simulink model "RB_KAIROS_impControl_repulsive"  (R2020b)
settings: Solver=ode4  StartTime=0.0  StopTime=t_end  FixedStep=Ts  RelTol=1e-3
values from neighbouring files (symbols this model uses):
  am = 0.3    [RB_KAIROS_ImpControl_OpSpace_quat_2020b_safety_main.m]
  am_r = 0.3    [RB_KAIROS_ImpControl_OpSpace_quat_2020b_safety_main.m]
  Kc = diag(50*ones(6,1))    [RB_KAIROS_ImpControl_OpSpace_quat_2020b_safety_main.m]
  Kp = 2*[400;400;400;400;0;0;0]    [RB_KAIROS_ImpControl_OpSpace_quat_2020b_safety_main.m]
  Kv = [1000;1000;1000;[300;300;300;300;300;300;300]]    [RB_KAIROS_ImpControl_OpSpace_quat_2020b_safety_main.m]
  model_sample_time = 0.001    [RB_KAIROS_ImpControl_OpSpace_quat_2020b_safety_main.m]
  q_dot_0 = zeros(10,1)    [RB_KAIROS_ImpControl_OpSpace_quat_2020b_safety_main.m]
  T_i = K    [RB_KAIROS_ImpControl_OpSpace_quat_2020b_safety_main.m]
  tau_ext = [0 0 0 0 0 0 0 0 0 0 0]    [RB_KAIROS_ImpControl_OpSpace_quat_2020b_safety_main.m]
  v_SMU = 10    [RB_KAIROS_ImpControl_OpSpace_quat_2020b_safety_main.m]
  vm = 0.5    [RB_KAIROS_ImpControl_OpSpace_quat_2020b_safety_main.m]
  vm_r = 0.5    [RB_KAIROS_ImpControl_OpSpace_quat_2020b_safety_main.m]
undefined symbols (not defined in the file or in its folder): DiscIntNeverNeededParam, magnitude, q_0, T_f
libraries: simulink x4, utils x4, transformations_lib x3
(part 3 of 17)

== matlab function RB_KAIROS_impControl_repulsive/CONTROLLER /Kinematics and Dynamics/Dynamics - Configuration space/Arm Coriolis//Centrifugal Matrix  ==
  data: qv input; C output; qa input; qdv input; qda input
function C = get_C(qv,qa,qdv,qda)
%GET_C
%    C = GET_C(qv,qa,qdv,qda)

%    This function was generated by the Symbolic Math Toolbox version 8.6.
%    14-Feb-2023 12:26:28

phi = qv(3);
phid = qdv(3);
q1 = qa(1);
q2 = qa(2);
q3 = qa(3);
q4 = qa(4);
q5 = qa(5);
q6 = qa(6);
q7 = qa(7);
q1d = qda(1);
q2d = qda(2);
q3d = qda(3);
q4d = qda(4);
q5d = qda(5);
q6d = qda(6);
q7d = qda(7);
xd = qdv(1);
yd = qdv(2);
t2 = cos(phi);
t3 = cos(q1);
t4 = cos(q2);
t5 = cos(q3);
t6 = cos(q4);
t7 = cos(q5);
t8 = cos(q6);
t9 = cos(q7);
t10 = sin(phi);
t11 = sin(q1);
t12 = sin(q2);
t13 = sin(q3);
t14 = sin(q4);
t15 = sin(q5);
t16 = sin(q6);
t17 = sin(q7);
t18 = t4.^2;
t19 = t5.^2;
t20 = t6.^2;
t21 = t7.^2;
t22 = t8.^2;
t23 = t9.^2;
t24 = t12.^2;
t25 = t13.^2;
t26 = t14.^2;
t27 = t15.^2;
t28 = t16.^2;
t29 = t17.^2;
t30 = t4.*t6;
t31 = t5.*t7;
t32 = t6.*t8;
t33 = t7.*t9;
t34 = t4.*t14;
t35 = t6.*t12;
t36 = t5.*t15;
t37 = t7.*t13;
t38 = t6.*t16;
t39 = t8.*t14;
t40 = t7.*t17;
t41 = t9.*t15;
t42 = t12.*t14;
t43 = t13.*t15;
t44 = t14.*t16;
t45 = t15.*t17;
t46 = -t10;
t82 = t7.*(1.1e+1./1.25e+2);
t83 = t6.*(4.8e+1./1.25e+2);
t84 = t7.*(4.8e+1./1.25e+2);
t85 = t4.*(3.3e+1./4.0e+2);
t86 = t5.*(3.3e+1./4.0e+2);
t87 = t6.*(3.3e+1./4.0e+2);
t88 = t7.*(3.3e+1./4.0e+2);
t89 = t8.*(3.3e+1./4.0e+2);
t90 = t15.*(1.1e+1./1.25e+2);
t91 = t14.*(4.8e+1./1.25e+2);
t92 = t15.*(4.8e+1./1.25e+2);
t93 = t12.*(3.3e+1./4.0e+2);
t94 = t13.*(3.3e+1./4.0e+2);
t95 = t14.*(3.3e+1./4.0e+2);
t96 = t15.*(3.3e+1./4.0e+2);
t97 = t16.*(3.3e+1./4.0e+2);
t121 = t5.*(7.9e+1./2.5e+2);
t125 = t13.*(7.9e+1./2.5e+2);
t132 = t8.*t9.*(1.1e+1./1.25e+2);
t146 = t8.*t17.*(1.1e+1./1.25e+2);
t147 = t9.*t16.*(1.1e+1./1.25e+2);
t163 = t16.*t17.*(1.1e+1./1.25e+2);
t179 = t5.*t6.*(-3.3e+1./4.0e+2);
t180 = t7.*t16.*(-4.8e+1./1.25e+2);
t181 = t8.*t15.*(-4.8e+1./1.25e+2);
t188 = t4.*t13.*(-3.3e+1./4.0e+2);
t189 = t5.*t12.*(-3.3e+1./4.0e+2);
t191 = t5.*t14.*(-3.3e+1./4.0e+2);
t192 = t6.*t13.*(-3.3e+1./4.0e+2);
t197 = t12.*t13.*(-3.3e+1./4.0e+2);
t198 = t13.*t14.*(-3.3e+1./4.0e+2);
t199 = t4.*2.872e-2;
t200 = t4.*3.925e-3;
t201 = t12.*2.872e-2;
t202 = t12.*3.925e-3;
t203 = t4.*t5.*(-7.9e+1./2.5e+2);
t204 = t5.*t6.*(-7.9e+1./2.5e+2);
t212 = t5.*t14.*(-7.9e+1./2.5e+2);
t213 = t13.*t14.*(-7.9e+1./2.5e+2);
t215 = t6.*1.9552e-2;
t216 = t5.*1.0442e-1;
t217 = t6.*1.0442e-1;
t219 = t14.*1.9552e-2;
t221 = t13.*1.0442e-1;
t222 = t14.*1.0442e-1;
t270 = t4.*1.083e-2;
t271 = t4.*2.811e-2;
t272 = t5.*5.317e-2;
t273 = t6.*5.317e-2;
t275 = t12.*1.083e-2;
t276 = t12.*2.811e-2;
t277 = t13.*5.317e-2;
t278 = t14.*5.317e-2;
t337 = t5.*t14.*(-1.9552e-2);
t364 = t5.*t12.*(-5.317e-2);
t366 = t5.*t14.*(-5.317e-2);
t367 = t12.*t13.*(-5.317e-2);
t368 = t13.*t14.*(-5.317e-2);
t566 = t13.*3.7242e-2;
t567 = t7.*2.9474e-2;
t569 = t15.*2.9474e-2;
t576 = t5.*3.7242e-2;
t587 = t9.*1.2516e-2;
t589 = t17.*1.2516e-2;
t606 = t8.*4.815e-3;
t607 = t7.*3.5549e-2;
t608 = t16.*4.815e-3;
t609 = t15.*3.5549e-2;
t610 = t5.*1.01140545e-1;
t611 = t7.*1.01140545e-1;
t612 = t13.*1.01140545e-1;
t613 = t15.*1.01140545e-1;
t621 = t12.*t13.*(-3.7242e-2);
t625 = t14.*4.1065e-2;
t626 = t15.*4.1065e-2;
t627 = t12.*7.962e-3;
t628 = t8.*4.354e-3;
t629 = t4.*1.2805e-2;
t630 = t5.*1.2805e-2;
t631 = t16.*4.354e-3;
t632 = t12.*1.2805e-2;
t633 = t13.*1.2805e-2;
t634 = t5.*2.8323e-2;
t635 = t13.*2.8323e-2;
t636 = t6.*8.626999999999999e-3;
t637 = t7.*5.433e-3;
t638 = t14.*8.626999999999999e-3;
t639 = t15.*5.433e-3;
t640 = t6.*2.5853e-2;
t643 = t14.*2.5853e-2;
t644 = t4.*2.7518e-2;
t645 = t5.*2.7518e-2;
t647 = t5.*3.6155e-2;
t648 = t12.*2.7518e-2;
t649 = t13.*2.7518e-2;
t650 = t7.*6.0149e-2;
t651 = t8.*6.0149e-2;
t652 = t13.*3.6155e-2;
t653 = t4.*3.9252e-2;
t654 = t5.*3.9252e-2;
t659 = t15.*6.0149e-2;
t660 = t16.*6.0149e-2;
t661 = t4.*1.1396e-2;
t662 = t5.*1.1396e-2;
t663 = t12.*3.9252e-2;
t664 = t13.*3.9252e-2;
t669 = t12.*1.1396e-2;
t670 = t13.*1.1396e-2;
t671 = t5.*8.640999999999999e-3;
t672 = t6.*8.640999999999999e-3;
t677 = t7.*6.3995712e-1;
t678 = t6.*4.1065e-2;
t679 = t7.*4.1065e-2;
t680 = t13.*8.640999999999999e-3;
t681 = t14.*8.640999999999999e-3;
t684 = t4.*7.962e-3;
t685 = t15.*6.3995712e-1;
t686 = t8.*1.196e-3;
t687 = t9.*1.196e-3;
t689 = t17.*4.28e-4;
t690 = t6.*7.796e-3;
t692 = t8.*1.0517e-2;
t693 = t9.*1.0517e-2;
t694 = t7.*2.117e-3;
t695 = t16.*1.196e-3;
t696 = t17.*1.196e-3;
t697 = t14.*7.796e-3;
t698 = t7.*t8.*2.82440448e-1;
t700 = t16.*1.0517e-2;
t701 = t17.*1.0517e-2;
t703 = t15.*2.117e-3;
t704 = t6.*4.037e-3;
t705 = t7.*4.037e-3;
t706 = t7.*6.4725936e-2;
t707 = t4.*3.495e-3;
t708 = t5.*t6.*3.87398936e-1;
t710 = t7.*t16.*2.82440448e-1;
t714 = t14.*4.037e-3;
t715 = t15.*4.037e-3;
t717 = t15.*6.4725936e-2;
t719 = t12.*3.495e-3;
t720 = t5.*t14.*3.87398936e-1;
t723 = t15.*t16.*2.82440448e-1;
t725 = t7.*1.158e-3;
t726 = t8.*1.158e-3;
t730 = t13.*t14.*3.87398936e-1;
t732 = t15.*1.158e-3;
t733 = t16.*1.158e-3;
t734 = t5.*1.332e-3;
t735 = t6.*1.332e-3;
t740 = t9.*1.0027e-2;
t742 = t13.*1.332e-3;
t743 = t14.*1.332e-3;
t751 = t17.*1.0027e-2;
t762 = t6.*t7.*3.8437e-2;
t764 = t6.*t15.*3.8437e-2;
t765 = t7.*t14.*3.8437e-2;
t766 = t14.*t15.*3.8437e-2;
t768 = t8.*1.964e-3;
t769 = t6.*1.1953e-2;
t770 = t7.*1.1953e-2;
t772 = t16.*1.964e-3;
t773 = t4.*3.141e-3;
t774 = t8.*4.252e-3;
t775 = t9.*4.252e-3;
t776 = t14.*1.1953e-2;
t777 = t15.*1.1953e-2;
t781 = t12.*3.141e-3;
t782 = t5.*4.761e-3;
t783 = t16.*4.252e-3;
t784 = t17.*4.252e-3;
t788 = t13.*4.761e-3;
t789 = t7.*1.4117e-2;
t790 = t8.*1.4117e-2;
t795 = t15.*1.4117e-2;
t796 = t16.*1.4117e-2;
t798 = t9.*4.28e-4;
t801 = t16.*t17.*(-1.2516e-2);
t804 = t8.*6.0680565e-2;
t805 = t7.*3.41e-4;
t806 = t8.*3.41e-4;
t813 = t16.*6.0680565e-2;
t817 = t15.*3.41e-4;
t818 = t16.*3.41e-4;
t830 = t8.*t9.*6.1597e-2;
t832 = t6.*2.29e-4;
t833 = t7.*2.29e-4;
t843 = t8.*t17.*6.1597e-2;
t844 = t9.*t16.*6.1597e-2;
t846 = t14.*2.29e-4;
t847 = t15.*2.29e-4;
t857 = t16.*t17.*6.1597e-2;
t862 = t7.*t16.*(-4.815e-3);
t866 = t5.*t6.*2.7454e-2;
t867 = t5.*t6.*(-1.01140545e-1);
t871 = t14.*t15.*(-3.5549e-2);
t874 = t5.*t14.*2.7454e-2;
t875 = t6.*t13.*2.7454e-2;
t876 = t5.*t14.*(-1.01140545e-1);
t877 = t6.*t13.*(-1.01140545e-1);
t883 = t13.*t14.*2.7454e-2;
t890 = t8.*7.41e-4;
t891 = t9.*7.41e-4;
t905 = t16.*7.41e-4;
t906 = t17.*7.41e-4;
t957 = t16.*1.09e-4;
t971 = t8.*t17.*6.4725936e-2;
t972 = t9.*t16.*6.4725936e-2;
t977 = t7.*t16.*(-4.354e-3);
t982 = t16.*t17.*6.4725936e-2;
t995 = t12.*t13.*(-1.2805e-2);
t999 = t4.*t13.*(-2.8323e-2);
t1004 = t7.*1.374907875e-1;
t1005 = t8.*1.374907875e-1;
t1018 = t12.*t13.*(-2.8323e-2);
t1023 = t15.*1.374907875e-1;
t1024 = t16.*1.374907875e-1;
t1026 = t6.*t13.*(-8.626999999999999e-3);
t1041 = t6.*t15.*(-5.433e-3);
t1048 = t14.*t15.*(-5.433e-3);
t1051 = t5.*t6.*(-2.5853e-2);
t1052 = t5.*1.13377482;
t1057 = t13.*1.13377482;
t1078 = t7.*t14.*(-6.0149e-2);
t1082 = t4.*t5.*(-1.1396e-2);
t1100 = t12.*t13.*(-3.9252e-2);
t1115 = t7.*t16.*(-6.3995712e-1);
t1116 = t8.*t15.*(-6.3995712e-1);
t1126 = t5.*t14.*(-4.1065e-2);
t1133 = t12.*t13.*(-8.640999999999999e-3);
t1140 = t4.*2.960013375e-1;
t1161 = t8.*1.09e-4;
t1166 = t12.*2.960013375e-1;
t1176 = t8.*t9.*6.4725936e-2;
t1179 = t16.*t17.*(-1.0517e-2);
t1184 = t14.*t15.*(-2.117e-3);
t1186 = t6.*t13.*(-4.037e-3);
t1194 = t14.*t15.*(-4.037e-3);
t1227 = t14.*t15.*(-1.158e-3);
t1229 = t15.*t16.*(-1.158e-3);
t1231 = t4.*t13.*(-1.332e-3);
t1243 = t13.*t14.*(-1.332e-3);
t1284 = t7.*t8.*(-1.964e-3);
t1297 = t6.*t15.*(-1.1953e-2);
t1303 = t13.*t14.*(-1.1953e-2);
t1304 = t14.*t15.*(-1.1953e-2);
t1312 = t7.*t8.*(-1.4117e-2);
t1325 = t12.*t13.*(-4.761e-3);
t1326 = t8.*t15.*(-1.4117e-2);
t1330 = t8.*t9.*(-1.196e-3);
t1337 = t7.*t16.*(-1.196e-3);
t1338 = t16.*t17.*(-4.28e-4);
t1340 = t6.*t13.*(-7.796e-3);
t1345 = t8.*t15.*(-1.0517e-2);
t1347 = t8.*t17.*(-1.0517e-2);
t1357 = t15.*t16.*(-1.196e-3);
t1358 = t13.*t14.*(-7.796e-3);
t1386 = t6.*t13.*(-2.29e-4);
t1423 = t4.*t5.*2.49498e-1;
t1429 = t8.*t15.*(-7.41e-4);
t1442 = t4.*t13.*2.49498e-1;
t1443 = t5.*t12.*2.49498e-1;
t1446 = t16.*t17.*(-7.41e-4);
t1460 = t12.*t13.*2.49498e-1;
t1496 = t5.*t6.*2.960013375e-1;
t1526 = t5.*t14.*2.960013375e-1;
t1527 = t6.*t13.*2.960013375e-1;
t1557 = t13.*t14.*2.960013375e-1;
t1594 = t6.*t15.*(-3.41e-4);
t1628 = t5.*t6.*(-1.13377482);
t1640 = t13.*t14.*(-1.13377482);
t1679 = t4.*1.857971472e-2;
t1700 = t12.*1.857971472e-2;
t1707 = t8.*t15.*(-1.09e-4);
t1724 = t15.*t16.*(-1.09e-4);
t1743 = t5.*1.9076837715e-1;
t1744 = t6.*1.9076837715e-1;
t1747 = t13.*1.9076837715e-1;
t1748 = t14.*1.9076837715e-1;
t1820 = t5.*3.746479959e-1;
t1821 = t6.*3.746479959e-1;
t1826 = t13.*3.746479959e-1;
t1827 = t14.*3.746479959e-1;
t1899 = t5.*t12.*(-1.9076837715e-1);
t1901 = t5.*t14.*(-1.9076837715e-1);
t1902 = t12.*t13.*(-1.9076837715e-1);
t1903 = t13.*t14.*(-1.9076837715e-1);
t2009 = t2.*1.224646799147353e-16;
t2024 = t10.*1.224646799147353e-16;
t2093 = t13.*t14.*4.5595633420575e-2;
t2162 = t6.*t13.*5.13251877947625e-2;
t2295 = t13.*3.879344917247175e-2;
t2385 = t5.*t12.*3.879344917247175e-2;
t2411 = t4.*t13.*(-3.879344917247175e-2);
t2712 = t4.*8.8844724872e-2;
t2713 = t5.*8.8844724872e-2;
t2715 = t12.*8.8844724872e-2;
t2716 = t13.*8.8844724872e-2;
t2720 = t4.*1.26729164208e-1;
t2721 = t5.*1.26729164208e-1;
t2722 = t12.*1.26729164208e-1;
t2723 = t13.*1.26729164208e-1;
t2725 = t6.*5.034347249e-2;
t2726 = t7.*5.034347249e-2;
t2727 = t6.*t7.*4.7121686402e-2;
t2728 = t14.*5.034347249e-2;
t2729 = t15.*5.034347249e-2;
t2730 = t6.*t15.*4.7121686402e-2;
t2731 = t7.*t14.*4.7121686402e-2;
t2733 = t14.*t15.*4.7121686402e-2;
t2743 = t6.*1.4653732538e-2;
t2744 = t7.*1.4653732538e-2;
t2747 = t14.*1.4653732538e-2;
t2748 = t15.*1.4653732538e-2;
t2761 = t7.*2.3526756935e-2;
t2762 = t8.*2.3526756935e-2;
t2765 = t15.*2.3526756935e-2;
t2766 = t16.*2.3526756935e-2;
t2768 = t8.*3.127439544e-3;
t2769 = t9.*3.127439544e-3;
t2771 = t16.*3.127439544e-3;
t2772 = t17.*3.127439544e-3;
t2774 = t8.*7.735484874e-3;
t2775 = t9.*7.735484874e-3;
t2777 = t16.*7.735484874e-3;
t2778 = t17.*7.735484874e-3;
t2781 = t7.*1.00241616695e-1;
t2782 = t8.*1.00241616695e-1;
t2784 = t15.*1.00241616695e-1;
t2785 = t16.*1.00241616695e-1;
t2788 = t12.*2.26100637e-3;
t2795 = t5.*t6.*9.850206933e-2;
t2801 = t5.*t14.*9.850206933e-2;
t2802 = t6.*t13.*9.850206933e-2;
t2806 = t13.*t14.*9.850206933e-2;
t2836 = t8.*t9.*4.5305948634e-2;
t2840 = t8.*t17.*4.5305948634e-2;
t2841 = t9.*t16.*4.5305948634e-2;
t2842 = t4.*2.031994566e-3;
t2845 = t16.*t17.*4.5305948634e-2;
t2846 = t12.*2.031994566e-3;
t2849 = t4.*2.26100637e-3;
t2868 = t12.*t13.*(-1.26729164208e-1);
t2877 = t7.*t8.*1.7527158935e-2;
t2892 = t7.*t16.*1.7527158935e-2;
t2893 = t8.*t15.*1.7527158935e-2;
t2908 = t15.*t16.*1.7527158935e-2;
t2911 = t5.*t14.*(-5.034347249e-2);
t2953 = t15.*t16.*1.924639040544e-2;
t2954 = t3.*2.75e-1;
t2958 = t6.*t15.*(-1.4653732538e-2);
t2959 = t11.*2.75e-1;
t2963 = t9.*t16.*3.40361334456e-4;
t2964 = t13.*t14.*(-1.4653732538e-2);
t2965 = t14.*t15.*(-1.4653732538e-2);
t2967 = t3.*1.55e-1;
t2972 = t11.*1.55e-1;
t2979 = t7.*t8.*(-2.3526756935e-2);
t2985 = t8.*t15.*(-2.3526756935e-2);
t3001 = t8.*t17.*(-7.735484874e-3);
t3004 = t16.*t17.*(-7.735484874e-3);
t3010 = t7.*t14.*(-1.00241616695e-1);
t3019 = t8.*t15.*4.51713733152e-3;
t3105 = t4.*t5.*8.055302407919999e-1;
t3112 = t4.*t13.*8.055302407919999e-1;
t3113 = t5.*t12.*8.055302407919999e-1;
t3122 = t12.*t13.*8.055302407919999e-1;
t3167 = t16.*t17.*1.37607339936e-4;
t3273 = t5.*t14.*8.222930397193003e-4;
t3281 = t12.*7.689361029464e-4;
t3298 = t5.*t6.*1.95267751313805e-3;
t4017 = t3.*7.704560200000002e-1;
t4019 = t11.*7.704560200000002e-1;
t4041 = t6.*t15.*1.082026026049065e-3;
t4044 = t3.*1.3669381;
t4047 = t11.*1.3669381;
t4049 = t3.*1.0027353e-1;
t4051 = t6.*t7.*2.300122758781553e-3;
t4052 = t11.*1.0027353e-1;
t4063 = t3.*1.7790465e-1;
t4066 = t11.*1.7790465e-1;
t4071 = t8.*t9.*8.36241330891889e-4;
t4072 = t5.*t12.*4.442367301156758e-2;
t4080 = t8.*t17.*2.74179553204116e-4;
t4084 = t7.*t8.*5.187945860934245e-5;
t4092 = t7.*t16.*4.67845486573025e-5;
t4095 = t4.*t13.*2.221183650578379e-2;
t4096 = t14.*5.434755381414281e-3;
t4110 = t15.*5.897280115119475e-3;
t4115 = t4.*t5.*1.678129058305713e-2;
t4121 = t12.*t13.*3.356258116611425e-2;
t4130 = t16.*2.454825983680473e-3;
t4157 = t6.*t13.*5.434755381414281e-3;
t4177 = t7.*t14.*5.897280115119475e-3;
t4178 = t4.*1.026110182100817e-2;
t4189 = t8.*t15.*2.454825983680473e-3;
t4195 = t5.*t14.*(-5.434755381414281e-3);
t4207 = t6.*t15.*(-5.897280115119475e-3);
t4221 = t7.*t16.*(-2.454825983680473e-3);
t4241 = t12.*9.124601146260056e-3;
t47 = t12.*t43;
t48 = t13.*t44;
t49 = t14.*t45;
t50 = t5.*t30;
t51 = t6.*t31;
t52 = t7.*t32;
t53 = t8.*t33;
t54 = t5.*t34;
t55 = t5.*t35;
t56 = t4.*t37;
t57 = t12.*t31;
t58 = t6.*t36;
t59 = t6.*t37;
t60 = t5.*t39;
t61 = t13.*t32;
t62 = t7.*t38;
t63 = t7.*t39;
t64 = t6.*t41;
t65 = t14.*t33;
t66 = t8.*t40;
t67 = t8.*t41;
t68 = t5.*t42;
t69 = t4.*t43;
t70 = t12.*t36;
t71 = t12.*t37;
t72 = t6.*t43;
t73 = t5.*t44;
t74 = t13.*t38;
t75 = t13.*t39;
t76 = t7.*t44;
t77 = t6.*t45;
t78 = t14.*t40;
t79 = t14.*t41;
t80 = t8.*t45;
t98 = t35.*t37;
t99 = t37.*t39;
t100 = t39.*t41;
t103 = t35.*t43;
t105 = t37.*t44;
t107 = t39.*t45;
t113 = t13.*t16.*t42;
t114 = t14.*t17.*t43;
t122 = -t86;
t123 = -t88;
t124 = -t89;
t126 = -t93;
t127 = -t94;
t128 = -t95;
t129 = -t96;
t130 = t31.*(1.1e+1./1.25e+2);
t131 = t32.*(1.1e+1./1.25e+2);
t133 = t30.*(4.8e+1./1.25e+2);
t134 = t5.*t83;
t135 = t31.*(4.8e+1./1.25e+2);
t136 = t8.*t84;
t137 = t33.*(4.8e+1./1.25e+2);
t138 = t30.*(3.3e+1./4.0e+2);
t139 = t6.*t86;
t140 = t36.*(1.1e+1./1.25e+2);
t141 = t37.*(1.1e+1./1.25e+2);
t142 = t6.*t90;
t143 = t14.*t82;
t144 = t38.*(1.1e+1./1.25e+2);
t145 = t39.*(1.1e+1./1.25e+2);
t148 = t34.*(4.8e+1./1.25e+2);
t149 = t13.*t83;
t150 = t36.*(4.8e+1./1.25e+2);
t151 = t37.*(4.8e+1./1.25e+2);
t152 = t16.*t84;
t153 = t8.*t92;
t154 = t40.*(4.8e+1./1.25e+2);
t155 = t41.*(4.8e+1./1.25e+2);
t156 = t13.*t85;
t157 = t12.*t86;
t158 = t34.*(3.3e+1./4.0e+2);
t159 = t35.*(3.3e+1./4.0e+2);
t160 = t14.*t86;
t161 = t13.*t87;
t162 = t14.*t90;
t164 = t42.*(4.8e+1./1.25e+2);
t165 = t13.*t91;
t166 = t43.*(4.8e+1./1.25e+2);
t167 = t16.*t92;
t168 = t45.*(4.8e+1./1.25e+2);
t169 = t13.*t93;
t170 = t14.*t94;
t176 = t4.*t121;
t177 = t6.*t121;
t178 = t31.*(7.9e+1./2.5e+2);
t182 = t4.*t125;
t183 = t12.*t121;
t184 = t14.*t121;
t185 = t6.*t125;
t186 = t36.*(7.9e+1./2.5e+2);
t187 = t37.*(7.9e+1./2.5e+2);
t194 = t12.*t125;
t195 = t14.*t125;
t196 = t43.*(7.9e+1./2.5e+2);
t207 = t14.*t43.*(1.1e+1./1.25e+2);
t209 = t16.*t45.*(1.1e+1./1.25e+2);
t211 = t42.*t94;
t218 = -t201;
t220 = -t202;
t240 = t16.*t33.*(1.1e+1./1.25e+2);
t247 = t30.*t94;
t253 = t16.*t40.*(1.1e+1./1.25e+2);
t255 = t16.*t41.*(1.1e+1./1.25e+2);
t257 = t13.*t35.*(4.8e+1./1.25e+2);
t262 = t34.*t94;
t264 = t35.*t94;
t267 = t42.*t125;
t269 = t13.*t42.*(-3.3e+1./4.0e+2);
t274 = -t219;
t282 = t30.*t125;
t285 = t13.*t30.*(-3.3e+1./4.0e+2);
t293 = t34.*t125;
t295 = t35.*t125;
t297 = t13.*t34.*(-3.3e+1./4.0e+2);
t299 = t13.*t35.*(-3.3e+1./4.0e+2);
t300 = t30.*1.9552e-2;
t301 = t30.*1.0442e-1;
t302 = t6.*t216;
t303 = t13.*t42.*(-7.9e+1./2.5e+2);
t305 = t34.*1.9552e-2;
t306 = t35.*1.9552e-2;
t307 = t5.*t219;
t308 = t13.*t215;
t309 = t4.*t221;
t310 = t12.*t216;
t311 = t34.*1.0442e-1;
t312 = t13.*t217;
t313 = t13.*t219;
t314 = t12.*t221;
t315 = t42.*1.0442e-1;
t316 = t14.*t221;
t317 = -t272;
t318 = -t278;
t330 = t41.*t44.*(1.1e+1./1.25e+2);
t331 = t44.*t45.*(1.1e+1./1.25e+2);
t332 = t13.*t34.*(-7.9e+1./2.5e+2);
t334 = t13.*t35.*(-7.9e+1./2.5e+2);
t335 = t30.*5.317e-2;
t339 = t4.*t277;
t340 = t12.*t272;
t341 = t34.*5.317e-2;
t342 = t35.*5.317e-2;
t343 = t14.*t272;
t344 = t13.*t273;
t345 = t12.*t277;
t346 = t14.*t277;
t363 = t13.*t42.*1.9552e-2;
t378 = t35.*t221;
t379 = t42.*t277;
t402 = t13.*t42.*(-5.317e-2);
t406 = t87+t91;
t432 = t89+t180;
t438 = t93+t203;
t494 = t200+t276;
t577 = -t566;
t583 = t222+t273-3.3e+1./4.0e+2;
t588 = t14.*t569;
t590 = t4.*t576;
t591 = t12.*t576;
t592 = t31.*2.9474e-2;
t593 = t12.*t566;
t594 = t36.*2.9474e-2;
t595 = t37.*2.9474e-2;
t596 = t6.*t569;
t597 = t14.*t567;
t601 = -t589;
t641 = -t609;
t642 = -t611;
t646 = -t613;
t665 = t33.*1.2516e-2;
t666 = t8.*t587;
t673 = t40.*1.2516e-2;
t674 = t16.*t587;
t676 = t14.*t43.*2.9474e-2;
t682 = t45.*1.2516e-2;
t683 = t16.*t589;
t691 = -t627;
t699 = t33.*2.82440448e-1;
t709 = t31.*3.87398936e-1;
t711 = t40.*2.82440448e-1;
t712 = t41.*2.82440448e-1;
t716 = -t629;
t721 = t36.*3.87398936e-1;
t722 = t37.*3.87398936e-1;
t724 = t45.*2.82440448e-1;
t727 = -t631;
t728 = -t633;
t731 = t43.*3.87398936e-1;
t736 = t32.*4.815e-3;
t737 = t31.*3.5549e-2;
t738 = t6.*t607;
t739 = -t635;
t741 = -t636;
t744 = t38.*4.815e-3;
t745 = t39.*4.815e-3;
t746 = t7.*t608;
t747 = t15.*t606;
t748 = t36.*3.5549e-2;
t749 = t14.*t607;
t750 = t6.*t610;
t752 = t15.*t608;
t755 = t43.*3.5549e-2;
t756 = t14.*t609;
t757 = t4.*t612;
t758 = t12.*t610;
t759 = t14.*t610;
t760 = t6.*t612;
t761 = -t639;
t763 = t12.*t612;
t780 = -t660;
t785 = -t664;
t791 = -t669;
t802 = -t689;
t803 = t32.*4.354e-3;
t807 = -t695;
t808 = -t697;
t809 = t38.*4.354e-3;
t810 = t39.*4.354e-3;
t811 = t7.*t631;
t812 = t15.*t628;
t814 = t13.*t629;
t815 = t12.*t630;
t816 = -t701;
t819 = -t703;
t820 = -t704;
t821 = t15.*t631;
t822 = t13.*t632;
t825 = t4.*t635;
t826 = t12.*t634;
t827 = -t715;
t828 = t30.*8.626999999999999e-3;
t829 = t33.*6.1597e-2;
t834 = -t720;
t835 = t12.*t635;
t836 = t31.*5.433e-3;
t837 = t34.*8.626999999999999e-3;
t838 = t35.*8.626999999999999e-3;
t839 = t5.*t638;
t840 = t13.*t636;
t841 = t40.*6.1597e-2;
t842 = t41.*6.1597e-2;
t848 = -t730;
t850 = -t733;
t851 = t36.*5.433e-3;
t852 = t37.*5.433e-3;
t853 = t6.*t639;
t854 = t14.*t637;
t855 = t13.*t638;
t856 = t45.*6.1597e-2;
t858 = -t743;
t861 = t14.*t639;
t863 = t30.*2.5853e-2;
t864 = t5.*t640;
t865 = t30.*2.7454e-2;
t868 = t34.*2.5853e-2;
t869 = t13.*t640;
t872 = t34.*2.7454e-2;
t873 = t35.*2.7454e-2;
t878 = t42.*2.5853e-2;
t879 = t13.*t643;
t880 = t13.*t644;
t881 = t12.*t645;
t882 = t42.*2.7454e-2;
t884 = -t765;
t885 = t31.*6.0149e-2;
t886 = t32.*6.0149e-2;
t888 = t4.*t652;
t889 = t12.*t647;
t892 = t13.*t648;
t893 = t5.*t653;
t894 = -t766;
t895 = t36.*6.0149e-2;
t896 = t37.*6.0149e-2;
t897 = t6.*t659;
t898 = t14.*t650;
t899 = t38.*6.0149e-2;
t900 = t39.*6.0149e-2;
t901 = t16.*t650;
t902 = t15.*t651;
t903 = t12.*t652;
t904 = t5.*t661;
t907 = t12.*t654;
t909 = t14.*t659;
t910 = t16.*t659;
t911 = t12.*t662;
t912 = t13.*t663;
t913 = t30.*8.640999999999999e-3;
t914 = -t773;
t917 = t31.*6.3995712e-1;
t918 = t8.*t677;
t919 = -t777;
t920 = t13.*t669;
t921 = t30.*4.1065e-2;
t922 = t31.*4.1065e-2;
t923 = t7.*t678;
t924 = t4.*t680;
t925 = t12.*t671;
t926 = t34.*8.640999999999999e-3;
t927 = t35.*8.640999999999999e-3;
t928 = t14.*t671;
t929 = t13.*t672;
t934 = t16.*t41.*1.2516e-2;
t935 = t36.*6.3995712e-1;
t936 = t16.*t677;
t937 = t8.*t685;
t938 = t34.*4.1065e-2;
t939 = t35.*4.1065e-2;
t940 = t5.*t625;
t941 = t13.*t678;
t942 = t36.*4.1065e-2;
t943 = t7.*t625;
t944 = t12.*t680;
t945 = t14.*t680;
t947 = -t788;
t948 = -t789;
t949 = t43.*6.3995712e-1;
t950 = t16.*t685;
t951 = t13.*t625;
t952 = t43.*4.1065e-2;
t953 = t15.*t625;
t954 = t44.*1.0517e-2;
t955 = t15.*t700;
t956 = t17.*t700;
t958 = t43.*2.117e-3;
t959 = t14.*t703;
t960 = -t804;
t961 = t34.*4.037e-3;
t962 = t35.*4.037e-3;
t963 = t5.*t714;
t964 = t13.*t704;
t965 = t36.*4.037e-3;
t966 = t14.*t705;
t967 = t36.*6.4725936e-2;
t968 = t37.*6.4725936e-2;
t969 = t6.*t717;
t970 = t14.*t706;
t974 = t31.*1.158e-3;
t975 = t32.*1.158e-3;
t976 = t8.*t725;
t978 = t13.*t714;
t979 = t43.*4.037e-3;
t980 = t15.*t714;
t981 = t14.*t717;
t983 = t13.*t34.*3.87398936e-1;
t985 = t13.*t35.*3.87398936e-1;
t987 = t36.*1.158e-3;
t988 = t37.*1.158e-3;
t989 = t6.*t732;
t990 = t14.*t725;
t991 = t38.*1.158e-3;
t992 = t15.*t726;
t993 = t30.*1.332e-3;
t994 = t6.*t734;
t997 = t13.*t42.*3.87398936e-1;
t1000 = t14.*t732;
t1001 = t44.*1.158e-3;
t1002 = t16.*t732;
t1003 = t33.*1.0027e-2;
t1006 = t4.*t742;
t1007 = t12.*t734;
t1008 = t34.*1.332e-3;
t1009 = t13.*t735;
t1011 = -t830;
t1016 = -t832;
t1019 = t40.*1.0027e-2;
t1020 = t41.*1.0027e-2;
t1021 = t8.*t751;
t1022 = t16.*t740;
t1027 = t12.*t742;
t1028 = t42.*1.332e-3;
t1029 = t14.*t742;
t1030 = -t843;
t1037 = t14.*t37.*3.5549e-2;
t1038 = t30.*t612;
t1040 = t16.*t751;
t1045 = t15.*t44.*4.815e-3;
t1047 = t35.*t612;
t1053 = t42.*t612;
t1055 = t14.*t37.*3.8437e-2;
t1058 = t32.*1.964e-3;
t1059 = t7.*t768;
t1060 = t14.*t43.*3.8437e-2;
t1061 = -t883;
t1062 = t30.*1.1953e-2;
t1063 = t31.*1.1953e-2;
t1064 = t38.*1.964e-3;
t1065 = t15.*t768;
t1066 = -t890;
t1067 = t32.*4.252e-3;
t1068 = t33.*4.252e-3;
t1069 = t9.*t774;
t1070 = t34.*1.1953e-2;
t1071 = t35.*1.1953e-2;
t1072 = t5.*t776;
t1073 = t13.*t769;
t1074 = t36.*1.1953e-2;
t1075 = t37.*1.1953e-2;
t1076 = t15.*t769;
t1077 = t14.*t770;
t1079 = t44.*1.964e-3;
t1080 = t15.*t772;
t1081 = t4.*t782;
t1083 = -t906;
t1084 = t38.*4.252e-3;
t1085 = t39.*4.252e-3;
t1086 = t7.*t783;
t1087 = t15.*t774;
t1088 = t40.*4.252e-3;
t1089 = t16.*t775;
t1090 = t13.*t776;
t1091 = t15.*t776;
t1092 = t4.*t788;
t1093 = t12.*t782;
t1094 = t31.*1.4117e-2;
t1095 = t32.*1.4117e-2;
t1096 = t8.*t789;
t1097 = t15.*t783;
t1098 = t45.*4.252e-3;
t1099 = t17.*t783;
t1101 = t12.*t788;
t1102 = t36.*1.4117e-2;
t1103 = t37.*1.4117e-2;
t1104 = t6.*t795;
t1105 = t14.*t789;
t1106 = t38.*1.4117e-2;
t1107 = t15.*t790;
t1110 = t33.*4.28e-4;
t1111 = t8.*t798;
t1117 = t14.*t795;
t1118 = t44.*1.4117e-2;
t1119 = t16.*t795;
t1120 = t32.*1.196e-3;
t1121 = t33.*1.196e-3;
t1122 = t9.*t686;
t1127 = t40.*4.28e-4;
t1128 = t41.*4.28e-4;
t1129 = t8.*t689;
t1130 = t16.*t798;
t1131 = t30.*7.796e-3;
t1132 = t5.*t690;
t1134 = t32.*1.0517e-2;
t1135 = t7.*t692;
t1136 = t33.*1.0517e-2;
t1138 = t31.*2.117e-3;
t1139 = t6.*t694;
t1141 = t38.*1.196e-3;
t1142 = t39.*1.196e-3;
t1143 = t7.*t695;
t1144 = t15.*t686;
t1145 = t40.*1.196e-3;
t1146 = t16.*t687;
t1147 = t45.*4.28e-4;
t1148 = t16.*t689;
t1149 = t34.*7.796e-3;
t1150 = t35.*7.796e-3;
t1151 = t5.*t697;
t1152 = t13.*t690;
t1153 = t38.*1.0517e-2;
t1154 = t39.*1.0517e-2;
t1155 = t7.*t700;
t1156 = t15.*t692;
t1157 = t40.*1.0517e-2;
t1158 = t41.*1.0517e-2;
t1159 = t17.*t692;
t1160 = t16.*t693;
t1162 = t36.*2.117e-3;
t1163 = t37.*2.117e-3;
t1164 = t6.*t703;
t1165 = t14.*t694;
t1167 = t15.*t695;
t1168 = t45.*1.196e-3;
t1169 = t17.*t695;
t1170 = t30.*4.037e-3;
t1171 = t31.*4.037e-3;
t1172 = t7.*t704;
t1173 = t42.*7.796e-3;
t1174 = t13.*t697;
t1175 = t31.*6.4725936e-2;
t1180 = t14.*t817;
t1181 = t16.*t817;
t1182 = -t957;
t1189 = t15.*t44.*4.354e-3;
t1190 = t30.*2.29e-4;
t1191 = t31.*2.29e-4;
t1201 = t34.*2.29e-4;
t1202 = t35.*2.29e-4;
t1203 = t5.*t846;
t1204 = t13.*t832;
t1205 = t36.*2.29e-4;
t1206 = t37.*2.29e-4;
t1207 = t15.*t832;
t1208 = t14.*t833;
t1223 = t13.*t846;
t1224 = t15.*t846;
t1230 = -t1005;
t1235 = t13.*t42.*8.626999999999999e-3;
t1245 = t14.*t43.*5.433e-3;
t1252 = t13.*t30.*(-1.01140545e-1);
t1256 = t13.*t35.*2.5853e-2;
t1260 = t13.*t35.*(-1.01140545e-1);
t1263 = t32.*7.41e-4;
t1264 = t33.*7.41e-4;
t1275 = t38.*7.41e-4;
t1276 = t39.*7.41e-4;
t1277 = t7.*t905;
t1278 = t15.*t890;
t1279 = t40.*7.41e-4;
t1280 = t41.*7.41e-4;
t1281 = t17.*t890;
t1282 = t16.*t891;
t1290 = t15.*t905;
t1291 = t17.*t905;
t1293 = t14.*t43.*6.0149e-2;
t1295 = t44.*t659;
t1322 = t37.*t625;
t1323 = t42.*t680;
t1328 = t13.*t42.*4.1065e-2;
t1334 = t31.*3.41e-4;
t1335 = t32.*3.41e-4;
t1348 = t36.*3.41e-4;
t1349 = t37.*3.41e-4;
t1350 = t6.*t817;
t1351 = t14.*t805;
t1352 = t38.*3.41e-4;
t1353 = t39.*3.41e-4;
t1354 = t16.*t805;
t1355 = t15.*t806;
t1356 = -t1166;
t1368 = t39.*t732;
t1374 = t14.*t43.*1.158e-3;
t1382 = t35.*t742;
t1397 = t16.*t45.*1.0027e-2;
t1399 = t4.*t1052;
t1400 = t6.*t1052;
t1405 = t12.*t1052;
t1406 = t14.*t1052;
t1407 = t6.*t1057;
t1410 = t12.*t1057;
t1411 = t14.*t1057;
t1415 = t13.*t42.*(-2.7454e-2);
t1428 = t15.*t39.*1.964e-3;
t1453 = t41.*t783;
t1454 = t13.*t42.*1.1953e-2;
t1456 = t43.*t776;
t1459 = t15.*t44.*(-6.0149e-2);
t1469 = t15.*t44.*4.252e-3;
t1482 = t39.*t795;
t1493 = t14.*t43.*1.4117e-2;
t1519 = t32.*1.09e-4;
t1520 = t7.*t1161;
t1534 = t41.*t695;
t1548 = t38.*1.09e-4;
t1549 = t39.*1.09e-4;
t1550 = t7.*t957;
t1551 = t15.*t1161;
t1559 = t15.*t44.*1.196e-3;
t1569 = t16.*t33.*6.4725936e-2;
t1577 = t45.*t700;
t1578 = t44.*1.09e-4;
t1579 = t15.*t957;
t1588 = t37.*t714;
t1591 = t16.*t40.*6.4725936e-2;
t1593 = t16.*t41.*6.4725936e-2;
t1602 = t13.*t42.*4.037e-3;
t1605 = t14.*t43.*6.4725936e-2;
t1606 = t16.*t45.*6.4725936e-2;
t1613 = t13.*t42.*2.29e-4;
t1615 = t43.*t846;
t1624 = t31.*3.45563e-1;
t1626 = t36.*3.45563e-1;
t1627 = t37.*3.45563e-1;
t1630 = t43.*3.45563e-1;
t1650 = t15.*t44.*7.41e-4;
t1652 = t45.*t905;
t1653 = -t1423;
t1657 = t31.*5.2663138e-1;
t1662 = t14.*t43.*(-1.1953e-2);
t1664 = t37.*5.2663138e-1;
t1665 = -t1460;
t1669 = t43.*5.2663138e-1;
t1693 = -t1526;
t1694 = -t1527;
t1699 = t13.*t35.*(-7.796e-3);
t1710 = -t1557;
t1714 = t13.*t42.*(-7.796e-3);
t1718 = t15.*t44.*(-1.0517e-2);
t1719 = t16.*t45.*(-1.0517e-2);
t1721 = t14.*t43.*3.41e-4;
t1723 = t44.*t817;
t1745 = t30.*t1057;
t1749 = t34.*t1057;
t1751 = t35.*t1057;
t1752 = t42.*t1057;
t1762 = t16.*t45.*(-7.41e-4);
t1771 = t13.*t30.*2.960013375e-1;
t1785 = t13.*t34.*2.960013375e-1;
t1787 = t13.*t35.*2.960013375e-1;
t1801 = t13.*t42.*2.960013375e-1;
t1810 = -t1700;
t1812 = t41.*t44.*6.4725936e-2;
t1817 = t44.*t45.*6.4725936e-2;
t1832 = -t1743;
t1836 = -t1748;
t1839 = t13.*t34.*(-1.13377482);
t1863 = t15.*t39.*(-1.09e-4);
t1866 = t15.*t44.*(-1.09e-4);
t1871 = t4.*t1747;
t1872 = t12.*t1743;
t1873 = t34.*1.9076837715e-1;
t1874 = t35.*1.9076837715e-1;
t1875 = t14.*t1743;
t1876 = t13.*t1744;
t1878 = t12.*t1747;
t1879 = t14.*t1747;
t1889 = t30.*3.746479959e-1;
t1890 = t6.*t1820;
t1891 = t4.*t1826;
t1892 = t12.*t1820;
t1893 = t34.*3.746479959e-1;
t1894 = t13.*t1821;
t1895 = t12.*t1826;
t1896 = t42.*3.746479959e-1;
t1897 = t14.*t1826;
t1898 = t30.*1.9076837715e-1;
t1924 = t35.*t1826;
t1928 = t42.*t1747;
t1949 = t13.*t42.*(-1.9076837715e-1);
t1970 = t202+t684;
t2008 = t199+t781;
t2044 = t132+t844;
t2054 = t146+t857;
t2111 = t215+t697;
t2175 = t13.*t30.*7.8691955574375e-3;
t2193 = -t2093;
t2228 = t13.*t34.*1.5454229830875e-2;
t2254 = t13.*t34.*4.5595633420575e-2;
t2297 = t2+t2024;
t2320 = t13.*t30.*5.13251877947625e-2;
t2384 = t4.*t2295;
t2396 = t46+t2009;
t2755 = -t2723;
t2779 = -t2731;
t2780 = -t2733;
t2787 = t13.*t2715;
t2792 = t5.*t2720;
t2793 = t12.*t2721;
t2794 = t30.*9.850206933e-2;
t2797 = -t2748;
t2798 = t13.*t2722;
t2799 = t34.*9.850206933e-2;
t2800 = t35.*9.850206933e-2;
t2805 = t42.*9.850206933e-2;
t2810 = t30.*5.034347249e-2;
t2811 = t31.*5.034347249e-2;
t2812 = t7.*t2725;
t2813 = -t2761;
t2816 = t34.*5.034347249e-2;
t2817 = t35.*5.034347249e-2;
t2818 = t5.*t2728;
t2819 = t13.*t2725;
t2820 = t36.*5.034347249e-2;
t2821 = t14.*t2726;
t2825 = t13.*t2728;
t2826 = t43.*5.034347249e-2;
t2827 = t15.*t2728;
t2829 = t14.*t37.*4.7121686402e-2;
t2832 = t14.*t43.*4.7121686402e-2;
t2834 = -t2778;
t2835 = t33.*4.5305948634e-2;
t2838 = t40.*4.5305948634e-2;
t2839 = t41.*4.5305948634e-2;
t2843 = -t2785;
t2844 = t45.*4.5305948634e-2;
t2847 = t13.*t2712;
t2848 = t12.*t2713;
t2851 = t30.*1.4653732538e-2;
t2852 = t31.*1.4653732538e-2;
t2854 = t34.*1.4653732538e-2;
t2855 = t35.*1.4653732538e-2;
t2856 = t5.*t2747;
t2857 = t13.*t2743;
t2858 = t36.*1.4653732538e-2;
t2859 = t37.*1.4653732538e-2;
t2860 = t15.*t2743;
t2861 = t14.*t2744;
t2863 = t13.*t2747;
t2864 = t15.*t2747;
t2870 = t33.*1.485213095808e-3;
t2872 = t31.*2.3526756935e-2;
t2873 = t32.*2.3526756935e-2;
t2874 = t8.*t2761;
t2875 = -t2806;
t2876 = t32.*1.7527158935e-2;
t2878 = t36.*2.3526756935e-2;
t2879 = t37.*2.3526756935e-2;
t2880 = t6.*t2765;
t2881 = t14.*t2761;
t2882 = t38.*2.3526756935e-2;
t2883 = t15.*t2762;
t2887 = t32.*3.127439544e-3;
t2888 = t33.*3.127439544e-3;
t2889 = t9.*t2768;
t2890 = t38.*1.7527158935e-2;
t2891 = t39.*1.7527158935e-2;
t2895 = t14.*t2765;
t2896 = t44.*2.3526756935e-2;
t2897 = t16.*t2765;
t2899 = t38.*3.127439544e-3;
t2900 = t39.*3.127439544e-3;
t2901 = t7.*t2771;
t2902 = t15.*t2768;
t2903 = t40.*3.127439544e-3;
t2904 = t16.*t2769;
t2905 = t32.*7.735484874e-3;
t2906 = t33.*7.735484874e-3;
t2907 = t44.*1.7527158935e-2;
t2912 = t15.*t2771;
t2913 = t45.*3.127439544e-3;
t2914 = t17.*t2771;
t2915 = t38.*7.735484874e-3;
t2916 = t39.*7.735484874e-3;
t2917 = t7.*t2777;
t2918 = t15.*t2774;
t2919 = t40.*7.735484874e-3;
t2920 = t41.*7.735484874e-3;
t2921 = t17.*t2774;
t2922 = t16.*t2775;
t2926 = t15.*t2777;
t2927 = t17.*t2777;
t2930 = t31.*1.00241616695e-1;
t2931 = t32.*1.00241616695e-1;
t2934 = t36.*1.00241616695e-1;
t2935 = t37.*1.00241616695e-1;
t2936 = t6.*t2784;
t2937 = t14.*t2781;
t2938 = t38.*1.00241616695e-1;
t2939 = t39.*1.00241616695e-1;
t2940 = t16.*t2781;
t2941 = t15.*t2782;
t2942 = t31.*4.23641577598e-1;
t2943 = t14.*t2784;
t2944 = t16.*t2784;
t2946 = -t2836;
t2947 = t36.*4.23641577598e-1;
t2948 = t37.*4.23641577598e-1;
t2949 = -t2840;
t2950 = -t2842;
t2951 = t43.*4.23641577598e-1;
t2955 = t36.*7.954268653419999e-3;
t2968 = t31.*2.315289741004e-3;
t2974 = t40.*6.00468392448e-4;
t2993 = t37.*t2728;
t2994 = -t2893;
t2996 = t13.*t42.*5.034347249e-2;
t3018 = -t2953;
t3020 = t13.*t42.*1.4653732538e-2;
t3022 = t43.*t2747;
t3024 = -t2959;
t3026 = -t2963;
t3030 = t576+t788;
t3037 = t13.*t42.*(-9.850206933e-2);
t3051 = t39.*t2765;
t3064 = t14.*t43.*2.3526756935e-2;
t3073 = t41.*t2771;
t3086 = t15.*t44.*3.127439544e-3;
t3094 = t15.*t44.*7.735484874e-3;
t3096 = t45.*t2777;
t3106 = t569+t694;
t3117 = t14.*t43.*1.00241616695e-1;
t3119 = t44.*t2784;
t3140 = -t3019;
t3142 = t14.*t43.*(-1.4653732538e-2);
t3162 = t15.*t44.*(-1.7527158935e-2);
t3170 = t16.*t45.*(-7.735484874e-3);
t3172 = -t3105;
t3184 = t15.*t44.*(-1.00241616695e-1);
t3185 = -t3122;
t3190 = t16.*t33.*3.40361334456e-4;
t3219 = t587+t689;
t3220 = -t3167;
t3230 = t607+t703;
t3235 = t16.*t40.*1.37607339936e-4;
t3240 = t630+t670;
t3243 = t649+t654;
t3246 = t41.*t44.*3.40361334456e-4;
t3248 = t643+t690;
t3249 = t651+t796;
t3260 = t681+t735;
t3263 = t652+t782;
t3271 = t34.*1.644586079438601e-3;
t3272 = t35.*8.222930397193003e-4;
t3276 = t44.*t45.*1.37607339936e-4;
t3280 = t751+t798;
t3286 = t696+t891;
t3292 = t192+t213+t277+t866;
t3296 = t628+t957;
t3297 = t30.*3.9053550262761e-3;
t3299 = t726+t818;
t3302 = t705+t847;
t3303 = t42.*1.95267751313805e-3;
t3307 = t772+t1161;
t3309 = t13.*t42.*8.222930397193003e-4;
t3350 = t644+t1443;
t3354 = t13.*t35.*1.95267751313805e-3;
t3356 = t663+t1442;
t3424 = t626+t770+3.3e+1./4.0e+2;
t3451 = t4.*(t633-t662).*(-1.0./4.0);
t3489 = t693+t784+1.1e+1./1.25e+2;
t3518 = (t4.*(t633-t662))./4.0;
t3550 = t17.*(t689-t740).*(-1.0./2.0);
t3681 = t9.*t16.*(t689-t740).*(-1.0./4.0);
t3699 = t6.*t15.*(t733-t806).*(-1.0./4.0);
t3702 = (t9.*t16.*(t689-t740))./4.0;
t3722 = (t6.*t15.*(t733-t806))./4.0;
t3745 = t14.*t43.*(t733-t806).*(-1.0./4.0);
t4062 = -t4047;
t4069 = t37.*8.583920692030934e-3;
t4073 = t45.*8.36241330891889e-4;
t4079 = t41.*2.74179553204116e-4;
t4082 = t14.*t43.*1.082026026049065e-3;
t4085 = t44.*5.187945860934245e-5;
t4086 = t43.*5.133938885144471e-4;
t4087 = -t4066;
t4090 = t14.*t37.*2.300122758781553e-3;
t4091 = t39.*4.67845486573025e-5;
t4094 = -t4071;
t4103 = -t4080;
t4105 = -t4084;
t4120 = -t4092;
t4124 = t16.*t41.*8.36241330891889e-4;
t4126 = -t4095;
t4135 = t16.*t45.*2.74179553204116e-4;
t4138 = t15.*t39.*5.187945860934245e-5;
t4145 = -t4110;
t4148 = -t4115;
t4151 = t15.*t44.*4.67845486573025e-5;
t4154 = t34.*5.434755381414281e-3;
t4155 = t35.*5.434755381414281e-3;
t4156 = t5.*t4096;
t4163 = -t4130;
t4174 = t36.*5.897280115119475e-3;
t4175 = t37.*5.897280115119475e-3;
t4176 = t6.*t4110;
t4186 = t38.*2.454825983680473e-3;
t4187 = t39.*2.454825983680473e-3;
t4188 = t7.*t4130;
t4209 = -t4178;
t4222 = t13.*t42.*5.434755381414281e-3;
t4239 = t14.*t43.*5.897280115119475e-3;
t4249 = t15.*t44.*2.454825983680473e-3;
t4264 = -t4241;
t4294 = t12.*t19.*1.004890920085612e-1;
t4296 = t12.*t25.*1.004890920085612e-1;
t4298 = t1176+t2841;
t4300 = t971+t2845;
t4337 = t1679+t2846;
t4681 = t1744+t1827-2.960013375e-1;
t4860 = t2716+t2721;
t4884 = t2766+t2782;
t4916 = t2712+t3113;
t4922 = t2722+t3112;
t4959 = t2954+t2972;
t5011 = -t4.*(t2959-t2967);
t5012 = -t5.*(t2959-t2967);
t5015 = -t12.*(t2959-t2967);
t5016 = -t13.*(t2959-t2967);
t5044 = -t30.*(t2959-t2967);
t5047 = -t34.*(t2959-t2967);
t5048 = -t35.*(t2959-t2967);
t5052 = -t42.*(t2959-t2967);
t5076 = t4.*t5.*(t2959-t2967);
t5077 = t30.*(t2959-t2967);
t5078 = t34.*(t2959-t2967);
t5079 = t35.*(t2959-t2967);
t5080 = t12.*t13.*(t2959-t2967);
t5081 = t42.*(t2959-t2967);
t5083 = t1005+t1115+t2893;
t5137 = t1526+t1628+t2806;
t5331 = t2729+t2744+1.01140545e-1;
t5365 = t2772+t2775+6.4725936e-2;
t5437 = t12.*(t2959-t2967).*(-3.228604);
t5439 = t13.*(t2959-t2967).*(-3.228604);
t5440 = t5.*(t2959-t2967).*(-3.587895);
t5441 = t1116+t2765+t2892;
t5451 = t4.*(t2959-t2967).*(-3.228604);
t5452 = t5.*(t2959-t2967).*(-3.228604);
t5455 = t12.*(t2959-t2967).*(-6.46926e-1);
t5463 = t4.*(t2959-t2967).*(-6.46926e-1);
t5465 = t4.*t13.*(t2959-t2967).*(-3.587895);
t5759 = t4019+t4044;
t5889 = t13.*(t2959-t2967).*(-6.3364582104e-2);
t5900 = t5.*(t2959-t2967).*(-4.4422362436e-2);
t5902 = t13.*(t2959-t2967).*6.3364582104e-2;
t5916 = t5.*(t2959-t2967).*4.4422362436e-2;
t5943 = t5.*t12.*(t2959-t2967).*(-6.3364582104e-2);
t5963 = t5.*t12.*(t2959-t2967).*6.3364582104e-2;
t81 = -t48;
t101 = -t51;
t102 = -t52;
t104 = t12.*t75;
t106 = t13.*t79;
t108 = -t54;
t109 = -t55;
t110 = -t60;
t111 = -t66;
t112 = -t67;
t115 = -t69;
t116 = -t71;
t117 = -t72;
t118 = -t76;
t119 = -t77;
t120 = -t79;
t171 = -t100;
t172 = -t103;
t173 = -t105;
t175 = -t113;
t190 = -t158;
t193 = -t166;
t205 = -t178;
t206 = t47.*(1.1e+1./1.25e+2);
t208 = t48.*(1.1e+1./1.25e+2);
t210 = t47.*(4.8e+1./1.25e+2);
t214 = -t196;
t223 = t30+t68;
t224 = t42+t50;
t225 = t36+t59;
t226 = t37+t58;
t227 = t38+t63;
t228 = t39+t62;
t229 = t33+t80;
t230 = t45+t53;
t231 = t50.*(4.8e+1./1.25e+2);
t232 = t56.*(1.1e+1./1.25e+2);
t233 = t57.*(1.1e+1./1.25e+2);
t234 = t58.*(1.1e+1./1.25e+2);
t235 = t59.*(1.1e+1./1.25e+2);
t236 = t60.*(1.1e+1./1.25e+2);
t237 = t61.*(1.1e+1./1.25e+2);
t238 = t62.*(1.1e+1./1.25e+2);
t239 = t63.*(1.1e+1./1.25e+2);
t241 = t67.*(1.1e+1./1.25e+2);
t242 = t55.*(4.8e+1./1.25e+2);
t243 = t56.*(4.8e+1./1.25e+2);
t244 = t57.*(4.8e+1./1.25e+2);
t245 = t67.*(4.8e+1./1.25e+2);
t246 = t54.*(3.3e+1./4.0e+2);
t248 = t55.*(3.3e+1./4.0e+2);
t249 = t71.*(1.1e+1./1.25e+2);
t250 = t72.*(1.1e+1./1.25e+2);
t251 = t75.*(1.1e+1./1.25e+2);
t252 = t76.*(1.1e+1./1.25e+2);
t254 = t80.*(1.1e+1./1.25e+2);
t256 = t68.*(4.8e+1./1.25e+2);
t258 = t69.*(4.8e+1./1.25e+2);
t259 = t70.*(4.8e+1./1.25e+2);
t260 = t71.*(4.8e+1./1.25e+2);
t261 = t80.*(4.8e+1./1.25e+2);
t263 = t68.*(3.3e+1./4.0e+2);
t268 = t47.*(7.9e+1./2.5e+2);
t283 = t55.*(7.9e+1./2.5e+2);
t290 = -t257;
t294 = t68.*(7.9e+1./2.5e+2);
t296 = t71.*(7.9e+1./2.5e+2);
t327 = t103.*(1.1e+1./1.25e+2);
t329 = t105.*(1.1e+1./1.25e+2);
t336 = -t305;
t338 = -t311;
t361 = -t331;
t362 = -t335;
t365 = -t341;
t369 = t70+t98;
t370 = t74+t99;
t371 = t65+t107;
t372 = t50.*1.0442e-1;
t373 = t54.*1.9552e-2;
t374 = t55.*1.9552e-2;
t375 = t55.*1.0442e-1;
t376 = t68.*1.9552e-2;
t377 = t68.*1.0442e-1;
t399 = t54.*5.317e-2;
t400 = t55.*5.317e-2;
t401 = t68.*5.317e-2;
t419 = t83+t128;
t420 = t97+t136;
t421 = t7.*t406;
t422 = t15.*t406;
t433 = t85+t183;
t437 = t161+t165;
t444 = t134+t191;
t445 = t139+t184;
t449 = t149+t198;
t459 = t177+t191;
t461 = t185+t198;
t463 = t9.*t432;
t467 = t17.*t432;
t478 = t7.*t438;
t481 = t15.*t438;
t487 = t7.*(t134+t14.*t122);
t489 = t15.*(t134+t14.*t122);
t492 = t7.*(t149+t14.*t127);
t496 = t15.*(t149+t14.*t127);
t502 = t264+t267;
t512 = t220+t271;
t528 = t282+t297;
t530 = t211+t334;
t536 = t217+t318;
t544 = -t7.*(t257+t269);
t546 = -t15.*(t257+t269);
t552 = -t7.*(t295-t13.*t42.*(3.3e+1./4.0e+2));
t553 = -t8.*(t295-t13.*t42.*(3.3e+1./4.0e+2));
t554 = t316+t344;
t555 = -t15.*(t295-t13.*t42.*(3.3e+1./4.0e+2));
t556 = -t16.*(t295-t13.*t42.*(3.3e+1./4.0e+2));
t559 = (t4.*t494)./2.0;
t564 = t7.*(t257+t269);
t570 = t7.*(t295-t13.*t42.*(3.3e+1./4.0e+2));
t572 = t15.*(t295-t13.*t42.*(3.3e+1./4.0e+2));
t575 = t127+t161+t195;
t619 = -t592;
t655 = t56.*2.9474e-2;
t656 = t57.*2.9474e-2;
t657 = t58.*2.9474e-2;
t658 = t59.*2.9474e-2;
t667 = t71.*2.9474e-2;
t668 = t72.*2.9474e-2;
t675 = t47.*2.9474e-2;
t794 = -t673;
t823 = -t709;
t849 = -t731;
t859 = t188+t247+t293;
t870 = -t755;
t908 = t53.*1.2516e-2;
t915 = t67.*1.2516e-2;
t916 = t103.*2.9474e-2;
t930 = t77.*1.2516e-2;
t931 = t78.*1.2516e-2;
t932 = t79.*1.2516e-2;
t933 = t80.*1.2516e-2;
t946 = t49.*1.2516e-2;
t973 = t80.*2.82440448e-1;
t984 = t68.*3.87398936e-1;
t986 = t71.*3.87398936e-1;
t996 = t51.*3.5549e-2;
t998 = t47.*3.87398936e-1;
t1010 = -t829;
t1012 = t60.*4.815e-3;
t1013 = t61.*4.815e-3;
t1014 = t62.*4.815e-3;
t1015 = t63.*4.815e-3;
t1017 = t59.*3.5549e-2;
t1025 = -t838;
t1031 = t75.*4.815e-3;
t1032 = t76.*4.815e-3;
t1033 = t69.*3.5549e-2;
t1034 = t70.*3.5549e-2;
t1035 = t71.*3.5549e-2;
t1036 = t72.*3.5549e-2;
t1039 = t55.*1.01140545e-1;
t1042 = t51.*3.8437e-2;
t1043 = -t856;
t1044 = t48.*4.815e-3;
t1046 = t47.*3.5549e-2;
t1049 = t58.*3.8437e-2;
t1050 = t59.*3.8437e-2;
t1054 = t72.*3.8437e-2;
t1056 = -t873;
t1109 = -t922;
t1112 = -t927;
t1124 = -t938;
t1125 = -t939;
t1137 = -t949;
t1177 = t67.*2.82440448e-1;
t1178 = -t954;
t1183 = -t958;
t1185 = -t962;
t1187 = t53.*6.1597e-2;
t1188 = t48.*4.354e-3;
t1192 = -t974;
t1193 = -t979;
t1195 = t54.*8.626999999999999e-3;
t1196 = t55.*8.626999999999999e-3;
t1197 = t64.*6.1597e-2;
t1198 = t65.*6.1597e-2;
t1199 = t66.*6.1597e-2;
t1200 = t67.*6.1597e-2;
t1209 = -t983;
t1211 = -t985;
t1212 = t56.*5.433e-3;
t1213 = t57.*5.433e-3;
t1214 = t58.*5.433e-3;
t1215 = t59.*5.433e-3;
t1216 = t68.*8.626999999999999e-3;
t1218 = t77.*6.1597e-2;
t1219 = t78.*6.1597e-2;
t1220 = t79.*6.1597e-2;
t1221 = t80.*6.1597e-2;
t1222 = t16.*t842;
t1225 = -t997;
t1228 = -t1001;
t1232 = -t1008;
t1233 = t71.*5.433e-3;
t1234 = t72.*5.433e-3;
t1238 = t49.*6.1597e-2;
t1239 = t16.*t856;
t1240 = t50.*2.5853e-2;
t1241 = t50.*2.7454e-2;
t1242 = -t1020;
t1244 = t47.*5.433e-3;
t1247 = t55.*2.5853e-2;
t1250 = t54.*2.7454e-2;
t1251 = t55.*2.7454e-2;
t1255 = t68.*2.5853e-2;
t1258 = t68.*2.7454e-2;
t1259 = t13.*t873;
t1265 = t13.*t882;
t1266 = -t1055;
t1267 = t56.*6.0149e-2;
t1268 = t57.*6.0149e-2;
t1269 = t58.*6.0149e-2;
t1270 = t59.*6.0149e-2;
t1271 = t60.*6.0149e-2;
t1272 = t61.*6.0149e-2;
t1273 = t62.*6.0149e-2;
t1274 = t63.*6.0149e-2;
t1283 = -t1058;
t1285 = -t1060;
t1286 = t71.*6.0149e-2;
t1287 = t72.*6.0149e-2;
t1288 = t75.*6.0149e-2;
t1289 = t76.*6.0149e-2;
t1292 = t47.*6.0149e-2;
t1294 = t48.*6.0149e-2;
t1296 = -t1071;
t1298 = t51.*4.1065e-2;
t1299 = t54.*8.640999999999999e-3;
t1300 = t55.*8.640999999999999e-3;
t1301 = t100.*1.2516e-2;
t1305 = t54.*4.1065e-2;
t1306 = t55.*4.1065e-2;
t1307 = t59.*4.1065e-2;
t1308 = t68.*8.640999999999999e-3;
t1310 = -t1094;
t1311 = -t1095;
t1313 = t69.*6.3995712e-1;
t1314 = t70.*6.3995712e-1;
t1315 = t71.*6.3995712e-1;
t1317 = t68.*4.1065e-2;
t1318 = t69.*4.1065e-2;
t1319 = t70.*4.1065e-2;
t1320 = t71.*4.1065e-2;
t1321 = t72.*4.1065e-2;
t1324 = t114.*1.2516e-2;
t1327 = t47.*6.3995712e-1;
t1329 = t47.*4.1065e-2;
t1331 = -t1127;
t1332 = -t1128;
t1333 = -t1134;
t1336 = -t1138;
t1339 = -t1149;
t1341 = t60.*4.354e-3;
t1342 = t61.*4.354e-3;
t1343 = t62.*4.354e-3;
t1344 = t63.*4.354e-3;
t1346 = -t1157;
t1359 = t75.*4.354e-3;
t1360 = t76.*4.354e-3;
t1362 = t71.*1.158e-3;
t1363 = t72.*1.158e-3;
t1364 = t73.*1.158e-3;
t1365 = t74.*1.158e-3;
t1366 = t75.*1.158e-3;
t1367 = t76.*1.158e-3;
t1369 = t55.*1.332e-3;
t1372 = -t1191;
t1373 = t47.*1.158e-3;
t1375 = t48.*1.158e-3;
t1376 = t64.*1.0027e-2;
t1377 = t65.*1.0027e-2;
t1378 = t66.*1.0027e-2;
t1379 = t67.*1.0027e-2;
t1381 = t68.*1.332e-3;
t1385 = -t1202;
t1387 = t98.*3.5549e-2;
t1388 = t79.*1.0027e-2;
t1389 = t80.*1.0027e-2;
t1395 = t105.*4.815e-3;
t1396 = t49.*1.0027e-2;
t1401 = -t1245;
t1402 = t98.*3.8437e-2;
t1408 = t52.*1.964e-3;
t1409 = t103.*3.8437e-2;
t1412 = t63.*1.964e-3;
t1413 = -t1263;
t1414 = t53.*4.252e-3;
t1416 = t54.*1.1953e-2;
t1417 = t55.*1.1953e-2;
t1418 = t56.*1.1953e-2;
t1419 = t57.*1.1953e-2;
t1420 = t58.*1.1953e-2;
t1421 = t59.*1.1953e-2;
t1424 = t73.*1.964e-3;
t1425 = t74.*1.964e-3;
t1426 = t75.*1.964e-3;
t1427 = t76.*1.964e-3;
t1430 = -t1279;
t1431 = t60.*4.252e-3;
t1432 = t61.*4.252e-3;
t1433 = t62.*4.252e-3;
t1434 = t63.*4.252e-3;
t1435 = t67.*4.252e-3;
t1436 = t68.*1.1953e-2;
t1437 = t71.*1.1953e-2;
t1438 = t72.*1.1953e-2;
t1444 = t48.*1.964e-3;
t1445 = t52.*1.4117e-2;
t1447 = t75.*4.252e-3;
t1448 = t76.*4.252e-3;
t1449 = t77.*4.252e-3;
t1450 = t78.*4.252e-3;
t1451 = t79.*4.252e-3;
t1452 = t80.*4.252e-3;
t1455 = t47.*1.1953e-2;
t1463 = t56.*1.4117e-2;
t1464 = t57.*1.4117e-2;
t1465 = t58.*1.4117e-2;
t1466 = t59.*1.4117e-2;
t1467 = t63.*1.4117e-2;
t1468 = t48.*4.252e-3;
t1470 = t49.*4.252e-3;
t1472 = t53.*4.28e-4;
t1476 = t71.*1.4117e-2;
t1477 = t72.*1.4117e-2;
t1478 = t73.*1.4117e-2;
t1479 = t74.*1.4117e-2;
t1480 = t75.*1.4117e-2;
t1481 = t76.*1.4117e-2;
t1483 = t53.*1.196e-3;
t1485 = t64.*4.28e-4;
t1486 = t65.*4.28e-4;
t1487 = t66.*4.28e-4;
t1488 = t67.*4.28e-4;
t1489 = t50.*7.796e-3;
t1490 = t121+t302+t366;
t1491 = t52.*1.0517e-2;
t1492 = t47.*1.4117e-2;
t1494 = t48.*1.4117e-2;
t1495 = t51.*2.117e-3;
t1497 = t60.*1.196e-3;
t1498 = t61.*1.196e-3;
t1499 = t62.*1.196e-3;
t1500 = t63.*1.196e-3;
t1501 = t67.*1.196e-3;
t1503 = t77.*4.28e-4;
t1504 = t78.*4.28e-4;
t1505 = t79.*4.28e-4;
t1506 = t80.*4.28e-4;
t1507 = t16.*t1128;
t1508 = t54.*7.796e-3;
t1509 = t55.*7.796e-3;
t1511 = t60.*1.0517e-2;
t1512 = t61.*1.0517e-2;
t1513 = t62.*1.0517e-2;
t1514 = t63.*1.0517e-2;
t1515 = t64.*1.0517e-2;
t1516 = t65.*1.0517e-2;
t1517 = t66.*1.0517e-2;
t1518 = t67.*1.0517e-2;
t1522 = t56.*2.117e-3;
t1523 = t57.*2.117e-3;
t1524 = t58.*2.117e-3;
t1525 = t59.*2.117e-3;
t1528 = t75.*1.196e-3;
t1529 = t76.*1.196e-3;
t1530 = t77.*1.196e-3;
t1531 = t78.*1.196e-3;
t1532 = t79.*1.196e-3;
t1533 = t80.*1.196e-3;
t1535 = t51.*4.037e-3;
t1536 = t49.*4.28e-4;
t1537 = t16.*t1147;
t1538 = t68.*7.796e-3;
t1539 = t13.*t1150;
t1541 = t73.*1.0517e-2;
t1542 = t74.*1.0517e-2;
t1543 = t75.*1.0517e-2;
t1544 = t76.*1.0517e-2;
t1545 = t15.*t1154;
t1546 = t79.*1.0517e-2;
t1547 = t80.*1.0517e-2;
t1552 = t69.*2.117e-3;
t1553 = t70.*2.117e-3;
t1554 = t71.*2.117e-3;
t1555 = t72.*2.117e-3;
t1556 = t14.*t1163;
t1558 = t48.*1.196e-3;
t1560 = t49.*1.196e-3;
t1561 = t54.*4.037e-3;
t1562 = t55.*4.037e-3;
t1563 = t59.*4.037e-3;
t1564 = t13.*t1173;
t1565 = t56.*6.4725936e-2;
t1566 = t57.*6.4725936e-2;
t1567 = t58.*6.4725936e-2;
t1568 = t59.*6.4725936e-2;
t1570 = t67.*6.4725936e-2;
t1571 = -t1335;
t1572 = t125+t312+t368;
t1573 = t52.*1.158e-3;
t1574 = t48.*1.0517e-2;
t1575 = t15.*t954;
t1576 = t49.*1.0517e-2;
t1580 = t47.*2.117e-3;
t1581 = t14.*t958;
t1583 = t68.*4.037e-3;
t1584 = t69.*4.037e-3;
t1585 = t70.*4.037e-3;
t1586 = t71.*4.037e-3;
t1587 = t72.*4.037e-3;
t1589 = t71.*6.4725936e-2;
t1590 = t72.*6.4725936e-2;
t1592 = t80.*6.4725936e-2;
t1595 = t56.*1.158e-3;
t1596 = t57.*1.158e-3;
t1597 = t58.*1.158e-3;
t1598 = t59.*1.158e-3;
t1599 = t63.*1.158e-3;
t1600 = t50.*1.332e-3;
t1603 = t47.*4.037e-3;
t1604 = t47.*6.4725936e-2;
t1607 = t68.*2.29e-4;
t1608 = t71.*2.29e-4;
t1609 = t72.*2.29e-4;
t1612 = t107.*6.1597e-2;
t1614 = t47.*2.29e-4;
t1616 = -t1374;
t1620 = t103.*5.433e-3;
t1621 = t114.*6.1597e-2;
t1631 = t60.*7.41e-4;
t1632 = t61.*7.41e-4;
t1633 = t62.*7.41e-4;
t1634 = t63.*7.41e-4;
t1635 = t64.*7.41e-4;
t1636 = t65.*7.41e-4;
t1637 = t66.*7.41e-4;
t1638 = t67.*7.41e-4;
t1641 = t75.*7.41e-4;
t1642 = t76.*7.41e-4;
t1643 = t79.*7.41e-4;
t1644 = t80.*7.41e-4;
t1645 = t103.*6.0149e-2;
t1647 = t105.*6.0149e-2;
t1649 = t48.*7.41e-4;
t1651 = t49.*7.41e-4;
t1661 = -t1454;
t1663 = t98.*4.1065e-2;
t1668 = -t1469;
t1683 = t56.*3.41e-4;
t1684 = t57.*3.41e-4;
t1685 = t58.*3.41e-4;
t1686 = t59.*3.41e-4;
t1687 = t60.*3.41e-4;
t1688 = t61.*3.41e-4;
t1689 = t62.*3.41e-4;
t1690 = t63.*3.41e-4;
t1691 = -t1519;
t1703 = t71.*3.41e-4;
t1704 = t72.*3.41e-4;
t1705 = t75.*3.41e-4;
t1706 = t76.*3.41e-4;
t1712 = -t1559;
t1716 = t105.*4.354e-3;
t1720 = t47.*3.41e-4;
t1722 = t48.*3.41e-4;
t1730 = t54.*2.29e-4;
t1731 = t55.*2.29e-4;
t1732 = t56.*2.29e-4;
t1733 = t57.*2.29e-4;
t1734 = t58.*2.29e-4;
t1735 = t59.*2.29e-4;
t1739 = t100.*6.1597e-2;
t1741 = t107.*1.0027e-2;
t1746 = t55.*1.13377482;
t1750 = t68.*1.13377482;
t1753 = t99.*1.964e-3;
t1758 = t100.*4.252e-3;
t1759 = t103.*1.1953e-2;
t1761 = t113.*1.964e-3;
t1764 = t105.*4.252e-3;
t1765 = t99.*1.4117e-2;
t1766 = t114.*4.252e-3;
t1767 = t103.*1.4117e-2;
t1768 = t100.*4.28e-4;
t1769 = t52.*1.09e-4;
t1770 = t113.*1.4117e-2;
t1772 = t55.*2.960013375e-1;
t1773 = t100.*1.196e-3;
t1775 = t107.*4.28e-4;
t1776 = -t1669;
t1779 = t99.*1.0517e-2;
t1780 = t60.*1.09e-4;
t1781 = t61.*1.09e-4;
t1782 = t62.*1.09e-4;
t1783 = t63.*1.09e-4;
t1784 = t98.*2.117e-3;
t1786 = t68.*2.960013375e-1;
t1789 = t105.*1.196e-3;
t1790 = t114.*4.28e-4;
t1792 = t105.*1.0517e-2;
t1794 = t107.*1.0517e-2;
t1795 = t73.*1.09e-4;
t1796 = t74.*1.09e-4;
t1797 = t75.*1.09e-4;
t1798 = t76.*1.09e-4;
t1799 = t15.*t1549;
t1800 = t103.*2.117e-3;
t1802 = t114.*1.196e-3;
t1803 = t98.*4.037e-3;
t1807 = t113.*1.0517e-2;
t1808 = t48.*1.09e-4;
t1809 = t15.*t1578;
t1811 = t103.*6.4725936e-2;
t1815 = t99.*1.158e-3;
t1819 = t103.*1.158e-3;
t1825 = t113.*1.158e-3;
t1830 = t56.*3.45563e-1;
t1831 = t57.*3.45563e-1;
t1833 = t69.*3.45563e-1;
t1834 = t70.*3.45563e-1;
t1835 = t71.*3.45563e-1;
t1838 = t47.*3.45563e-1;
t1842 = t105.*7.41e-4;
t1844 = t107.*7.41e-4;
t1847 = t71.*5.2663138e-1;
t1850 = -t1771;
t1853 = -t1785;
t1858 = t103.*3.41e-4;
t1860 = t105.*3.41e-4;
t1864 = -t1801;
t1868 = -t1817;
t1869 = t103.*2.29e-4;
t1884 = t99.*1.09e-4;
t1886 = t105.*1.09e-4;
t1887 = t113.*1.09e-4;
t1900 = -t1873;
t1909 = -t1893;
t1910 = -t1898;
t1920 = t194+t378+t402;
t1921 = t50.*3.746479959e-1;
t1922 = t55.*3.746479959e-1;
t1923 = t68.*3.746479959e-1;
t1925 = t54.*1.9076837715e-1;
t1926 = t55.*1.9076837715e-1;
t1927 = t68.*1.9076837715e-1;
t2040 = t200+t691;
t2087 = t218+t773;
t2176 = t55.*7.8691955574375e-3;
t2219 = t274+t690;
t2229 = t68.*1.5454229830875e-2;
t2255 = t68.*4.5595633420575e-2;
t2261 = -t2175;
t2304 = -t2228;
t2321 = t55.*5.13251877947625e-2;
t2333 = -t2254;
t2383 = t308+t1174;
t2393 = (t12.*t1970)./2.0;
t2422 = t3.*t2297;
t2425 = t11.*t2297;
t2443 = (t14.*t2111)./2.0;
t2468 = t3.*t2396;
t2471 = t11.*t2396;
t2486 = (t6.*t13.*t2111)./4.0;
t2520 = t432+t1156;
t2523 = (t13.*t42.*t2111)./2.0;
t2546 = t15.*(t257+t269).*(-1.225946);
t2568 = t160+t204+t883;
t2583 = t8.*(t295-t13.*t42.*(3.3e+1./4.0e+2)).*(-1.666555);
t2588 = t16.*(t295-t13.*t42.*(3.3e+1./4.0e+2)).*(-1.666555);
t2631 = t8.*(t295-t13.*t42.*(3.3e+1./4.0e+2)).*(-7.35522e-1);
t2814 = t51.*4.7121686402e-2;
t2822 = t58.*4.7121686402e-2;
t2823 = t59.*4.7121686402e-2;
t2828 = t72.*4.7121686402e-2;
t2869 = -t2800;
t2898 = -t2811;
t2909 = -t2816;
t2910 = -t2817;
t2929 = -t2829;
t2933 = -t2832;
t2945 = -t2835;
t2952 = -t2844;
t2956 = t50.*9.850206933e-2;
t2957 = -t2855;
t2960 = t54.*9.850206933e-2;
t2961 = t55.*9.850206933e-2;
t2969 = t68.*9.850206933e-2;
t2970 = t13.*t2800;
t2973 = t13.*t2805;
t2975 = t51.*5.034347249e-2;
t2976 = -t2870;
t2977 = -t2872;
t2978 = -t2873;
t2981 = t54.*5.034347249e-2;
t2982 = t55.*5.034347249e-2;
t2983 = t59.*5.034347249e-2;
t2984 = -t2876;
t2988 = t68.*5.034347249e-2;
t2989 = t69.*5.034347249e-2;
t2990 = t70.*5.034347249e-2;
t2991 = t71.*5.034347249e-2;
t2992 = t72.*5.034347249e-2;
t2995 = t98.*4.7121686402e-2;
t2997 = t47.*5.034347249e-2;
t2998 = -t2907;
t2999 = t103.*4.7121686402e-2;
t3000 = -t2919;
t3003 = t53.*4.5305948634e-2;
t3006 = t64.*4.5305948634e-2;
t3007 = t65.*4.5305948634e-2;
t3008 = t66.*4.5305948634e-2;
t3009 = t67.*4.5305948634e-2;
t3011 = t77.*4.5305948634e-2;
t3012 = t78.*4.5305948634e-2;
t3013 = t79.*4.5305948634e-2;
t3014 = t80.*4.5305948634e-2;
t3015 = t16.*t2839;
t3016 = t49.*4.5305948634e-2;
t3017 = t16.*t2844;
t3021 = t47.*1.4653732538e-2;
t3023 = -t2955;
t3027 = t52.*2.3526756935e-2;
t3028 = -t2968;
t3031 = t52.*1.7527158935e-2;
t3032 = t56.*2.3526756935e-2;
t3033 = t57.*2.3526756935e-2;
t3034 = t58.*2.3526756935e-2;
t3035 = t59.*2.3526756935e-2;
t3036 = t63.*2.3526756935e-2;
t3038 = t53.*3.127439544e-3;
t3039 = t80.*1.485213095808e-3;
t3040 = -t2974;
t3041 = t60.*1.7527158935e-2;
t3042 = t61.*1.7527158935e-2;
t3043 = t62.*1.7527158935e-2;
t3044 = t63.*1.7527158935e-2;
t3045 = t71.*2.3526756935e-2;
t3046 = t72.*2.3526756935e-2;
t3047 = t73.*2.3526756935e-2;
t3048 = t74.*2.3526756935e-2;
t3049 = t75.*2.3526756935e-2;
t3050 = t76.*2.3526756935e-2;
t3053 = t60.*3.127439544e-3;
t3054 = t61.*3.127439544e-3;
t3055 = t62.*3.127439544e-3;
t3056 = t63.*3.127439544e-3;
t3057 = t67.*3.127439544e-3;
t3058 = t73.*1.7527158935e-2;
t3059 = t74.*1.7527158935e-2;
t3060 = t75.*1.7527158935e-2;
t3061 = t76.*1.7527158935e-2;
t3062 = t15.*t2891;
t3063 = t47.*2.3526756935e-2;
t3065 = t48.*2.3526756935e-2;
t3067 = t75.*3.127439544e-3;
t3068 = t76.*3.127439544e-3;
t3069 = t77.*3.127439544e-3;
t3070 = t78.*3.127439544e-3;
t3071 = t79.*3.127439544e-3;
t3072 = t80.*3.127439544e-3;
t3074 = t60.*7.735484874e-3;
t3075 = t61.*7.735484874e-3;
t3076 = t62.*7.735484874e-3;
t3077 = t63.*7.735484874e-3;
t3078 = t64.*7.735484874e-3;
t3079 = t65.*7.735484874e-3;
t3080 = t66.*7.735484874e-3;
t3081 = t67.*7.735484874e-3;
t3082 = t48.*1.7527158935e-2;
t3083 = t15.*t2907;
t3085 = t48.*3.127439544e-3;
t3087 = t49.*3.127439544e-3;
t3088 = t75.*7.735484874e-3;
t3089 = t76.*7.735484874e-3;
t3090 = t79.*7.735484874e-3;
t3091 = t80.*7.735484874e-3;
t3093 = t48.*7.735484874e-3;
t3095 = t49.*7.735484874e-3;
t3097 = t56.*1.00241616695e-1;
t3098 = t57.*1.00241616695e-1;
t3099 = t58.*1.00241616695e-1;
t3100 = t59.*1.00241616695e-1;
t3101 = t60.*1.00241616695e-1;
t3102 = t61.*1.00241616695e-1;
t3103 = t62.*1.00241616695e-1;
t3104 = t63.*1.00241616695e-1;
t3107 = t71.*1.00241616695e-1;
t3108 = t72.*1.00241616695e-1;
t3109 = t75.*1.00241616695e-1;
t3110 = t76.*1.00241616695e-1;
t3114 = t56.*4.23641577598e-1;
t3115 = t57.*4.23641577598e-1;
t3116 = t47.*1.00241616695e-1;
t3118 = t48.*1.00241616695e-1;
t3123 = t69.*4.23641577598e-1;
t3124 = t70.*4.23641577598e-1;
t3125 = t71.*4.23641577598e-1;
t3129 = t47.*4.23641577598e-1;
t3130 = t54.*1.4653732538e-2;
t3131 = t55.*1.4653732538e-2;
t3132 = t56.*1.4653732538e-2;
t3133 = t57.*1.4653732538e-2;
t3134 = t58.*1.4653732538e-2;
t3135 = t59.*1.4653732538e-2;
t3136 = t68.*1.4653732538e-2;
t3137 = t71.*1.4653732538e-2;
t3138 = t72.*1.4653732538e-2;
t3139 = t47.*7.954268653419999e-3;
t3141 = -t3020;
t3143 = t67.*6.00468392448e-4;
t3144 = t71.*2.315289741004e-3;
t3147 = t577+t782;
t3149 = t98.*5.034347249e-2;
t3164 = -t3086;
t3173 = t567+t819;
t3174 = t100.*4.5305948634e-2;
t3180 = t107.*4.5305948634e-2;
t3186 = t114.*4.5305948634e-2;
t3191 = t67.*3.40361334456e-4;
t3196 = t99.*2.3526756935e-2;
t3200 = t99.*1.7527158935e-2;
t3202 = t103.*2.3526756935e-2;
t3203 = t100.*3.127439544e-3;
t3207 = t105.*1.7527158935e-2;
t3208 = t113.*2.3526756935e-2;
t3210 = t105.*3.127439544e-3;
t3211 = t113.*1.7527158935e-2;
t3212 = t114.*3.127439544e-3;
t3215 = t105.*7.735484874e-3;
t3217 = t107.*7.735484874e-3;
t3221 = t103.*1.00241616695e-1;
t3223 = t105.*1.00241616695e-1;
t3226 = t103.*1.4653732538e-2;
t3229 = -t3190;
t3236 = t80.*1.37607339936e-4;
t3239 = t601+t798;
t3247 = t641+t694;
t3252 = -t3235;
t3256 = t662+t728;
t3261 = t645+t785;
t3264 = t640+t808;
t3265 = t780+t790;
t3266 = t679+t919;
t3277 = t597+t1184;
t3279 = t672+t858;
t3283 = t647+t947;
t3285 = t621+t1093;
t3288 = -t3272;
t3289 = t775+t816;
t3295 = (t13.*t3030)./2.0;
t3300 = t740+t802;
t3301 = (t7.*t3106)./2.0;
t3304 = t687+t1083;
t3305 = t54.*8.222930397193003e-4;
t3306 = t55.*1.644586079438601e-3;
t3310 = t801+t1130;
t3311 = t815+t920;
t3316 = t880+t893;
t3317 = t727+t1161;
t3318 = t892+t907;
t3319 = t806+t850;
t3321 = t827+t833;
t3322 = -t3303;
t3329 = t768+t1182;
t3332 = -t3309;
t3335 = (t5.*t12.*t3030)./4.0;
t3351 = t50.*1.95267751313805e-3;
t3352 = t881+t1100;
t3353 = t68.*3.9053550262761e-3;
t3355 = (t17.*t3219)./2.0;
t3357 = (t14.*t15.*t3106)./4.0;
t3358 = t871+t1165;
t3359 = t879+t1152;
t3360 = t902+t1119;
t3362 = t953+t1077;
t3365 = t1099+t1160;
t3385 = (t15.*t3230)./2.0;
t3395 = t929+t1243;
t3396 = t648+t1653;
t3401 = -t3354;
t3404 = t889+t1325;
t3405 = t653+t1665;
t3407 = (t12.*t3240)./2.0;
t3408 = t923+t1297;
t3409 = t943+t1304;
t3421 = t1089+t1179;
t3427 = (t5.*t3263)./2.0;
t3431 = (t6.*t3248)./2.0;
t3441 = t812+t1579;
t3446 = (t9.*t16.*t3219)./4.0;
t3447 = t1022+t1338;
t3453 = t1169+t1282;
t3454 = (t5.*t3260)./4.0;
t3455 = t1069+t1347;
t3475 = (t7.*t14.*t3230)./4.0;
t3510 = t1229+t1355;
t3514 = t1194+t1208;
t3524 = t1080+t1551;
t3536 = (t9.*t3280)./2.0;
t3547 = (t6.*t3302)./4.0;
t3553 = (t12.*t13.*t3263)./4.0;
t3558 = (t13.*t14.*t3248)./4.0;
t3586 = (t12.*t13.*t3260)./4.0;
t3588 = (t16.*t3296)./2.0;
t3592 = (t7.*t3299)./4.0;
t3620 = (t8.*t3307)./2.0;
t3632 = (t17.*(t1130-t16.*t17.*1.2516e-2))./4.0;
t3653 = (t16.*t17.*t3280)./4.0;
t3659 = (t13.*t35.*t3248)./2.0;
t3661 = (t15.*(t1165-t14.*t15.*3.5549e-2))./4.0;
t3665 = (t7.*t16.*t3286)./4.0;
t3675 = (t8.*t15.*t3296)./4.0;
t3683 = (t14.*t15.*t3299)./4.0;
t3687 = (t13.*t14.*t3302)./4.0;
t3695 = (t15.*t16.*t3307)./4.0;
t3696 = (t9.*t16.*(t1130-t16.*t17.*1.2516e-2))./2.0;
t3697 = (t5.*(t929-t1029))./2.0;
t3707 = (t5.*(t889+t12.*t947))./4.0;
t3711 = (t15.*t44.*t3286)./4.0;
t3726 = (t7.*t14.*(t1165-t14.*t15.*3.5549e-2))./2.0;
t3732 = t167+t659+t1135;
t3738 = t774+t2054;
t3740 = (t12.*t13.*(t929-t1029))./4.0;
t3741 = (t7.*(t1355-t15.*t16.*1.158e-3))./2.0;
t3743 = t692+t2044;
t3746 = (t6.*(t1208-t14.*t15.*4.037e-3))./2.0;
t3748 = (t12.*t13.*(t889+t12.*t947))./2.0;
t3752 = t92+t910+t1326;
t3758 = t1821+t1836;
t3763 = t163+t783+t1030;
t3767 = t147+t700+t1011;
t3771 = t84+t901+t1312;
t3780 = t181+t795+t1155;
t3787 = (t14.*t15.*(t1355-t15.*t16.*1.158e-3))./4.0;
t3789 = (t13.*t14.*(t1208-t14.*t15.*4.037e-3))./4.0;
t3833 = t1876+t1897;
t3861 = t337+t680+t1132;
t3864 = t313+t671+t1340;
t3865 = t275+t814+t1082;
t3866 = t270+t911+t995;
t3929 = t15.*(t257+t269).*(-2.5171736245e-2);
t3953 = t8.*(t295-t13.*t42.*(3.3e+1./4.0e+2)).*(-5.01208083475e-2);
t4000 = t16.*(t295-t13.*t42.*(3.3e+1./4.0e+2)).*(-1.17633784675e-2);
t4016 = t363+t925+t1699;
t4021 = t124+t152+t650+t1345;
t4074 = t58.*1.082026026049065e-3;
t4088 = -t4069;
t4097 = -t4073;
t4102 = -t4079;
t4104 = -t4082;
t4106 = -t4085;
t4107 = -t4086;
t4108 = t56.*8.583920692030934e-3;
t4109 = t57.*8.583920692030934e-3;
t4111 = t47.*1.716784138406187e-2;
t4114 = t51.*2.300122758781553e-3;
t4117 = t53.*8.36241330891889e-4;
t4118 = -t4090;
t4119 = -t4091;
t4122 = t77.*8.36241330891889e-4;
t4123 = t78.*8.36241330891889e-4;
t4127 = t64.*2.74179553204116e-4;
t4128 = t65.*2.74179553204116e-4;
t4129 = t66.*2.74179553204116e-4;
t4131 = t103.*1.082026026049065e-3;
t4132 = t52.*5.187945860934245e-5;
t4136 = t73.*5.187945860934245e-5;
t4137 = t74.*5.187945860934245e-5;
t4139 = t69.*5.133938885144471e-4;
t4140 = t70.*5.133938885144471e-4;
t4141 = t71.*1.026787777028894e-3;
t4167 = -t4135;
t4179 = t98.*2.300122758781553e-3;
t4180 = t60.*4.67845486573025e-5;
t4181 = t61.*4.67845486573025e-5;
t4182 = t62.*4.67845486573025e-5;
t4183 = t100.*8.36241330891889e-4;
t4190 = t114.*8.36241330891889e-4;
t4193 = -t4154;
t4194 = -t4155;
t4198 = t107.*2.74179553204116e-4;
t4199 = t99.*5.187945860934245e-5;
t4203 = t113.*5.187945860934245e-5;
t4206 = -t4174;
t4214 = t54.*5.434755381414281e-3;
t4215 = t55.*5.434755381414281e-3;
t4220 = -t4186;
t4232 = t56.*5.897280115119475e-3;
t4233 = t57.*5.897280115119475e-3;
t4234 = t58.*5.897280115119475e-3;
t4235 = t59.*5.897280115119475e-3;
t4238 = t47.*5.897280115119475e-3;
t4243 = t105.*4.67845486573025e-5;
t4248 = t48.*2.454825983680473e-3;
t4262 = -t4239;
t4270 = t60.*2.454825983680473e-3;
t4271 = t61.*2.454825983680473e-3;
t4272 = t62.*2.454825983680473e-3;
t4273 = t63.*2.454825983680473e-3;
t4283 = t103.*5.897280115119475e-3;
t4306 = t105.*2.454825983680473e-3;
t4344 = t591+t661+t1101;
t4356 = t1810+t2842;
t4365 = t590+t791+t1092;
t4383 = t596+t846+t1139;
t4410 = t674+t686+t1148;
t4415 = t588+t1016+t1165;
t4432 = t666+t807+t1129;
t4447 = t634+t945+t1009;
t4450 = t632+t888+t1081;
t4451 = t714+t738+t1164;
t4466 = t739+t928+t994;
t4470 = t716+t903+t1093;
t4471 = t749+t820+t959;
t4473 = t742+t1051+t1151;
t4475 = t734+t869+t1358;
t4476 = t608+t1281+t1330;
t4477 = t606+t1146+t1446;
t4486 = t9.*t2044.*1.13264871585e-2;
t4491 = t17.*t2054.*1.13264871585e-2;
t4494 = t638+t1172+t1207;
t4495 = t637+t992+t1181;
t4499 = t905+t1021+t1111;
t4510 = t761+t976+t1354;
t4512 = t741+t966+t1224;
t4515 = t1040+t1066+t1130;
t4526 = t732+t1284+t1550;
t4527 = t725+t1065+t1724;
t4532 = t817+t977+t1520;
t4534 = t805+t821+t1707;
t4558 = t826+t1323+t1382;
t4619 = t854+t1368+t1723;
t4624 = t1007+t1256+t1714;
t4635 = t747+t1534+t1762;
t4662 = t1026+t1588+t1615;
t4711 = t1189+t1351+t1863;
t4724 = t583.*(t1748-t1821).*(-1.0./2.0);
t4726 = t990+t1428+t1866;
t4746 = (t583.*(t1748-t1821))./2.0;
t4841 = t1052+t1890+t1901;
t4843 = t1057+t1894+t1903;
t4873 = t2713+t2755;
t4879 = t2726+t2797;
t4896 = t2769+t2834;
t4900 = t2762+t2843;
t4905 = t1410+t1924+t1949;
t4906 = t2792+t2847;
t4908 = t2787+t2793;
t4917 = t2827+t2861;
t4924 = t2848+t2868;
t4930 = t2715+t3172;
t4931 = t2821+t2965;
t4936 = t2720+t3185;
t4938 = t2914+t2922;
t4939 = t2897+t2941;
t4943 = t2812+t2958;
t4945 = t2889+t3001;
t4948 = t2904+t3004;
t4970 = t2967+t3024;
t4992 = t5.*t4959;
t4994 = t13.*t4959;
t5001 = t9.*t4298.*1.539925e-2;
t5009 = t17.*t4300.*1.539925e-2;
t5027 = t35.*t4959;
t5029 = t42.*t4959;
t5043 = t5.*t5011;
t5045 = t13.*t5011;
t5046 = t12.*t5012;
t5051 = t13.*t5015;
t5062 = t4959+3.875e-3;
t5069 = t918+t1024+t2908;
t5070 = t5.*t3350.*2.01382560198e-1;
t5087 = t12.*t13.*t3350.*4.02765120396e-1;
t5115 = t1406+t1496+t2802;
t5430 = t950+t2784+t2877;
t5433 = t2774+t4298;
t5434 = t2768+t4300;
t5442 = t677+t2940+t2979;
t5443 = t685+t2944+t2985;
t5448 = t972+t2777+t2946;
t5449 = t982+t2771+t2949;
t5458 = t5.*t4916.*6.23745e-2;
t5466 = t5078.*(-3.587895);
t5468 = t5079.*(-3.587895);
t5470 = t5080.*(-3.587895);
t5471 = t5081.*(-3.587895);
t5475 = t5077.*(-1.225946);
t5477 = t5079.*(-1.225946);
t5479 = t5081.*(-1.225946);
t5482 = t5076.*(-3.228604);
t5484 = t4.*t5439;
t5485 = t5.*t5437;
t5486 = t5080.*(-3.228604);
t5487 = t5076.*(-3.587895);
t5488 = t5077.*(-3.587895);
t5489 = t5078.*3.587895;
t5490 = t5080.*3.587895;
t5491 = t5081.*3.587895;
t5495 = t5077.*1.225946;
t5496 = t5079.*1.225946;
t5500 = t12.*t13.*t4916.*1.24749e-1;
t5501 = t5076.*3.228604;
t5502 = t5076.*3.587895;
t5503 = t5077.*3.587895;
t5530 = t707+t5011;
t5531 = t4.*t4959.*9.28985736e-3;
t5535 = t719+t5015;
t5601 = t8.*t5083.*2.62925e-3;
t5610 = t5078.*(-1.8732399795e-1);
t5615 = t5077.*(-9.5384188575e-2);
t5629 = t5078.*1.8732399795e-1;
t5632 = t5077.*9.5384188575e-2;
t5665 = t14.*t5137.*6.8635e-3;
t5681 = t201+t914+t4959;
t5739 = t1407+t1710+t1826+t2801;
t5750 = t1400+t1693+t1820+t2875;
t5755 = t1640+t1694+t1747+t2795;
t5772 = t4017+t4062;
t5795 = t4049+t4087;
t5911 = t12.*t4959.*1.015997283e-3;
t5935 = t5080.*(-4.4422362436e-2);
t5953 = t5080.*4.4422362436e-2;
t6069 = t936+t1230+t2781+t2994;
t6092 = t708+t876+t2993+t3142;
t6104 = t698+t813+t3073+t3170;
t6117 = (t701-t775).*(t2904-t2927).*(-1.0./4.0);
t6149 = ((t923-t1076).*(t2821-t2864))./2.0;
t6150 = ((t943-t1091).*(t2812-t2860))./2.0;
t6338 = t5759+1.92614005e-2;
t6481 = t2849+t5463;
t6483 = t2788+t5455;
t6524 = t5365.*(t701-t775).*(-1.0./2.0);
t6533 = (t5365.*(t701-t775))./2.0;
t7362 = t1700+t2950+t4052+t4063;
t8526 = t3350.*(-t2715+t3105+t5080.*3.228604).*(-1.0./4.0);
t174 = -t106;
t265 = -t208;
t266 = -t210;
t279 = -t236;
t280 = -t242;
t281 = -t245;
t284 = -t246;
t286 = -t248;
t287 = -t249;
t288 = -t250;
t289 = -t252;
t291 = -t258;
t292 = -t260;
t298 = -t263;
t304 = -t268;
t319 = t34+t109;
t320 = t35+t108;
t321 = t31+t117;
t322 = t43+t101;
t323 = t32+t118;
t324 = t44+t102;
t325 = t40+t112;
t326 = t41+t111;
t328 = t104.*(1.1e+1./1.25e+2);
t333 = -t294;
t347 = t7.*t224;
t348 = t8.*t223;
t349 = t8.*t225;
t350 = t9.*t225;
t351 = t9.*t226;
t352 = t9.*t227;
t353 = t15.*t224;
t354 = t16.*t223;
t355 = t16.*t225;
t356 = t17.*t225;
t357 = t17.*t226;
t358 = t17.*t227;
t359 = -t327;
t360 = -t329;
t382 = t41.*t223;
t383 = t45.*t223;
t398 = -t373;
t403 = t57+t172;
t404 = t61+t173;
t405 = t78+t171;
t407 = -t399;
t408 = -t401;
t409 = t8.*t369;
t410 = t9.*t370;
t413 = t16.*t369;
t414 = t17.*t370;
t428 = t90.*t223;
t429 = t90.*t224;
t434 = t7.*t419;
t435 = t15.*t419;
t441 = -t421;
t442 = -t422;
t452 = t9.*t420;
t453 = t17.*t420;
t457 = t144+t239;
t458 = t145+t238;
t462 = t33.*t419;
t464 = t7.*t433;
t466 = t40.*t419;
t468 = t15.*t433;
t477 = t7.*t437;
t479 = t15.*t437;
t488 = t7.*t445;
t490 = t67.*t419;
t491 = t15.*t445;
t493 = t80.*t419;
t498 = -t467;
t501 = t211+t290;
t507 = t7.*t459;
t508 = t8.*t459;
t509 = t15.*t459;
t510 = t16.*t459;
t511 = t7.*t461;
t514 = t15.*t461;
t515 = -t481;
t533 = -t487;
t535 = t112.*t419;
t537 = -t496;
t545 = t7.*t502;
t547 = t15.*t502;
t548 = t7.*(t282+t13.*t190);
t549 = -t7.*(t263-t283);
t550 = t15.*(t282+t13.*t190);
t551 = -t15.*(t263-t283);
t568 = (t12.*t512)./2.0;
t573 = t122+t445;
t602 = t8.*t575;
t603 = t16.*t575;
t779 = -t656;
t860 = t189+t248+t294;
t887 = t197+t502;
t1113 = -t930;
t1114 = -t931;
t1210 = -t984;
t1226 = -t998;
t1236 = -t1012;
t1246 = -t1032;
t1248 = -t1033;
t1249 = -t1036;
t1253 = -t1039;
t1254 = -t1044;
t1257 = -t1046;
t1261 = -t1049;
t1262 = -t1050;
t1361 = -t1177;
t1370 = -t1187;
t1371 = -t1188;
t1380 = -t1196;
t1383 = -t1199;
t1384 = -t1200;
t1390 = -t1212;
t1391 = -t1218;
t1392 = -t1220;
t1393 = -t1221;
t1394 = t104.*4.815e-3;
t1398 = -t1234;
t1403 = -t1247;
t1404 = -t1251;
t1422 = -t1272;
t1439 = -t1286;
t1440 = -t1287;
t1441 = -t1289;
t1457 = -t1292;
t1458 = -t1294;
t1461 = t8.*t859;
t1471 = -t1298;
t1473 = -t1300;
t1474 = t16.*t859;
t1484 = -t1305;
t1502 = -t1320;
t1521 = -t1327;
t1582 = -t1341;
t1601 = -t1360;
t1610 = -t1367;
t1611 = t106.*6.1597e-2;
t1617 = -t1375;
t1618 = -t1376;
t1619 = -t1379;
t1622 = -t1388;
t1623 = -t1395;
t1629 = -t1402;
t1639 = -t1408;
t1646 = t104.*6.0149e-2;
t1648 = -t1417;
t1654 = -t1432;
t1655 = -t1435;
t1656 = -t1438;
t1658 = -t1445;
t1659 = -t1448;
t1660 = -t1451;
t1666 = -t1464;
t1667 = -t1468;
t1670 = -t1476;
t1671 = -t1479;
t1672 = -t1488;
t1673 = -t1492;
t1674 = -t1501;
t1675 = -t1504;
t1676 = -t1505;
t1677 = -t1508;
t1678 = -t1509;
t1680 = -t1511;
t1681 = -t1512;
t1682 = -t1517;
t1692 = -t1523;
t1695 = -t1528;
t1696 = -t1529;
t1697 = -t1530;
t1698 = -t1532;
t1701 = -t1541;
t1702 = -t1544;
t1708 = -t1552;
t1709 = -t1555;
t1711 = -t1558;
t1713 = -t1562;
t1715 = t104.*4.354e-3;
t1717 = -t1574;
t1725 = -t1580;
t1726 = -t1584;
t1727 = -t1587;
t1728 = -t1589;
t1729 = -t1590;
t1736 = -t1595;
t1737 = -t1596;
t1738 = -t1603;
t1740 = t106.*1.0027e-2;
t1742 = -t1620;
t1754 = -t1631;
t1755 = -t1632;
t1756 = -t1635;
t1757 = -t1637;
t1760 = -t1645;
t1763 = t104.*4.252e-3;
t1774 = t106.*4.28e-4;
t1788 = t104.*1.196e-3;
t1791 = t104.*1.0517e-2;
t1793 = t106.*1.0517e-2;
t1805 = -t1687;
t1806 = -t1688;
t1813 = -t1703;
t1814 = -t1704;
t1816 = -t1716;
t1822 = -t1731;
t1823 = -t1733;
t1828 = -t1739;
t1841 = t104.*7.41e-4;
t1843 = t106.*7.41e-4;
t1845 = -t1758;
t1846 = -t1759;
t1848 = -t1765;
t1849 = -t1769;
t1851 = -t1773;
t1854 = -t1786;
t1856 = -t1789;
t1857 = -t1792;
t1859 = t104.*3.41e-4;
t1861 = -t1795;
t1862 = -t1798;
t1865 = -t1808;
t1867 = -t1811;
t1870 = -t1825;
t1877 = -t1830;
t1880 = -t1835;
t1881 = -t1838;
t1882 = t223.*t569;
t1885 = t104.*1.09e-4;
t1888 = -t1858;
t1908 = -t1886;
t1929 = t7.*t223.*3.8437e-2;
t1931 = t15.*t223.*3.8437e-2;
t1935 = t133+t190+t248+t256;
t1941 = -t1925;
t1944 = t223.*t607;
t1946 = -t1927;
t1954 = t223.*t659;
t1958 = t223.*t679;
t1979 = t223.*t639;
t1990 = t223.*t777;
t1999 = t223.*t795;
t2022 = t223.*t694;
t2034 = t223.*t703;
t2036 = t223.*t705;
t2038 = t223.*t717;
t2045 = t223.*t732;
t2057 = t15.*t223.*(-5.433e-3);
t2077 = t15.*t223.*(-1.1953e-2);
t2100 = t223.*t817;
t2116 = t223.*t847;
t2208 = t15.*t223.*(-3.41e-4);
t2262 = -t2176;
t2292 = t421.*1.666555;
t2301 = t422.*1.666555;
t2305 = -t2229;
t2307 = t421.*1.225946;
t2310 = t422.*1.225946;
t2334 = -t2255;
t2403 = t463.*7.35522e-1;
t2407 = t467.*7.35522e-1;
t2420 = (t4.*t2040)./2.0;
t2424 = -t2393;
t2434 = t478.*1.666555;
t2438 = t478.*1.225946;
t2441 = t481.*1.225946;
t2448 = t487.*1.666555;
t2450 = t492.*1.666555;
t2451 = t496.*1.666555;
t2452 = t487.*1.225946;
t2454 = t489.*1.225946;
t2456 = t492.*1.225946;
t2457 = t496.*1.225946;
t2460 = (t6.*t2219)./2.0;
t2461 = -t2425;
t2501 = t420+t955;
t2502 = -t2486;
t2503 = (t13.*t14.*t2219)./4.0;
t2521 = (t6.*t2383)./4.0;
t2533 = t564.*(-1.666555);
t2540 = t564.*(-1.225946);
t2561 = t445+t875;
t2578 = t15.*(t263-t283).*(-1.666555);
t2581 = t564.*1.666555;
t2582 = t570.*(-1.666555);
t2587 = t572.*(-1.666555);
t2591 = t7.*(t263-t283).*(-1.225946);
t2595 = t15.*(t263-t283).*(-1.225946);
t2600 = t564.*1.225946;
t2601 = t570.*(-1.225946);
t2605 = t572.*(-1.225946);
t2608 = (t13.*t14.*t2383)./2.0;
t2641 = t570.*1.666555;
t2645 = t570.*1.225946;
t2648 = t572.*1.225946;
t2701 = t301+t365+t377+t400;
t2808 = (t223.*t2219)./4.0;
t2924 = -t2822;
t2925 = -t2823;
t3025 = -t2961;
t3029 = (t223.*t2383)./4.0;
t3052 = -t2975;
t3066 = -t2981;
t3084 = -t2991;
t3092 = -t2995;
t3111 = -t3003;
t3120 = -t3008;
t3121 = -t3009;
t3126 = -t3011;
t3127 = -t3013;
t3128 = -t3014;
t3145 = -t3027;
t3148 = -t3033;
t3150 = -t3039;
t3151 = -t3042;
t3152 = -t3045;
t3153 = -t3048;
t3154 = -t3054;
t3155 = -t3057;
t3156 = -t3058;
t3157 = -t3063;
t3158 = -t3068;
t3159 = -t3071;
t3160 = -t3074;
t3161 = -t3080;
t3163 = -t3085;
t3165 = -t3089;
t3169 = -t3093;
t3171 = -t3102;
t3176 = -t3107;
t3177 = -t3108;
t3178 = -t3110;
t3179 = t106.*4.5305948634e-2;
t3181 = -t3114;
t3182 = -t3116;
t3183 = -t3118;
t3187 = -t3125;
t3188 = -t3129;
t3189 = -t3131;
t3192 = -t3138;
t3193 = -t3139;
t3194 = -t3143;
t3197 = -t3144;
t3206 = t104.*1.7527158935e-2;
t3209 = t104.*3.127439544e-3;
t3214 = t104.*7.735484874e-3;
t3216 = t106.*7.735484874e-3;
t3222 = t104.*1.00241616695e-1;
t3224 = -t3174;
t3232 = -t3196;
t3233 = -t3203;
t3238 = -t3215;
t3241 = -t3221;
t3244 = -t3226;
t3254 = t221+t461+t874;
t3275 = t216+t459+t1061;
t3290 = t7.*t223.*4.7121686402e-2;
t3293 = t15.*t223.*4.7121686402e-2;
t3314 = (t5.*t3147)./2.0;
t3315 = -t3295;
t3320 = -t3301;
t3323 = (t15.*t3173)./2.0;
t3325 = -t3305;
t3326 = -t3306;
t3327 = t223.*t2726;
t3386 = t223.*t2784;
t3390 = -t3335;
t3393 = (t12.*t13.*t3147)./4.0;
t3397 = -t3351;
t3398 = (t9.*t3239)./2.0;
t3399 = t223.*t2748;
t3402 = (t7.*t14.*t3173)./4.0;
t3403 = -t3355;
t3406 = -t3357;
t3414 = t223.*t2765;
t3430 = (t7.*t3247)./2.0;
t3449 = t15.*t223.*(-1.4653732538e-2);
t3482 = (t13.*t3283)./2.0;
t3485 = -t3431;
t3491 = (t13.*t3285)./4.0;
t3493 = (t14.*t3264)./2.0;
t3511 = (t7.*t3277)./4.0;
t3512 = (t16.*t17.*t3239)./4.0;
t3526 = -t3454;
t3554 = -t3475;
t3557 = (t14.*t15.*t3247)./4.0;
t3599 = -t3547;
t3602 = (t5.*t12.*t3283)./4.0;
t3604 = (t5.*t12.*t3285)./2.0;
t3605 = -t3553;
t3606 = (t6.*t13.*t3264)./4.0;
t3609 = -t3558;
t3617 = (t8.*t3304)./4.0;
t3629 = (t4.*t3311)./2.0;
t3633 = (t14.*t15.*t3277)./2.0;
t3641 = (t5.*t12.*t3279)./2.0;
t3642 = (t4.*t13.*t3279)./4.0;
t3643 = t248+t294+t364+t1259;
t3645 = (t8.*t3317)./2.0;
t3647 = -t3586;
t3651 = -t3588;
t3656 = -t3592;
t3662 = (t14.*t3359)./4.0;
t3671 = (t16.*t3329)./2.0;
t3689 = -t3659;
t3690 = -t3661;
t3692 = -t3665;
t3694 = (t15.*t16.*t3304)./4.0;
t3698 = (t15.*t16.*t3317)./4.0;
t3704 = -t3683;
t3705 = (t5.*t14.*t3321)./4.0;
t3708 = -t3687;
t3709 = (t8.*t3453)./2.0;
t3712 = (t8.*t15.*t3329)./4.0;
t3714 = -t3696;
t3717 = (t8.*t3441)./4.0;
t3719 = -t3697;
t3721 = (t9.*t3447)./4.0;
t3727 = (t6.*t13.*t3359)./2.0;
t3730 = (t16.*t3524)./4.0;
t3733 = t2422.*4.970684;
t3734 = t2425.*4.970684;
t3747 = (t13.*t42.*t3321)./4.0;
t3749 = -t3726;
t3750 = t2422.*6.46926e-1;
t3751 = t2425.*6.46926e-1;
t3753 = (t225.*t3173)./4.0;
t3754 = (t226.*t3173)./4.0;
t3756 = t467.*3.867742437e-3;
t3760 = (t15.*t16.*t3441)./2.0;
t3761 = -t3740;
t3765 = (t16.*t17.*t3447)./2.0;
t3770 = -t3748;
t3772 = (t15.*t16.*t3453)./4.0;
t3776 = t463.*1.563719772e-3;
t3782 = t481.*2.5171736245e-2;
t3792 = t478.*7.326866269e-3;
t3794 = (t8.*t15.*t3524)./2.0;
t3799 = (t229.*t3239)./4.0;
t3800 = (t230.*t3239)./4.0;
t3801 = t489.*2.5171736245e-2;
t3810 = -t3787;
t3811 = t487.*7.326866269e-3;
t3812 = t2468.*4.970684;
t3815 = (t225.*t3230)./4.0;
t3816 = t2471.*4.970684;
t3836 = t2468.*6.46926e-1;
t3837 = t2471.*6.46926e-1;
t3839 = -t8.*(-t244+t268+t15.*(t257+t269)+t7.*(t263-t283));
t3841 = -t16.*(-t244+t268+t15.*(t257+t269)+t7.*(t263-t283));
t3843 = (t223.*t3248)./4.0;
t3844 = (t224.*t3248)./4.0;
t3857 = t2422.*9.630700250000001e-3;
t3860 = t2425.*9.630700250000001e-3;
t3869 = (t229.*t3280)./4.0;
t3905 = (t227.*t3296)./4.0;
t3906 = (t228.*t3296)./4.0;
t3909 = (t223.*t3302)./4.0;
t3915 = t8.*(-t244+t268+t15.*(t257+t269)+t7.*(t263-t283));
t3920 = (t228.*t3286)./4.0;
t3931 = t226.*(t733-t806).*(-1.0./4.0);
t3935 = t564.*(-7.326866269e-3);
t3954 = (t226.*(t733-t806))./4.0;
t3958 = t2468.*9.630700250000001e-3;
t3960 = t15.*(t263-t283).*(-7.326866269e-3);
t3961 = (t369.*t3247)./4.0;
t3962 = (t225.*(t1165-t14.*t15.*3.5549e-2))./4.0;
t3964 = t2471.*9.630700250000001e-3;
t3971 = (t227.*t3329)./4.0;
t3975 = t7.*(t263-t283).*(-2.5171736245e-2);
t3977 = t15.*t223.*(t733-t806).*(-1.0./4.0);
t3984 = t15.*(t263-t283).*7.326866269e-3;
t4002 = t371.*(t689-t740).*(-1.0./4.0);
t4003 = (t229.*t3447)./4.0;
t4005 = (t15.*t223.*(t733-t806))./4.0;
t4022 = (t223.*(t1208-t14.*t15.*4.037e-3))./4.0;
t4026 = (t4.*t3865)./2.0;
t4027 = (t14.*t3864)./4.0;
t4028 = (t370.*t3307)./4.0;
t4029 = (t227.*t3524)./4.0;
t4032 = (t12.*t3866)./2.0;
t4056 = (t5.*t14.*t3864)./2.0;
t4057 = (t6.*t13.*t3864)./2.0;
t4058 = (t13.*t14.*t3861)./2.0;
t4098 = -t4074;
t4100 = (t13.*t42.*t3864)./4.0;
t4143 = -t4108;
t4147 = -t4114;
t4150 = -t4117;
t4152 = t420+t1453+t1719;
t4158 = -t4122;
t4159 = (t6.*t4016)./2.0;
t4161 = -t4127;
t4162 = -t4129;
t4165 = -t4132;
t4170 = -t4137;
t4171 = -t4139;
t4172 = -t4140;
t4197 = t106.*2.74179553204116e-4;
t4210 = -t4180;
t4211 = -t4181;
t4212 = -t4182;
t4216 = -t4183;
t4223 = -t4190;
t4224 = (t13.*t14.*t4016)./4.0;
t4228 = -t4199;
t4231 = -t4203;
t4242 = t104.*4.67845486573025e-5;
t4245 = -t4214;
t4246 = -t4215;
t4251 = t269+t295+t865+t1258;
t4255 = t129+t422+t678+t894;
t4259 = -t4232;
t4260 = -t4233;
t4261 = -t4235;
t4265 = t459+t1322+t1662;
t4267 = -t4243;
t4274 = -t4248;
t4286 = t123+t421+t769+t884;
t4290 = -t4270;
t4291 = -t4271;
t4292 = -t4273;
t4293 = (t223.*t3861)./4.0;
t4303 = -t4283;
t4305 = t104.*2.454825983680473e-3;
t4307 = t15.*t223.*1.082026026049065e-3;
t4313 = -t4306;
t4325 = t7.*t223.*2.300122758781553e-3;
t4374 = t336+t374+t1131+t1538;
t4412 = t223.*t4110;
t4422 = (t223.*t4016)./2.0;
t4433 = t15.*t223.*(-5.897280115119475e-3);
t4436 = t2422+t2471;
t4472 = (t5.*t4344)./4.0;
t4474 = t254+t463+t1087+t1239;
t4496 = (t13.*t4365)./2.0;
t4504 = -t4486;
t4508 = -t4491;
t4521 = (t4.*t5.*t4344)./2.0;
t4525 = (t12.*t13.*t4344)./2.0;
t4531 = t676+t1386+t1556;
t4533 = (t9.*t4410)./4.0;
t4535 = t2422.*5.171996702e-3;
t4538 = t2425.*5.171996702e-3;
t4546 = -t5.*(t2425-t2468);
t4547 = -t13.*(t2425-t2468);
t4548 = (t15.*t4415)./4.0;
t4550 = (t5.*t12.*t4365)./2.0;
t4551 = t934+t1144+t1537;
t4553 = (t5.*t4450)./2.0;
t4561 = (t14.*t15.*t4383)./2.0;
t4567 = (t13.*t4447)./2.0;
t4568 = (t7.*t4471)./4.0;
t4569 = t309+t528+t1056+t1250;
t4570 = (t13.*t4470)./4.0;
t4572 = (t8.*t9.*t4410)./2.0;
t4573 = (t16.*t17.*t4410)./2.0;
t4584 = -t30.*(t2425-t2468);
t4587 = t1037+t1186+t1581;
t4590 = -t34.*(t2425-t2468);
t4591 = -t35.*(t2425-t2468);
t4594 = (t6.*t15.*t4415)./2.0;
t4595 = (t7.*t14.*t4415)./2.0;
t4597 = -t42.*(t2425-t2468);
t4598 = (t5.*t4466)./2.0;
t4600 = (t12.*t13.*t4450)./2.0;
t4601 = (t6.*t4494)./2.0;
t4602 = t16.*(-t244+t268+t15.*(t257+t269)+t7.*(t263-t283)).*(-7.35522e-1);
t4604 = t285+t332+t339+t882+t1241;
t4607 = (t15.*t4495)./2.0;
t4608 = (t9.*t16.*t4432)./2.0;
t4610 = (t6.*t4475)./4.0;
t4612 = t16.*(-t244+t268+t15.*(t257+t269)+t7.*(t263-t283)).*(-1.666555);
t4614 = (t8.*t4476)./2.0;
t4617 = (t16.*t4477)./2.0;
t4626 = (t5.*t12.*t4447)./4.0;
t4628 = t2468.*5.171996702e-3;
t4632 = t2471.*5.171996702e-3;
t4634 = (t7.*t14.*t4451)./2.0;
t4636 = (t4.*t13.*t4470)./2.0;
t4637 = (t5.*t12.*t4470)./2.0;
t4641 = (t7.*t4510)./2.0;
t4642 = (t14.*t15.*t4471)./2.0;
t4644 = (t16.*t41.*t4410)./4.0;
t4646 = (t14.*t4512)./2.0;
t4650 = t109.*(t2425-t2468);
t4653 = -t68.*(t2425-t2468);
t4654 = t116.*(t2425-t2468);
t4656 = t4.*t5.*(t2425-t2468);
t4660 = -t47.*(t2425-t2468);
t4661 = (t14.*t43.*t4415)./4.0;
t4664 = t42.*(t2425-t2468);
t4665 = (t12.*t13.*t4466)./4.0;
t4670 = (t6.*t7.*t4471)./2.0;
t4677 = (t7.*t14.*t4495)./4.0;
t4678 = (t13.*t14.*t4494)./4.0;
t4679 = (t5.*t6.*t4475)./2.0;
t4680 = (t6.*t13.*t4473)./2.0;
t4686 = (t13.*t14.*t4475)./2.0;
t4689 = (t17.*t4515)./4.0;
t4690 = (t8.*t15.*t4477)./4.0;
t4691 = (t15.*t16.*t4476)./4.0;
t4701 = t1397+t1429+t1507;
t4708 = (t14.*t15.*t4510)./4.0;
t4709 = (t6.*t13.*t4512)./4.0;
t4714 = (t16.*t17.*t4499)./2.0;
t4716 = (t8.*t4527)./4.0;
t4720 = t55.*(t2425-t2468);
t4721 = t71.*(t2425-t2468);
t4723 = (t16.*t4534)./4.0;
t4733 = (t14.*t37.*t4471)./4.0;
t4736 = (t13.*t35.*t4475)./4.0;
t4737 = (t8.*t17.*t4515)./2.0;
t4738 = (t9.*t16.*t4515)./2.0;
t4742 = (t5.*t4558)./4.0;
t4751 = (t13.*t42.*t4512)./2.0;
t4752 = (t7.*t8.*t4527)./2.0;
t4753 = (t8.*t15.*t4526)./2.0;
t4756 = (t15.*t16.*t4527)./2.0;
t4763 = (t7.*t16.*t4534)./2.0;
t4764 = (t8.*t15.*t4534)./2.0;
t4765 = (t15.*t16.*t4532)./2.0;
t4777 = (t14.*t4624)./2.0;
t4780 = t8.*t2520.*4.38178973375e-3;
t4781 = (t16.*t45.*t4515)./4.0;
t4782 = (t8.*t4635)./4.0;
t4791 = (t583.*t3833)./4.0;
t4793 = (t12.*t13.*t4558)./2.0;
t4799 = (t7.*t4619)./4.0;
t4800 = (t15.*t39.*t4527)./4.0;
t4809 = (t15.*t44.*t4534)./4.0;
t4811 = t14.*t2568.*2.46255173325e-2;
t4819 = (t6.*t4662)./4.0;
t4822 = (t15.*t16.*t4635)./2.0;
t4824 = (t225.*t4415)./4.0;
t4830 = (t14.*t15.*t4619)./2.0;
t4834 = (t6.*t13.*t4624)./4.0;
t4835 = (t229.*t4410)./4.0;
t4842 = (t225.*t4451)./4.0;
t4845 = (t13.*t14.*t4662)./2.0;
t4852 = (t227.*t4477)./4.0;
t4853 = (t228.*t4477)./4.0;
t4854 = t15.*t223.*t4415.*(-1.0./4.0);
t4855 = (t15.*t16.*t4711)./4.0;
t4856 = (t223.*t4494)./4.0;
t4857 = (t225.*t4495)./4.0;
t4858 = (t226.*t4495)./4.0;
t4859 = t1572.*(t1748-t1821).*(-1.0./4.0);
t4861 = (t8.*t15.*t4726)./4.0;
t4862 = (t224.*t4475)./2.0;
t4863 = (t223.*t4475)./4.0;
t4871 = (t1572.*(t1748-t1821))./4.0;
t4874 = (t229.*t4499)./4.0;
t4881 = t7.*t223.*t4471.*(-1.0./4.0);
t4891 = (t227.*t4534)./4.0;
t4892 = (t369.*t4471)./2.0;
t4894 = (t1572.*t3833)./2.0;
t4899 = (t227.*t4526)./4.0;
t4946 = (t223.*t4662)./4.0;
t4966 = (t227.*t4726)./2.0;
t5021 = -t5001;
t5024 = t4.*t4992;
t5026 = t4.*t4994;
t5028 = -t5009;
t5034 = -t4994;
t5066 = -t5027;
t5088 = -t5070;
t5093 = t13.*t3405.*2.01382560198e-1;
t5101 = t5.*t12.*t3405.*4.02765120396e-1;
t5105 = t5.*(t2425-t2468).*(-3.587895);
t5107 = t13.*(t2425-t2468).*(-3.587895);
t5121 = t5.*(t2425-t2468).*(-3.228604);
t5125 = t13.*(t2425-t2468).*(-3.228604);
t5151 = t30.*(t2425-t2468).*(-1.225946);
t5153 = t35.*(t2425-t2468).*(-1.225946);
t5165 = t30.*(t2425-t2468).*(-3.587895);
t5168 = t34.*(t2425-t2468).*(-3.587895);
t5169 = t35.*(t2425-t2468).*(-3.587895);
t5180 = t17.*t3738.*1.13264871585e-2;
t5181 = t9.*t3743.*1.13264871585e-2;
t5190 = t68.*(t2425-t2468).*(-1.225946);
t5193 = t47.*(t2425-t2468).*(-1.225946);
t5194 = t16.*(-t244+t268+t15.*(t257+t269)+t7.*(t263-t283)).*(-5.01208083475e-2);
t5196 = t68.*(t2425-t2468).*(-3.587895);
t5212 = (t536.*t4681)./2.0;
t5214 = t16.*(-t244+t268+t15.*(t257+t269)+t7.*(t263-t283)).*5.01208083475e-2;
t5247 = (t554.*t4681)./4.0;
t5248 = t182+t5046;
t5252 = t4.*(t2425-t2468).*(-9.28985736e-3);
t5262 = t4.*(t2425-t2468).*9.28985736e-3;
t5274 = t863+t1255+t1339+t1509;
t5275 = t899+t1274+t1311+t1481;
t5277 = t1074+t1109+t1321+t1421;
t5281 = t34.*(t2425-t2468).*(-1.8732399795e-1);
t5286 = t30.*(t2425-t2468).*(-9.5384188575e-2);
t5287 = t35.*(t2425-t2468).*(-9.5384188575e-2);
t5290 = t1068+t1346+t1452+t1518;
t5293 = t35.*(t2425-t2468).*9.5384188575e-2;
t5295 = (t536.*t4843)./4.0;
t5299 = t68.*(t2425-t2468).*(-9.5384188575e-2);
t5312 = t1121+t1430+t1533+t1638;
t5314 = t809+t1344+t1691+t1798;
t5319 = (t554.*t4843)./2.0;
t5320 = (t2087.*t4337)./2.0;
t5321 = (t2008.*t4356)./2.0;
t5322 = (t2087.*t4337)./4.0;
t5323 = (t2008.*t4356)./4.0;
t5324 = t8.*t4021.*4.38178973375e-3;
t5334 = t1283+t1427+t1548+t1783;
t5351 = t438+t5051;
t5422 = t4994.*3.228604;
t5423 = t4992.*3.587895;
t5424 = t4994.*3.587895;
t5436 = t4992.*3.228604;
t5445 = (t1572.*t4841)./2.0;
t5446 = (t1490.*t4843)./2.0;
t5450 = t4970+2.081e-3;
t5454 = t5027.*3.587895;
t5456 = t5029.*3.587895;
t5457 = t5027.*1.225946;
t5469 = t13.*t4936.*6.23745e-2;
t5480 = -t5458;
t5510 = t5.*t12.*t4936.*1.24749e-1;
t5525 = (t1572.*t4905)./4.0;
t5526 = (t1920.*t4843)./4.0;
t5538 = t5.*(t2425-t2468).*(-4.4422362436e-2);
t5544 = t13.*(t2425-t2468).*(-6.3364582104e-2);
t5550 = -t5531;
t5557 = t5.*(t2425-t2468).*4.4422362436e-2;
t5562 = t13.*(t2425-t2468).*6.3364582104e-2;
t5565 = t16.*t5069.*2.62925e-3;
t5569 = t12.*(t2425-t2468).*(-1.015997283e-3);
t5571 = t4.*t13.*(t2425-t2468).*(-4.4422362436e-2);
t5572 = t12.*t13.*(t2425-t2468).*(-4.4422362436e-2);
t5576 = t5.*t12.*(t2425-t2468).*(-6.3364582104e-2);
t5587 = t12.*(t2425-t2468).*1.015997283e-3;
t5589 = t4.*t13.*(t2425-t2468).*4.4422362436e-2;
t5591 = t5029.*1.8732399795e-1;
t5593 = t12.*t13.*(t2425-t2468).*4.4422362436e-2;
t5594 = t5027.*9.5384188575e-2;
t5598 = t1889+t1900+t1923+t1926;
t5599 = t5.*t12.*(t2425-t2468).*6.3364582104e-2;
t5620 = t18.*(t2425-t2468).*(-1.130503185e-3);
t5622 = t24.*(t2425-t2468).*(-1.130503185e-3);
t5624 = t47.*(t2425-t2468).*(-2.5171736245e-2);
t5638 = t12.*t13.*t583.*(t2425-t2468).*(-8.9697375e-1);
t5639 = t18.*(t2425-t2468).*1.130503185e-3;
t5641 = t24.*(t2425-t2468).*1.130503185e-3;
t5642 = t47.*(t2425-t2468).*2.5171736245e-2;
t5650 = t6.*t5115.*6.8635e-3;
t5657 = t12.*t13.*t583.*(t2425-t2468).*8.9697375e-1;
t5677 = -t5665;
t5709 = t619+t668+t1162+t1223+t1525;
t5723 = t595+t657+t1183+t1203+t1495;
t5740 = t1832+t5115;
t5761 = t682+t908+t1332+t1337+t1487;
t5763 = t794+t915+t1110+t1357+t1506;
t5776 = t870+t963+t996+t1163+t1524;
t5777 = t748+t978+t1017+t1336+t1555;
t5778 = (t3738.*t4298)./2.0;
t5781 = (t3743.*t4300)./2.0;
t5785 = t999+t1028+t1112+t1299+t1600;
t5787 = t913+t1018+t1232+t1308+t1369;
t5826 = t1750+t1772+t1899+t2970;
t5831 = t839+t1193+t1206+t1535+t1734;
t5833 = t855+t965+t1372+t1563+t1609;
t5834 = t1147+t1242+t1277+t1378+t1472;
t5837 = t1003+t1290+t1331+t1389+t1488;
t5845 = t1041+t1228+t1353+t1573+t1689;
t5847 = t991+t1048+t1571+t1599+t1706;
t5933 = -t5911;
t5966 = (t3243.*t4873)./2.0;
t5967 = (t3261.*t4860)./2.0;
t5971 = t9.*t5433.*1.539925e-2;
t5975 = t17.*t5434.*1.539925e-2;
t6024 = (t3249.*t4900)./2.0;
t6025 = (t3265.*t4884)./2.0;
t6035 = (t3243.*t4908)./4.0;
t6036 = (t3318.*t4860)./4.0;
t6046 = t2813+t5069;
t6071 = t3261.*(t2798-t2848).*(-1.0./4.0);
t6072 = (t4873.*(t881-t912))./4.0;
t6084 = (t3249.*t4939)./4.0;
t6085 = (t3360.*t4884)./4.0;
t6090 = (t3318.*t4906)./2.0;
t6091 = (t3316.*t4908)./2.0;
t6093 = (t3266.*(t2821-t2864))./4.0;
t6094 = (t4879.*(t943-t1091))./4.0;
t6107 = (t4908.*(t881-t912))./2.0;
t6108 = t3318.*(t2798-t2848).*(-1.0./2.0);
t6109 = (t4908.*(t881-t912))./4.0;
t6110 = t3318.*(t2798-t2848).*(-1.0./4.0);
t6112 = (t3424.*t4879)./2.0;
t6116 = (t3421.*t4896)./4.0;
t6124 = (t3318.*(t2798-t2848))./2.0;
t6126 = (t3318.*(t2798-t2848))./4.0;
t6130 = (t4917.*(t943-t1091))./2.0;
t6131 = (t3362.*(t2821-t2864))./2.0;
t6133 = (t3489.*t4896)./2.0;
t6137 = (t3356.*t4936)./2.0;
t6138 = (t3405.*t4922)./2.0;
t6145 = (t3396.*t4916)./2.0;
t6146 = (t3350.*t4930)./2.0;
t6155 = t3316+t5011;
t6159 = t3318+t5015;
t6160 = (t3424.*t4917)./4.0;
t6168 = -t6149;
t6169 = -t6150;
t6182 = (t3421.*t4938)./2.0;
t6183 = (t3365.*(t2904-t2927))./2.0;
t6187 = (t3489.*t4938)./4.0;
t6197 = (t3421.*(t2889-t2921))./2.0;
t6198 = (t3455.*(t2904-t2927))./2.0;
t6205 = t3356+t5046;
t6213 = t12.*t3243.*(t2425-t2468).*(-8.07151e-1);
t6216 = t3396+t5051;
t6222 = t1751+t1864+t2794+t2969;
t6225 = t12.*t3261.*(t2425-t2468).*(-8.07151e-1);
t6239 = t12.*t3261.*(t2425-t2468).*8.07151e-1;
t6243 = (t3752.*t4900)./4.0;
t6253 = (t2054.*t5433)./2.0;
t6256 = t12.*t3316.*(t2425-t2468).*(-8.07151e-1);
t6257 = t4.*t3318.*(t2425-t2468).*(-8.07151e-1);
t6259 = t12.*t3318.*(t2425-t2468).*(-8.07151e-1);
t6261 = (t2044.*t5434)./2.0;
t6273 = t12.*(t881-t912).*(t2425-t2468).*(-8.07151e-1);
t6274 = t12.*t3318.*(t2425-t2468).*8.07151e-1;
t6280 = (t3752.*t4939)./2.0;
t6300 = t12.*t13.*t3350.*(t2425-t2468).*(-8.07151e-1);
t6309 = t4337.*(t2425-t2468).*(-1.0./4.0);
t6317 = t12.*t13.*t3350.*(t2425-t2468).*8.07151e-1;
t6319 = t5.*t12.*t3405.*(t2425-t2468).*(-8.07151e-1);
t6324 = t4356.*(t2425-t2468).*(-1.0./4.0);
t6333 = t14.*t5750.*6.8635e-3;
t6337 = t5.*t12.*t3405.*(t2425-t2468).*8.07151e-1;
t6479 = (t3266.*t5331)./2.0;
t6513 = (t4021.*t5069)./2.0;
t6514 = -t8.*(t30.*(t2425-t2468)+t68.*(t2425-t2468));
t6515 = -t16.*(t30.*(t2425-t2468)+t68.*(t2425-t2468));
t6519 = t12.*t13.*t4681.*(t2425-t2468).*(-1.0./4.0);
t6520 = (t3362.*t5331)./4.0;
t6529 = (t12.*t13.*t4681.*(t2425-t2468))./4.0;
t6530 = t12.*t3261.*t4959.*8.07151e-1;
t6545 = (t3365.*t5365)./4.0;
t6561 = t8.*t6069.*2.62925e-3;
t6578 = t12.*t4860.*(t2425-t2468).*(-1.0./4.0);
t6580 = (t3265.*t5443)./4.0;
t6586 = t12.*t4873.*(t2425-t2468).*(-1.0./4.0);
t6597 = (t12.*t4873.*(t2425-t2468))./4.0;
t6606 = (t3360.*t5443)./2.0;
t6609 = t12.*t4906.*(t2425-t2468).*(-1.0./4.0);
t6611 = t4.*t4908.*(t2425-t2468).*(-1.0./4.0);
t6614 = t12.*t4908.*(t2425-t2468).*(-1.0./4.0);
t6621 = (t12.*t4908.*(t2425-t2468))./4.0;
t6622 = (t12.*(t2425-t2468).*(t2798-t2848))./4.0;
t6643 = t12.*t13.*t4916.*(t2425-t2468).*(-1.0./4.0);
t6646 = t5772+1.0343993404e-2;
t6647 = t5.*t12.*t4936.*(t2425-t2468).*(-1.0./4.0);
t6655 = (t12.*t13.*t4916.*(t2425-t2468))./4.0;
t6658 = (t5.*t12.*t4936.*(t2425-t2468))./4.0;
t6684 = (t3743.*t5448)./2.0;
t6685 = (t3767.*t5433)./2.0;
t6694 = (t3738.*t5449)./2.0;
t6695 = (t3763.*t5434)./2.0;
t6710 = (t3752.*t5442)./2.0;
t6711 = (t3771.*t5443)./2.0;
t6762 = t1745+t1853+t1891+t2869+t2960;
t6763 = t1839+t1850+t1871+t2805+t2956;
t6839 = (t4021.*t5430)./2.0;
t6928 = t2858+t2898+t2992+t3135;
t6950 = t8.*(t30.*(t2425-t2468)+t68.*(t2425-t2468)).*(-7.35522e-1);
t6952 = t8.*(t30.*(t2425-t2468)+t68.*(t2425-t2468)).*(-1.666555);
t6955 = t16.*(t30.*(t2425-t2468)+t68.*(t2425-t2468)).*(-1.666555);
t6960 = (t12.*t4873.*t4959)./4.0;
t6966 = t2888+t3000+t3072+t3081;
t6969 = t2938+t2978+t3050+t3104;
t7002 = t5750.*(t263-t283-t310+t1265).*(-1.0./4.0);
t7145 = t18.*t4959.*(t2425-t2468).*(-3.23463e-1);
t7153 = t24.*t4959.*(t2425-t2468).*(-1.937765);
t7161 = t18.*t4959.*(t2425-t2468).*3.23463e-1;
t7166 = t24.*t4959.*(t2425-t2468).*1.937765;
t7206 = (t6092.*(t943-t1091))./4.0;
t7210 = t183+t4992+t5045;
t7233 = (t3421.*t6104)./4.0;
t7237 = t194+t4994+t5076;
t7248 = (t4337.*t5681)./2.0;
t7249 = (t4337.*t5681)./4.0;
t7274 = (t3732.*t6069)./2.0;
t7344 = t433+t4992+t5045;
t7383 = t8.*(t30.*(t2425-t2468)+t68.*(t2425-t2468)).*(-5.01208083475e-2);
t7386 = t4906+t5451;
t7389 = t4908+t5437;
t7392 = t14.*(t30.*(t2425-t2468)+t68.*(t2425-t2468)).*(-2.46255173325e-2);
t7395 = t16.*(t30.*(t2425-t2468)+t68.*(t2425-t2468)).*(-1.17633784675e-2);
t7405 = t14.*(t30.*(t2425-t2468)+t68.*(t2425-t2468)).*2.46255173325e-2;
t7422 = t4922+t5485;
t7428 = t4930+t5486;
t7437 = t5759.*(t2425-t2468).*(-1.0./4.0);
t7443 = t5772.*(t2425-t2468).*(-1.0./4.0);
t7444 = (t5759.*(t2425-t2468))./4.0;
t7468 = t5795.*(t2425-t2468).*(-1.0./4.0);
t7620 = t1443+t4992+t5045;
t7656 = t1460+t4994+t5076;
t7665 = t4.*t5530.*(t2425-t2468).*(-1.617315e-1);
t7667 = t12.*t5535.*(t2425-t2468).*(-1.617315e-1);
t7681 = t4.*t5530.*(t2425-t2468).*1.617315e-1;
t7683 = t12.*t5535.*(t2425-t2468).*1.617315e-1;
t7734 = t1920+t4994+t5076;
t7852 = t14.*(t30.*(t2425-t2468).*3.587895+t68.*(t2425-t2468).*3.587895).*(-6.8635e-3);
t7865 = t14.*(t30.*(t2425-t2468).*3.587895+t68.*(t2425-t2468).*3.587895).*6.8635e-3;
t7887 = (t5062.*t5772)./2.0;
t7956 = t6338.*(t2425-t2468).*(-1.0./4.0);
t7966 = (t6338.*(t2425-t2468))./4.0;
t8015 = t4.*t4959.*t5530.*3.23463e-1;
t8017 = t12.*t4959.*t5535.*3.23463e-1;
t8108 = (t2008.*t7362)./2.0;
t8109 = (t2008.*t7362)./4.0;
t8155 = t4.*t6481.*(t2425-t2468).*(-1.0./4.0);
t8156 = t3350+t4992+t5045;
t8159 = t12.*t6483.*(t2425-t2468).*(-1.0./4.0);
t8169 = (t4.*t6481.*(t2425-t2468))./4.0;
t8171 = (t12.*t6483.*(t2425-t2468))./4.0;
t8321 = t6338.*(t2959-t2967).*(-1.0./2.0);
t8327 = (t6338.*(t2959-t2967))./2.0;
t8423 = (t30.*(t2425-t2468)+t68.*(t2425-t2468)).*(t2821-t2864).*(-1.0./4.0);
t8428 = ((t30.*(t2425-t2468)+t68.*(t2425-t2468)).*(t2821-t2864))./4.0;
t8442 = (t4.*t4959.*t6481)./2.0;
t8444 = (t943-t1091).*(t30.*(t2425-t2468).*1.225946+t68.*(t2425-t2468).*1.225946).*(-1.0./4.0);
t8445 = (t12.*t4959.*t6483)./2.0;
t8450 = ((t943-t1091).*(t30.*(t2425-t2468).*1.225946+t68.*(t2425-t2468).*1.225946))./4.0;
t8453 = t3424.*(t30.*(t2425-t2468).*1.225946+t68.*(t2425-t2468).*1.225946).*(-1.0./4.0);
t8470 = (t5681.*t5795)./2.0;
t8683 = t5331.*(t30.*(t2425-t2468)+t68.*(t2425-t2468)).*(-1.0./4.0);
t8797 = t7362.*(t2425-t2468).*(-1.0./4.0);
t8811 = (t7362.*(t2425-t2468))./4.0;
t8940 = t13.*(-t3405+t4994+t5076).*(-2.01382560198e-1);
t8969 = t5.*t12.*(-t3405+t4994+t5076).*(-2.01382560198e-1);
t9031 = t7362.*(t2959-t2967).*(-1.0./2.0);
t9033 = (t7362.*(t2959-t2967))./2.0;
t9451 = t4922.*(-t3405+t4994+t5076).*(-1.0./4.0);
t9540 = t5.*t12.*(t2425-t2468).*(-t3405+t4994+t5076).*8.07151e-1;
t380 = t7.*t348;
t381 = t7.*t354;
t384 = t7.*t319;
t385 = t8.*t319;
t386 = t8.*t320;
t387 = -t348;
t388 = t8.*t322;
t389 = t9.*t321;
t390 = t9.*t324;
t391 = t15.*t319;
t392 = t16.*t319;
t393 = t16.*t320;
t394 = t16.*t322;
t395 = t17.*t321;
t396 = -t357;
t397 = t17.*t324;
t416 = -t383;
t423 = t9.*t403;
t424 = t17.*t403;
t426 = t348.*(1.1e+1./1.25e+2);
t427 = t349.*(1.1e+1./1.25e+2);
t430 = t354.*(1.1e+1./1.25e+2);
t431 = t355.*(1.1e+1./1.25e+2);
t439 = t75+t355;
t440 = t49+t352;
t443 = t82.*t354;
t446 = t82.*t319;
t450 = t90.*t319;
t454 = t56+t353;
t455 = -t434;
t456 = -t435;
t465 = t8.*t435;
t469 = t16.*t435;
t471 = t81+t349;
t472 = t120+t358;
t473 = t131+t289;
t474 = t413.*(1.1e+1./1.25e+2);
t475 = t147.*t321;
t476 = t163.*t321;
t480 = -t453;
t482 = t115+t347;
t495 = -t464;
t499 = -t468;
t503 = t9.*t457;
t504 = t9.*t458;
t505 = t17.*t457;
t506 = t17.*t458;
t513 = -t479;
t518 = -t8.*(t69-t347);
t521 = -t16.*(t69-t347);
t523 = -t9.*(t48-t349);
t527 = -t17.*(t48-t349);
t529 = t283+t298;
t534 = -t488;
t538 = t237+t360;
t539 = t104+t413;
t540 = t114+t410;
t541 = -t514;
t557 = t175+t409;
t558 = t174+t414;
t565 = -t547;
t571 = t88+t441;
t574 = t96+t442;
t580 = t16.*(t69-t347).*(-1.1e+1./1.25e+2);
t584 = -t9.*(t113-t409);
t585 = -t17.*(t113-t409);
t618 = t9.*(t113-t409);
t620 = t8.*t573;
t624 = t16.*t573;
t1462 = t8.*t860;
t1475 = t16.*t860;
t1510 = t8.*t887;
t1540 = t16.*t887;
t1777 = -t1474;
t1829 = -t1740;
t1852 = -t1774;
t1855 = -t1788;
t1883 = t353.*2.9474e-2;
t1911 = t352.*1.2516e-2;
t1915 = t356.*1.2516e-2;
t1916 = t357.*1.2516e-2;
t1917 = t358.*1.2516e-2;
t1930 = t347.*3.8437e-2;
t1932 = t353.*3.8437e-2;
t1936 = t138+t148+t263+t280;
t1937 = t159+t164+t231+t284;
t1942 = t348.*4.815e-3;
t1943 = t349.*4.815e-3;
t1945 = t347.*3.5549e-2;
t1947 = t354.*4.815e-3;
t1948 = t355.*4.815e-3;
t1950 = -t1931;
t1952 = t348.*6.0149e-2;
t1953 = t349.*6.0149e-2;
t1955 = t353.*6.0149e-2;
t1956 = t354.*6.0149e-2;
t1957 = t355.*6.0149e-2;
t1959 = t347.*4.1065e-2;
t1960 = t383.*1.2516e-2;
t1963 = t323.*t587;
t1968 = t348.*4.354e-3;
t1969 = t349.*4.354e-3;
t1971 = t354.*4.354e-3;
t1972 = t355.*4.354e-3;
t1973 = t350.*6.1597e-2;
t1974 = t351.*6.1597e-2;
t1975 = t352.*6.1597e-2;
t1976 = t356.*6.1597e-2;
t1977 = t357.*6.1597e-2;
t1978 = t358.*6.1597e-2;
t1980 = t353.*5.433e-3;
t1982 = t348.*1.964e-3;
t1983 = t349.*1.964e-3;
t1985 = t354.*1.964e-3;
t1986 = t355.*1.964e-3;
t1987 = t348.*4.252e-3;
t1988 = t349.*4.252e-3;
t1989 = t352.*4.252e-3;
t1991 = t353.*1.1953e-2;
t1992 = t354.*4.252e-3;
t1993 = t355.*4.252e-3;
t1994 = t356.*4.252e-3;
t1995 = t357.*4.252e-3;
t1996 = t358.*4.252e-3;
t1997 = t348.*1.4117e-2;
t1998 = t349.*1.4117e-2;
t2000 = t353.*1.4117e-2;
t2001 = t354.*1.4117e-2;
t2002 = t355.*1.4117e-2;
t2004 = t350.*4.28e-4;
t2005 = t351.*4.28e-4;
t2006 = t352.*4.28e-4;
t2010 = t348.*1.196e-3;
t2011 = t349.*1.196e-3;
t2012 = t352.*1.196e-3;
t2013 = t356.*4.28e-4;
t2014 = t357.*4.28e-4;
t2015 = t358.*4.28e-4;
t2016 = t9.*t323.*(-1.2516e-2);
t2017 = t348.*1.0517e-2;
t2018 = t349.*1.0517e-2;
t2019 = t350.*1.0517e-2;
t2020 = t351.*1.0517e-2;
t2021 = t352.*1.0517e-2;
t2023 = t347.*2.117e-3;
t2025 = t354.*1.196e-3;
t2026 = t355.*1.196e-3;
t2027 = t356.*1.196e-3;
t2028 = t357.*1.196e-3;
t2029 = t358.*1.196e-3;
t2031 = t354.*1.0517e-2;
t2032 = t355.*1.0517e-2;
t2033 = t358.*1.0517e-2;
t2035 = t353.*2.117e-3;
t2037 = t347.*4.037e-3;
t2039 = t353.*6.4725936e-2;
t2041 = t348.*1.158e-3;
t2042 = t349.*1.158e-3;
t2046 = t353.*1.158e-3;
t2047 = t354.*1.158e-3;
t2048 = t355.*1.158e-3;
t2050 = t350.*1.0027e-2;
t2051 = t351.*1.0027e-2;
t2052 = t352.*1.0027e-2;
t2055 = t358.*1.0027e-2;
t2062 = t321.*t608;
t2066 = t354.*7.41e-4;
t2067 = t355.*7.41e-4;
t2068 = t358.*7.41e-4;
t2079 = t321.*t660;
t2081 = t410.*1.2516e-2;
t2094 = t348.*3.41e-4;
t2095 = t349.*3.41e-4;
t2101 = t353.*3.41e-4;
t2102 = t354.*3.41e-4;
t2103 = t355.*3.41e-4;
t2106 = t7.*t1935;
t2109 = t321.*t631;
t2112 = t382.*6.1597e-2;
t2113 = t15.*t1935;
t2117 = t353.*2.29e-4;
t2119 = t383.*6.1597e-2;
t2122 = t9.*t323.*6.1597e-2;
t2126 = t17.*t323.*6.1597e-2;
t2130 = t16.*t321.*(-4.815e-3);
t2132 = t348.*7.41e-4;
t2133 = t349.*7.41e-4;
t2134 = t350.*7.41e-4;
t2135 = t351.*7.41e-4;
t2136 = t352.*7.41e-4;
t2139 = t321.*t768;
t2143 = t383.*4.252e-3;
t2150 = t323.*t775;
t2154 = t321.*t783;
t2157 = t382.*4.28e-4;
t2159 = t321.*t790;
t2164 = t383.*4.28e-4;
t2169 = t382.*1.0517e-2;
t2170 = t348.*1.09e-4;
t2171 = t349.*1.09e-4;
t2173 = t323.*t798;
t2177 = t383.*1.196e-3;
t2178 = t354.*1.09e-4;
t2179 = t355.*1.09e-4;
t2183 = t323.*t687;
t2186 = t323.*t689;
t2190 = t321.*t692;
t2198 = t321.*t695;
t2203 = t321.*t700;
t2206 = t323.*t701;
t2215 = t321.*t726;
t2217 = t382.*1.0027e-2;
t2218 = t16.*t321.*(-4.354e-3);
t2224 = t413.*4.815e-3;
t2231 = t323.*t751;
t2236 = t477+t491;
t2239 = t321.*t905;
t2242 = t323.*t906;
t2244 = t8.*t321.*(-1.964e-3);
t2247 = t9.*t323.*(-4.252e-3);
t2253 = t8.*t321.*(-1.4117e-2);
t2264 = t9.*t323.*(-1.196e-3);
t2266 = t17.*t323.*(-4.28e-4);
t2267 = t413.*4.354e-3;
t2274 = t16.*t321.*(-1.196e-3);
t2280 = t321.*t818;
t2284 = t410.*6.1597e-2;
t2290 = t414.*6.1597e-2;
t2293 = t8.*t321.*(-1.158e-3);
t2309 = t382.*7.41e-4;
t2312 = t413.*6.0149e-2;
t2316 = t413.*4.252e-3;
t2319 = t409.*1.4117e-2;
t2322 = t410.*4.28e-4;
t2325 = t410.*1.196e-3;
t2326 = t414.*4.28e-4;
t2327 = t409.*1.0517e-2;
t2331 = t413.*1.196e-3;
t2335 = t413.*1.0517e-2;
t2336 = t414.*1.0517e-2;
t2340 = t321.*t1161;
t2344 = t321.*t957;
t2346 = t409.*1.158e-3;
t2350 = t16.*t321.*(-3.41e-4);
t2352 = t414.*1.0027e-2;
t2354 = t434.*1.666555;
t2355 = -t2292;
t2359 = -t2301;
t2360 = t434.*1.225946;
t2361 = -t2307;
t2362 = t409.*1.964e-3;
t2364 = t435.*1.225946;
t2365 = -t2310;
t2366 = t410.*4.252e-3;
t2375 = t452.*7.35522e-1;
t2378 = t413.*3.41e-4;
t2379 = t453.*7.35522e-1;
t2389 = t413.*7.41e-4;
t2390 = t414.*7.41e-4;
t2397 = t409.*1.09e-4;
t2399 = t413.*1.09e-4;
t2402 = t462.*7.35522e-1;
t2406 = t466.*7.35522e-1;
t2410 = t464.*1.666555;
t2413 = t468.*1.666555;
t2417 = t464.*1.225946;
t2419 = t468.*1.225946;
t2432 = -t2407;
t2433 = t477.*1.666555;
t2436 = t477.*1.225946;
t2439 = t479.*1.225946;
t2446 = t490.*7.35522e-1;
t2447 = t493.*7.35522e-1;
t2449 = t491.*1.666555;
t2453 = t488.*1.225946;
t2455 = t491.*1.225946;
t2459 = -t2441;
t2464 = t508.*7.35522e-1;
t2469 = t507.*1.666555;
t2470 = t508.*1.666555;
t2472 = t509.*1.666555;
t2473 = t510.*1.666555;
t2475 = -t2451;
t2476 = t514.*1.666555;
t2477 = -t2452;
t2478 = t507.*1.225946;
t2481 = t509.*1.225946;
t2483 = t511.*1.225946;
t2484 = -t2457;
t2485 = t514.*1.225946;
t2487 = -t2460;
t2491 = t9.*(t48-t349).*(-1.2516e-2);
t2493 = t17.*(t48-t349).*(-1.2516e-2);
t2517 = t16.*(t69-t347).*(-4.815e-3);
t2526 = -t2503;
t2535 = t16.*(t69-t347).*(-4.354e-3);
t2536 = t547.*1.666555;
t2541 = t545.*1.225946;
t2544 = t9.*(t48-t349).*(-6.1597e-2);
t2547 = t547.*1.225946;
t2551 = t17.*(t48-t349).*(-6.1597e-2);
t2552 = t608.*(t69-t347);
t2555 = -t2521;
t2558 = t16.*(t69-t347).*(-6.0149e-2);
t2562 = t8.*(t69-t347).*(-1.0517e-2);
t2564 = t16.*(t69-t347).*(-1.196e-3);
t2565 = t9.*(t48-t349).*(-1.196e-3);
t2567 = t17.*(t48-t349).*(-4.28e-4);
t2570 = t16.*(t69-t347).*(-1.0517e-2);
t2572 = t9.*(t48-t349).*(-1.0517e-2);
t2576 = t17.*(t48-t349).*(-1.196e-3);
t2577 = t550.*1.666555;
t2580 = t17.*(t48-t349).*(-1.0517e-2);
t2584 = t8.*(t69-t347).*(-1.158e-3);
t2585 = t631.*(t69-t347);
t2590 = t548.*1.225946;
t2594 = t550.*1.225946;
t2598 = t9.*(t48-t349).*(-1.0027e-2);
t2603 = t9.*(t48-t349).*6.1597e-2;
t2604 = t17.*(t48-t349).*(-1.0027e-2);
t2606 = t17.*(t48-t349).*6.1597e-2;
t2609 = t8.*(t69-t347).*(-1.964e-3);
t2614 = t660.*(t69-t347);
t2617 = t16.*(t69-t347).*(-4.252e-3);
t2618 = t9.*(t48-t349).*(-4.252e-3);
t2620 = t8.*(t69-t347).*(-1.4117e-2);
t2623 = t17.*(t48-t349).*(-4.252e-3);
t2629 = t9.*(t48-t349).*(-4.28e-4);
t2632 = t695.*(t69-t347);
t2633 = t687.*(t48-t349);
t2635 = t700.*(t69-t347);
t2637 = t16.*(t69-t347).*(-3.41e-4);
t2644 = t740.*(t48-t349);
t2651 = -t2608;
t2653 = t16.*(t69-t347).*(-7.41e-4);
t2655 = t9.*(t48-t349).*(-7.41e-4);
t2658 = t17.*(t48-t349).*(-7.41e-4);
t2661 = t783.*(t69-t347);
t2662 = t775.*(t48-t349);
t2667 = t798.*(t48-t349);
t2688 = t8.*(t69-t347).*(-1.09e-4);
t2690 = t16.*(t69-t347).*(-1.09e-4);
t2708 = t957.*(t69-t347);
t2741 = t17.*(t113-t409).*(-6.1597e-2);
t2757 = t602.*7.35522e-1;
t2773 = t602.*1.666555;
t2776 = t603.*1.666555;
t2790 = t17.*(t113-t409).*(-1.0027e-2);
t2791 = t17.*(t113-t409).*6.1597e-2;
t2833 = t17.*(t113-t409).*(-4.28e-4);
t2837 = t17.*(t113-t409).*(-1.0517e-2);
t2871 = t17.*(t113-t409).*(-7.41e-4);
t2884 = -t2808;
t2885 = (t319.*t2111)./4.0;
t2886 = (t320.*t2111)./4.0;
t3146 = -t3029;
t3198 = t1461.*1.666555;
t3204 = t1474.*1.666555;
t3227 = t1461.*7.35522e-1;
t3268 = t150+t187+t492+t509;
t3269 = t151+t186+t489+t511;
t3270 = t317+t2561;
t3291 = t347.*4.7121686402e-2;
t3294 = t353.*4.7121686402e-2;
t3312 = -t3293;
t3328 = t347.*5.034347249e-2;
t3330 = t135+t214+t507+t537;
t3338 = t350.*4.5305948634e-2;
t3339 = t351.*4.5305948634e-2;
t3340 = t352.*4.5305948634e-2;
t3344 = t356.*4.5305948634e-2;
t3345 = t357.*4.5305948634e-2;
t3346 = t358.*4.5305948634e-2;
t3361 = -t3323;
t3363 = t354.*1.7527158935e-2;
t3364 = t355.*1.7527158935e-2;
t3367 = t354.*3.127439544e-3;
t3368 = t355.*3.127439544e-3;
t3369 = t356.*3.127439544e-3;
t3370 = t357.*3.127439544e-3;
t3371 = t358.*3.127439544e-3;
t3372 = t348.*7.735484874e-3;
t3373 = t349.*7.735484874e-3;
t3374 = t350.*7.735484874e-3;
t3375 = t351.*7.735484874e-3;
t3376 = t352.*7.735484874e-3;
t3378 = t354.*7.735484874e-3;
t3379 = t355.*7.735484874e-3;
t3380 = t358.*7.735484874e-3;
t3381 = t348.*1.00241616695e-1;
t3382 = t349.*1.00241616695e-1;
t3383 = t4.*t3314;
t3387 = t353.*1.00241616695e-1;
t3388 = t354.*1.00241616695e-1;
t3389 = t355.*1.00241616695e-1;
t3400 = t353.*1.4653732538e-2;
t3410 = t348.*2.3526756935e-2;
t3411 = t349.*2.3526756935e-2;
t3412 = t348.*1.7527158935e-2;
t3413 = t349.*1.7527158935e-2;
t3415 = t353.*2.3526756935e-2;
t3416 = t354.*2.3526756935e-2;
t3417 = t355.*2.3526756935e-2;
t3418 = t348.*3.127439544e-3;
t3419 = t349.*3.127439544e-3;
t3420 = t352.*3.127439544e-3;
t3432 = t382.*4.5305948634e-2;
t3435 = t383.*4.5305948634e-2;
t3437 = t9.*t323.*4.5305948634e-2;
t3442 = -t3393;
t3444 = t17.*t323.*4.5305948634e-2;
t3450 = -t3402;
t3463 = t16.*t321.*1.7527158935e-2;
t3467 = t321.*t2771;
t3477 = t321.*t2777;
t3480 = t323.*t2778;
t3484 = -t3430;
t3495 = t321.*t2785;
t3504 = -t9.*(t166+t205+t514+t533);
t3509 = -t17.*(t166+t205+t514+t533);
t3529 = t321.*t2762;
t3531 = t383.*3.127439544e-3;
t3534 = t8.*t321.*1.7527158935e-2;
t3538 = t382.*7.735484874e-3;
t3545 = t323.*t2769;
t3556 = t410.*4.5305948634e-2;
t3564 = t414.*4.5305948634e-2;
t3568 = -t3491;
t3570 = -t3493;
t3579 = -t3511;
t3591 = t8.*t321.*(-2.3526756935e-2);
t3597 = t9.*t323.*(-3.127439544e-3);
t3601 = t4.*t3482;
t3603 = t413.*1.00241616695e-1;
t3608 = -t3557;
t3624 = t9.*(t166+t205+t514+t533);
t3639 = t409.*2.3526756935e-2;
t3640 = t409.*1.7527158935e-2;
t3644 = t410.*3.127439544e-3;
t3646 = t413.*1.7527158935e-2;
t3650 = t413.*3.127439544e-3;
t3654 = t413.*7.735484874e-3;
t3655 = t414.*7.735484874e-3;
t3663 = -t3604;
t3664 = -t3606;
t3673 = -t3633;
t3679 = -t3642;
t3691 = -t3662;
t3710 = t434.*7.326866269e-3;
t3713 = -t3694;
t3716 = t435.*2.5171736245e-2;
t3720 = t126+t176+t315+t342+t372+t407;
t3731 = -t3712;
t3742 = t338+t362+t375+t408+t433;
t3744 = -t3721;
t3755 = t462.*3.867742437e-3;
t3757 = -t3734;
t3759 = t244+t304+t546+t549;
t3769 = -t3747;
t3774 = -t3751;
t3777 = t466.*1.563719772e-3;
t3778 = -t3753;
t3779 = (t321.*t3106)./4.0;
t3781 = t479.*2.5171736245e-2;
t3783 = -t3756;
t3784 = t259+t296+t551+t564;
t3788 = -t3765;
t3791 = t477.*7.326866269e-3;
t3795 = -t3772;
t3798 = t488.*2.5171736245e-2;
t3802 = t223.*t3323;
t3804 = t493.*3.867742437e-3;
t3806 = -t3782;
t3813 = t491.*7.326866269e-3;
t3818 = -t3792;
t3821 = -t3794;
t3824 = t17.*(t48-t349).*(-4.5305948634e-2);
t3828 = t490.*1.563719772e-3;
t3829 = -t3799;
t3830 = -t3800;
t3831 = (t325.*t3219)./4.0;
t3832 = -t3801;
t3834 = t511.*2.5171736245e-2;
t3835 = t508.*5.01208083475e-2;
t3838 = -t3811;
t3842 = -t3815;
t3847 = t514.*7.326866269e-3;
t3850 = t9.*(t48-t349).*(-4.5305948634e-2);
t3852 = t17.*(t48-t349).*4.5305948634e-2;
t3856 = t510.*1.17633784675e-2;
t3867 = t8.*(t69-t347).*(-2.3526756935e-2);
t3868 = t8.*(t69-t347).*(-1.7527158935e-2);
t3873 = t16.*(t69-t347).*(-1.7527158935e-2);
t3876 = t16.*(t69-t347).*(-3.127439544e-3);
t3877 = t9.*(t48-t349).*(-3.127439544e-3);
t3881 = t17.*(t48-t349).*(-3.127439544e-3);
t3883 = t16.*(t69-t347).*(-7.735484874e-3);
t3885 = t9.*(t48-t349).*(-7.735484874e-3);
t3889 = t17.*(t48-t349).*(-7.735484874e-3);
t3891 = -t3843;
t3892 = -t3844;
t3895 = t16.*(t69-t347).*(-1.00241616695e-1);
t3900 = t9.*(t48-t349).*4.5305948634e-2;
t3904 = -t3857;
t3907 = -t3869;
t3910 = t223.*t3430;
t3911 = t2771.*(t69-t347);
t3912 = t2769.*(t48-t349);
t3914 = t2777.*(t69-t347);
t3918 = (t321.*t3247)./4.0;
t3919 = (t322.*t3247)./4.0;
t3922 = t2785.*(t69-t347);
t3926 = t545.*2.5171736245e-2;
t3927 = (t403.*t3173)./4.0;
t3928 = (t321.*t3277)./4.0;
t3930 = -t3905;
t3933 = -t3909;
t3938 = t547.*7.326866269e-3;
t3947 = (t319.*t3264)./4.0;
t3948 = -t3920;
t3955 = (t321.*t3299)./4.0;
t3956 = t325.*(t689-t740).*(-1.0./4.0);
t3957 = t326.*(t689-t740).*(-1.0./4.0);
t3959 = t550.*7.326866269e-3;
t3974 = t548.*2.5171736245e-2;
t3976 = (t323.*t3317)./4.0;
t3980 = (t325.*(t689-t740))./4.0;
t3981 = (t326.*(t689-t740))./4.0;
t3982 = -t3958;
t3985 = (t319.*t3321)./2.0;
t3986 = (t320.*t3321)./4.0;
t3987 = -t3961;
t3989 = -t3964;
t3990 = (t323.*t3304)./4.0;
t3992 = -t3971;
t3993 = (t323.*t3307)./4.0;
t3994 = (t324.*t3307)./4.0;
t3998 = (t405.*t3239)./4.0;
t3999 = (t325.*(t1130-t16.*t17.*1.2516e-2))./4.0;
t4008 = (t319.*t3359)./4.0;
t4010 = (t16.*t321.*t3286)./4.0;
t4011 = t17.*(t113-t409).*(-4.5305948634e-2);
t4020 = -t4003;
t4023 = t17.*(t113-t409).*(-7.735484874e-3);
t4024 = t948+t2501;
t4033 = t17.*(t113-t409).*4.5305948634e-2;
t4036 = (t404.*t3296)./4.0;
t4037 = (t323.*t3441)./4.0;
t4039 = -t4022;
t4042 = (t404.*t3286)./4.0;
t4043 = (t323.*t3453)./4.0;
t4045 = -t4027;
t4046 = -t4029;
t4053 = t403.*(t733-t806).*(-1.0./4.0);
t4054 = (t321.*(t1355-t15.*t16.*1.158e-3))./4.0;
t4065 = t602.*5.01208083475e-2;
t4077 = -t4056;
t4078 = -t4057;
t4081 = t603.*1.17633784675e-2;
t4144 = t3239.*(t79-t358).*(-1.0./4.0);
t4164 = t3247.*(t69-t347).*(-1.0./4.0);
t4192 = t3280.*(t79-t358).*(-1.0./4.0);
t4200 = (t3247.*(t69-t347))./4.0;
t4225 = t1461.*5.01208083475e-2;
t4227 = -t4197;
t4244 = t3296.*(t48-t349).*(-1.0./4.0);
t4252 = t502+t872+t1404;
t4266 = -t4242;
t4268 = t1474.*1.17633784675e-2;
t4281 = t3329.*(t48-t349).*(-1.0./4.0);
t4302 = (t3329.*(t48-t349))./4.0;
t4308 = t353.*1.082026026049065e-3;
t4314 = t3447.*(t79-t358).*(-1.0./4.0);
t4315 = -t4307;
t4318 = t348.*1.037589172186849e-4;
t4319 = (t320.*t3864)./2.0;
t4320 = (t319.*t3864)./4.0;
t4322 = t3524.*(t48-t349).*(-1.0./4.0);
t4326 = t347.*2.300122758781553e-3;
t4331 = (t3447.*(t79-t358))./4.0;
t4340 = (t3524.*(t48-t349))./4.0;
t4342 = -t4325;
t4345 = ((t106-t414).*(t689-t740))./4.0;
t4347 = t356.*8.36241330891889e-4;
t4348 = t357.*8.36241330891889e-4;
t4353 = t350.*2.74179553204116e-4;
t4354 = t351.*2.74179553204116e-4;
t4357 = t3307.*(t113-t409).*(-1.0./4.0);
t4364 = t354.*9.3569097314605e-5;
t4372 = t17.*t323.*2.74179553204116e-4;
t4375 = t8.*t321.*5.187945860934245e-5;
t4377 = (t3307.*(t113-t409))./4.0;
t4388 = t383.*8.36241330891889e-4;
t4391 = t17.*(t166+t205+t514+t533).*(-7.35522e-1);
t4393 = t9.*t323.*8.36241330891889e-4;
t4396 = t382.*2.74179553204116e-4;
t4413 = t353.*5.897280115119475e-3;
t4418 = t16.*t321.*4.67845486573025e-5;
t4437 = t410.*8.36241330891889e-4;
t4443 = t349.*2.454825983680473e-3;
t4446 = t354.*2.454825983680473e-3;
t4448 = t414.*2.74179553204116e-4;
t4452 = t409.*5.187945860934245e-5;
t4460 = t413.*4.67845486573025e-5;
t4482 = t2461+t2468;
t4487 = t321.*t4130;
t4497 = -t4472;
t4506 = t5.*t4436;
t4507 = t13.*t4436;
t4513 = -t4496;
t4516 = (t6.*t4374)./4.0;
t4517 = t241+t498+t1156+t1222;
t4518 = t413.*2.454825983680473e-3;
t4537 = t30.*t4436;
t4541 = t34.*t4436;
t4542 = t35.*t4436;
t4544 = t42.*t4436;
t4549 = -t4521;
t4556 = (t13.*t14.*t4374)./4.0;
t4557 = t314+t4251;
t4559 = -t4538;
t4562 = -t4548;
t4563 = -t4550;
t4578 = t55.*t4436;
t4581 = t68.*t4436;
t4582 = t71.*t4436;
t4583 = t4.*t4546;
t4586 = t47.*t4436;
t4588 = t4.*t4547;
t4596 = -t4561;
t4603 = -t4568;
t4606 = -t4570;
t4609 = t3915.*(-1.666555);
t4621 = -t4594;
t4622 = -t4595;
t4625 = t4.*t4567;
t4627 = -t4598;
t4638 = -t4600;
t4645 = -t4607;
t4647 = -t4610;
t4649 = -t4614;
t4651 = t109.*t4436;
t4655 = t116.*t4436;
t4657 = -t4617;
t4663 = t8.*(t69-t347).*(-5.187945860934245e-5);
t4667 = -t4628;
t4671 = -t4634;
t4673 = -t4636;
t4674 = -t4637;
t4683 = -t4646;
t4685 = t16.*(t69-t347).*(-4.67845486573025e-5);
t4694 = -t4661;
t4698 = t8.*(t69-t347).*5.187945860934245e-5;
t4705 = -t4670;
t4707 = -t4677;
t4710 = -t4678;
t4712 = -t4679;
t4715 = t16.*(t69-t347).*4.67845486573025e-5;
t4718 = -t4691;
t4734 = -t4708;
t4735 = -t4709;
t4739 = -t4716;
t4745 = -t4723;
t4750 = -t4733;
t4755 = -t4738;
t4759 = t16.*(t69-t347).*(-2.454825983680473e-3);
t4760 = t16.*t2501.*4.38178973375e-3;
t4761 = (t14.*t15.*t4531)./4.0;
t4772 = t168+t209+t452+t1010+t1393;
t4774 = t530+t1958+t2077;
t4775 = (t9.*t16.*t4551)./4.0;
t4776 = -t4751;
t4778 = -t4753;
t4784 = -t4756;
t4786 = t4130.*(t69-t347);
t4789 = t6.*t2561.*2.46255173325e-2;
t4792 = -t4765;
t4801 = -t4777;
t4805 = t17.*(t113-t409).*(-2.74179553204116e-4);
t4810 = -t4791;
t4812 = -t4793;
t4815 = (t7.*t14.*t4587)./4.0;
t4816 = (t223.*t4374)./2.0;
t4818 = -t4799;
t4820 = -t4800;
t4827 = -t4809;
t4828 = -t4811;
t4833 = -t4819;
t4839 = (t321.*t4383)./4.0;
t4844 = -t4830;
t4847 = t223.*t4548;
t4850 = -t4842;
t4851 = (t16.*t17.*t4701)./4.0;
t4864 = (t325.*t4432)./4.0;
t4865 = -t4852;
t4866 = -t4855;
t4867 = t223.*t4568;
t4868 = -t4856;
t4869 = (t321.*t4471)./4.0;
t4870 = -t4857;
t4872 = t323.*t4533;
t4875 = -t4861;
t4876 = -t4862;
t4877 = -t4863;
t4878 = (t323.*t4476)./4.0;
t4882 = t223.*t4607;
t4885 = t9.*t323.*t4410.*(-1.0./4.0);
t4886 = (t319.*t4473)./4.0;
t4887 = -t4874;
t4890 = (t403.*t4415)./2.0;
t4895 = (t321.*t4510)./4.0;
t4897 = (t319.*t4512)./4.0;
t4898 = (t320.*t4512)./4.0;
t4907 = -t4892;
t4912 = -t4899;
t4914 = (t325.*t4515)./4.0;
t4915 = (t321.*t4531)./2.0;
t4919 = (t323.*t4532)./4.0;
t4923 = (t225.*t4587)./2.0;
t4925 = (t325.*t4551)./2.0;
t4926 = (t323.*t4527)./4.0;
t4937 = (t403.*t4495)./4.0;
t4941 = t323.*t4689;
t4942 = (t404.*t4477)./4.0;
t4944 = t321.*t4723;
t4949 = t321.*t4716;
t4951 = t17.*t323.*t4515.*(-1.0./4.0);
t4953 = t16.*t321.*t4534.*(-1.0./4.0);
t4954 = (t321.*t4619)./4.0;
t4955 = -t4946;
t4957 = (t319.*t4624)./2.0;
t4958 = (t229.*t4701)./2.0;
t4960 = t8.*t321.*t4527.*(-1.0./4.0);
t4961 = (t323.*t4635)./4.0;
t4978 = t4410.*(t79-t358).*(-1.0./4.0);
t4979 = t14.*t3275.*2.46255173325e-2;
t4987 = (t4410.*(t79-t358))./4.0;
t4993 = (t323.*t4711)./2.0;
t4998 = t4471.*(t69-t347).*(-1.0./4.0);
t5018 = (t4471.*(t69-t347))./4.0;
t5025 = t4477.*(t48-t349).*(-1.0./4.0);
t5039 = t4499.*(t79-t358).*(-1.0./4.0);
t5054 = t17.*(t166+t205+t514+t533).*(-1.563719772e-3);
t5059 = (t4499.*(t79-t358))./4.0;
t5064 = t187+t492+t509+t1262+t1626;
t5065 = -t5026;
t5068 = t17.*(t166+t205+t514+t533).*1.563719772e-3;
t5072 = t4526.*(t48-t349).*(-1.0./4.0);
t5082 = t4534.*(t48-t349).*(-1.0./4.0);
t5092 = (t4526.*(t48-t349))./4.0;
t5095 = t214+t507+t537+t1054+t1624;
t5118 = t306+t398+t924+t1173+t1489;
t5139 = t300+t376+t1133+t1149+t1678;
t5145 = t4515.*(t106-t414).*(-1.0./4.0);
t5146 = t4701.*(t79-t358).*(-1.0./4.0);
t5154 = t4664.*(-1.225946);
t5158 = t4656.*(-3.228604);
t5161 = t4.*t5125;
t5163 = t594+t658+t1138+t1709;
t5164 = t4656.*(-3.587895);
t5167 = t4.*t5107;
t5170 = t4664.*(-3.587895);
t5173 = t4527.*(t113-t409).*(-1.0./4.0);
t5174 = t4726.*(t48-t349).*(-1.0./4.0);
t5175 = (t4701.*(t79-t358))./4.0;
t5179 = t4664.*1.225946;
t5182 = t4656.*3.228604;
t5185 = t4656.*3.587895;
t5187 = t4664.*3.587895;
t5188 = t4721.*(-1.666555);
t5189 = (t4726.*(t48-t349))./4.0;
t5191 = t4721.*(-1.225946);
t5195 = t4720.*(-3.587895);
t5200 = t3915.*(-1.17633784675e-2);
t5201 = t4721.*1.666555;
t5210 = t4721.*1.225946;
t5213 = t154+t253+t281+t842+t1086+t1383;
t5217 = t137+t240+t261+t1043+t1155+t1370;
t5219 = t4720.*3.587895;
t5221 = t3915.*1.17633784675e-2;
t5229 = t4.*t4436.*9.28985736e-3;
t5231 = -t5212;
t5233 = t665+t933+t1127+t1672;
t5254 = t737+t1162+t1249+t1525;
t5259 = -t5247;
t5270 = t926+t993+t1381+t1473;
t5282 = t6.*t5248;
t5283 = t4664.*(-1.8732399795e-1);
t5285 = t14.*t5248;
t5291 = t1019+t1110+t1506+t1619;
t5292 = t4664.*1.8732399795e-1;
t5297 = t4720.*(-1.8732399795e-1);
t5304 = -t5295;
t5307 = t975+t1352+t1610+t1690;
t5308 = t4720.*1.8732399795e-1;
t5309 = t1171+t1205+t1727+t1735;
t5326 = (t14.*t5274)./4.0;
t5355 = (t6.*t13.*t5274)./4.0;
t5370 = (t8.*t5314)./4.0;
t5382 = (t8.*t5312)./4.0;
t5392 = t7.*t5351;
t5393 = t15.*t5351;
t5398 = (t15.*t16.*t5314)./4.0;
t5399 = (t16.*t5334)./4.0;
t5405 = (t15.*t16.*t5312)./2.0;
t5412 = t14.*t4251.*2.46255173325e-2;
t5416 = t15.*t4255.*1.059103943995e-1;
t5421 = (t8.*t15.*t5334)./4.0;
t5432 = t7.*t4286.*1.059103943995e-1;
t5438 = -t5422;
t5453 = t5026.*3.587895;
t5459 = -t5445;
t5460 = -t5446;
t5461 = t5024.*3.228604;
t5462 = t5026.*3.228604;
t5467 = -t5454;
t5476 = -t5457;
t5478 = t3733+t3816;
t5494 = t1201+t1822+t1882+t2022;
t5498 = (t319.*t5274)./2.0;
t5499 = (t1748-t1821).*(t85+t338+t362+t375+t408+t5.*t12.*(7.9e+1./2.5e+2)).*(-1.0./4.0);
t5507 = ((t1748-t1821).*(t85+t338+t362+t375+t408+t5.*t12.*(7.9e+1./2.5e+2)))./4.0;
t5508 = t961+t1713+t1944+t2034;
t5509 = t3750+t3837;
t5517 = t837+t1380+t2036+t2116;
t5521 = (t3833.*(t85+t338+t362+t375+t408+t5.*t12.*(7.9e+1./2.5e+2)))./4.0;
t5524 = t90+t167+t1098+t1158+t1414+t1682;
t5533 = t12.*t4436.*1.015997283e-3;
t5537 = (t323.*t5312)./4.0;
t5539 = (t227.*t5334)./2.0;
t5540 = (t323.*t5314)./2.0;
t5543 = t434+t900+t1118+t1273+t1658;
t5575 = t4656.*(-6.3364582104e-2);
t5577 = t18.*t4436.*1.130503185e-3;
t5579 = t24.*t4436.*1.130503185e-3;
t5597 = t4656.*6.3364582104e-2;
t5611 = -t5591;
t5613 = t186+t489+t511+t1126+t1261+t1627;
t5616 = -t5594;
t5630 = t4721.*(-7.326866269e-3);
t5648 = t205+t514+t533+t1042+t1072+t1630;
t5652 = t4721.*7.326866269e-3;
t5653 = t6.*t4569.*2.46255173325e-2;
t5663 = -t5650;
t5669 = t14.*t4604.*2.46255173325e-2;
t5696 = t82+t124+t152+t1088+t1136+t1547+t1655;
t5713 = t86+t179+t212+t942+t1063+t1307+t1656;
t5716 = t94+t192+t213+t952+t1075+t1420+t1471;
t5722 = (t2701.*t4681)./4.0;
t5734 = t5334.*(t48-t349).*(-1.0./4.0);
t5745 = (t5334.*(t48-t349))./4.0;
t5779 = (t7.*t5723)./4.0;
t5780 = (t15.*t5709)./4.0;
t5783 = t868+t1027+t1131+t1403+t1538;
t5784 = -t5778;
t5790 = (t2701.*t4843)./4.0;
t5794 = (t7.*t14.*t5709)./4.0;
t5806 = t304+t546+t549+t1328+t1409+t1831;
t5807 = t878+t1150+t1231+t1240+t1677;
t5809 = t6.*t15.*t5709.*(-1.0./4.0);
t5810 = t752+t1145+t1264+t1644+t1674;
t5818 = (t14.*t43.*t5709)./2.0;
t5821 = t862+t1168+t1280+t1483+t1757;
t5829 = t779+t916+t1553+t1613+t1784;
t5835 = (t9.*t5763)./4.0;
t5836 = (t17.*t5761)./4.0;
t5839 = (t7.*t5777)./4.0;
t5840 = (t15.*t5776)./4.0;
t5843 = t1746+t1854+t1892+t3037;
t5860 = t296+t551+t564+t1629+t1661+t1834;
t5862 = (t16.*t17.*t5763)./4.0;
t5866 = t803+t1180+t1548+t1601+t1783;
t5868 = (t14.*t15.*t5777)./4.0;
t5872 = (t5.*t5785)./2.0;
t5873 = (t13.*t5787)./4.0;
t5874 = t8.*t9.*t5763.*(-1.0./4.0);
t5875 = t810+t1343+t1578+t1594+t1849;
t5877 = t989+t1079+t1549+t1639+t1782;
t5879 = t1064+t1227+t1412+t1519+t1862;
t5884 = t157+t286+t333+t1319+t1419+t1663+t1846;
t5885 = (t16.*t41.*t5763)./2.0;
t5887 = t6.*t7.*t5777.*(-1.0./4.0);
t5888 = t1114+t1301+t1486+t1712+t1775;
t5894 = t1034+t1387+t1602+t1692+t1800;
t5895 = (t4.*t13.*t5787)./2.0;
t5896 = (t5.*t12.*t5787)./2.0;
t5897 = (t12.*t13.*t5785)./2.0;
t5901 = (t14.*t37.*t5777)./2.0;
t5903 = (t17.*t5837)./4.0;
t5913 = t5026.*4.4422362436e-2;
t5918 = t5024.*6.3364582104e-2;
t5920 = (t9.*t5834)./4.0;
t5921 = (t14.*t5833)./4.0;
t5939 = (t225.*t5709)./2.0;
t5940 = (t226.*t5709)./2.0;
t5942 = (t15.*t5847)./4.0;
t5956 = (t5.*t14.*t5833)./2.0;
t5957 = (t6.*t13.*t5833)./2.0;
t5958 = (t13.*t14.*t5831)./2.0;
t5965 = (t9.*t16.*t5837)./4.0;
t5976 = (t6.*t15.*t5847)./2.0;
t5977 = (t7.*t14.*t5847)./2.0;
t5978 = (t14.*t15.*t5845)./2.0;
t5981 = t1045+t1531+t1636+t1844+t1851;
t5982 = (t321.*t5723)./2.0;
t5986 = t8.*t17.*t5837.*(-1.0./4.0);
t5988 = t1235+t1585+t1803+t1823+t1869;
t5990 = t1377+t1650+t1675+t1741+t1768;
t5997 = t15.*t223.*t5709.*(-1.0./4.0);
t5998 = (t13.*t42.*t5833)./4.0;
t6000 = (t16.*t45.*t5837)./2.0;
t6005 = t1365+t1401+t1806+t1815+t1860;
t6008 = (t229.*t5763)./2.0;
t6009 = (t230.*t5763)./2.0;
t6015 = (t14.*t43.*t5847)./4.0;
t6029 = t1342+t1721+t1796+t1816+t1884;
t6033 = (t225.*t5776)./2.0;
t6042 = (t325.*t5761)./2.0;
t6050 = (t403.*t5709)./4.0;
t6053 = -t6035;
t6054 = -t6036;
t6064 = t1425+t1616+t1753+t1781+t1908;
t6066 = (t321.*t5777)./2.0;
t6067 = (t322.*t5777)./2.0;
t6079 = t7.*t223.*t5777.*(-1.0./4.0);
t6088 = (t369.*t5777)./4.0;
t6098 = (t405.*t5763)./4.0;
t6099 = (t223.*t5831)./4.0;
t6101 = -t6090;
t6102 = -t6091;
t6103 = (t229.*t5834)./2.0;
t6105 = -t6093;
t6106 = -t6094;
t6119 = (t225.*t5847)./4.0;
t6123 = -t6107;
t6125 = -t6109;
t6135 = (t320.*t5833)./2.0;
t6136 = (t319.*t5833)./4.0;
t6139 = (t325.*t5837)./2.0;
t6140 = (t326.*t5837)./2.0;
t6152 = (t321.*t5845)./4.0;
t6154 = -t6133;
t6163 = (t4841.*(t85+t338+t362+t375+t408+t5.*t12.*(7.9e+1./2.5e+2)))./4.0;
t6170 = t15.*t223.*t5847.*(-1.0./4.0);
t6172 = (t371.*t5837)./4.0;
t6175 = t646+t2310+t2725+t2780;
t6178 = -t6160;
t6181 = t12.*t3243.*t4436.*8.07151e-1;
t6185 = (t583.*t5598)./4.0;
t6196 = t642+t2307+t2743+t2779;
t6199 = t12.*t3261.*t4436.*8.07151e-1;
t6203 = -t6187;
t6215 = (t403.*t5847)./2.0;
t6223 = t1752+t1787+t2799+t3025;
t6226 = t5763.*(t79-t358).*(-1.0./4.0);
t6230 = t5777.*(t69-t347).*(-1.0./2.0);
t6233 = t12.*t3316.*t4436.*8.07151e-1;
t6234 = t4.*t3318.*t4436.*8.07151e-1;
t6236 = t12.*t3318.*t4436.*8.07151e-1;
t6240 = (t5763.*(t79-t358))./4.0;
t6242 = (t5777.*(t69-t347))./2.0;
t6246 = (t4905.*(t85+t338+t362+t375+t408+t5.*t12.*(7.9e+1./2.5e+2)))./2.0;
t6249 = t12.*t4436.*(t881-t912).*8.07151e-1;
t6277 = (t4337.*t4436)./4.0;
t6278 = -t6261;
t6284 = (t3275.*t5115)./2.0;
t6292 = (t1572.*t5598)./4.0;
t6294 = (t4356.*t4436)./4.0;
t6296 = t5834.*(t79-t358).*(-1.0./4.0);
t6312 = (t5834.*(t79-t358))./4.0;
t6318 = t6.*t5740.*6.8635e-3;
t6350 = -t6333;
t6397 = t1592+t2403+t2902+t3017;
t6423 = t1053+t1211+t3327+t3449;
t6437 = t12.*t13.*(t2425-t2468).*(t85+t338+t362+t375+t408+t5.*t12.*(7.9e+1./2.5e+2)).*(-8.9697375e-1);
t6444 = t12.*t13.*(t2425-t2468).*(t85+t338+t362+t375+t408+t5.*t12.*(7.9e+1./2.5e+2)).*8.9697375e-1;
t6484 = t4584+t4653;
t6506 = (t4152.*(t2904-t2927))./4.0;
t6508 = t4590+t4720;
t6512 = (t4265.*(t2821-t2864))./4.0;
t6531 = -t6520;
t6538 = -t7.*(t4650+t34.*(t2425-t2468));
t6539 = -t15.*(t4650+t34.*(t2425-t2468));
t6542 = -t6530;
t6551 = t16.*t6046.*2.62925e-3;
t6554 = -t6545;
t6560 = (t12.*t4436.*t4860)./4.0;
t6569 = (t12.*t4436.*t4873)./4.0;
t6591 = (t12.*t4436.*t4906)./4.0;
t6592 = (t4.*t4436.*t4908)./4.0;
t6593 = (t12.*t4436.*t4908)./4.0;
t6602 = t12.*t4436.*(t2798-t2848).*(-1.0./4.0);
t6613 = (t12.*t4436.*(t2798-t2848))./4.0;
t6626 = (t2561.*t5750)./2.0;
t6627 = (t2568.*t5740)./2.0;
t6651 = t14.*t6222.*6.8635e-3;
t6693 = t1356+t1399+t1874+t1896+t1921+t1941;
t6698 = -t6684;
t6699 = -t6685;
t6713 = t1140+t1405+t1909+t1910+t1922+t1946;
t6715 = -t6694;
t6716 = -t6695;
t6750 = t1895+t6222;
t6799 = (t3275.*t5739)./2.0;
t6800 = (t3254.*t5750)./2.0;
t6823 = (t3292.*t5740)./2.0;
t6860 = (t5598.*(t85+t338+t362+t375+t408+t5.*t12.*(7.9e+1./2.5e+2)))./2.0;
t6861 = (t5598.*(t85+t338+t362+t375+t408+t5.*t12.*(7.9e+1./2.5e+2)))./4.0;
t6879 = -t6839;
t6930 = (t2520.*t6046)./2.0;
t6941 = (t2501.*t6069)./2.0;
t6974 = -t6960;
t6981 = t15.*(t4650+t34.*(t2425-t2468)).*(-1.666555);
t6984 = t7.*(t4650+t34.*(t2425-t2468)).*(-1.225946);
t6985 = t15.*(t4650+t34.*(t2425-t2468)).*(-1.225946);
t6993 = (t3643.*t5740)./4.0;
t7108 = t5016+t5024;
t7131 = t18.*t4436.*t4959.*3.23463e-1;
t7137 = t24.*t4436.*t4959.*1.937765;
t7149 = -t7.*(t5026+t5.*(t2959-t2967));
t7151 = -t15.*(t5026+t5.*(t2959-t2967));
t7154 = (t4474.*t5434)./4.0;
t7191 = (t4884.*t5275)./4.0;
t7218 = -t7206;
t7228 = (t5277.*(t2821-t2864))./4.0;
t7252 = t6.*t7210;
t7254 = t14.*t7210;
t7256 = (t4251.*t5740)./4.0;
t7260 = -t7248;
t7261 = -t7249;
t7263 = (t5290.*(t2904-t2927))./4.0;
t7275 = t6.*t7237;
t7277 = t7.*t7237;
t7278 = t14.*t7237;
t7279 = t15.*t7237;
t7287 = (t3780.*t6046)./2.0;
t7288 = -t7274;
t7293 = t6.*t6762.*6.8635e-3;
t7294 = t5151+t5190;
t7296 = t5165+t5196;
t7302 = t14.*t6763.*6.8635e-3;
t7399 = t7.*t7344;
t7401 = t15.*t7344;
t7408 = t7.*(t4650+t34.*(t2425-t2468)).*(-2.5171736245e-2);
t7414 = t15.*(t4650+t34.*(t2425-t2468)).*(-7.326866269e-3);
t7415 = t6.*(t4650+t34.*(t2425-t2468)).*(-2.46255173325e-2);
t7417 = t7.*(t4650+t34.*(t2425-t2468)).*2.5171736245e-2;
t7418 = (t4436.*t5759)./4.0;
t7426 = t15.*(t4650+t34.*(t2425-t2468)).*7.326866269e-3;
t7427 = t6.*(t4650+t34.*(t2425-t2468)).*2.46255173325e-2;
t7429 = (t4436.*t5772)./4.0;
t7452 = (t4436.*t5795)./4.0;
t7484 = (t943-t1091).*(t985+t3399-t13.*t42.*1.01140545e-1-t7.*t223.*5.034347249e-2).*(-1.0./4.0);
t7496 = ((t943-t1091).*(t985+t3399-t13.*t42.*1.01140545e-1-t7.*t223.*5.034347249e-2))./4.0;
t7538 = t711+t1361+t1591+t2839+t2901+t3120;
t7540 = t699+t973+t1569+t2917+t2952+t3111;
t7542 = t7.*(t5026+t5.*(t2959-t2967)).*(-1.666555);
t7546 = t7.*(t5026+t5.*(t2959-t2967)).*(-1.225946);
t7547 = t15.*(t5026+t5.*(t2959-t2967)).*(-1.225946);
t7606 = (t5277.*t5331)./4.0;
t7632 = t4.*t4436.*t5530.*1.617315e-1;
t7637 = t12.*t4436.*t5535.*1.617315e-1;
t7680 = (t5290.*t5365)./4.0;
t7766 = (t5275.*t5443)./4.0;
t7903 = -t7887;
t7927 = (t4436.*t6338)./4.0;
t7980 = t717+t723+t2913+t2920+t3038+t3161;
t8019 = (t4860.*t6159)./4.0;
t8032 = t7.*(t5026+t5.*(t2959-t2967)).*(-7.326866269e-3);
t8034 = t15.*(t5026+t5.*(t2959-t2967)).*(-2.5171736245e-2);
t8036 = (t3249.*t6969)./4.0;
t8042 = t7.*(t5026+t5.*(t2959-t2967)).*7.326866269e-3;
t8045 = t15.*(t5026+t5.*(t2959-t2967)).*2.5171736245e-2;
t8061 = (t4908.*t6155)./4.0;
t8064 = (t4906.*t6159)./4.0;
t8069 = (t6928.*(t943-t1091))./4.0;
t8073 = t13.*(t5026+t5.*(t2959-t2967)).*(-2.01382560198e-1);
t8085 = t6159.*(t2798-t2848).*(-1.0./2.0);
t8086 = t6159.*(t2798-t2848).*(-1.0./4.0);
t8092 = t13.*(t5026+t5.*(t2959-t2967)).*2.01382560198e-1;
t8093 = (t3424.*t6928)./4.0;
t8104 = (t6159.*(t2798-t2848))./2.0;
t8105 = (t6159.*(t2798-t2848))./4.0;
t8118 = (t3421.*t6966)./4.0;
t8119 = -t8108;
t8120 = -t8109;
t8125 = (t4.*t4436.*t6481)./4.0;
t8130 = (t12.*t4436.*t6483)./4.0;
t8137 = (t3489.*t6966)./4.0;
t8146 = (t4936.*t6205)./4.0;
t8152 = (t4916.*t6216)./4.0;
t8205 = t3405+t5034+t5043;
t8206 = t12.*t4436.*t6155.*8.07151e-1;
t8210 = t4.*t4436.*t6159.*8.07151e-1;
t8211 = t12.*t4436.*t6159.*8.07151e-1;
t8242 = t12.*t6155.*(t2425-t2468).*(-8.07151e-1);
t8243 = t4.*t6159.*(t2425-t2468).*(-8.07151e-1);
t8244 = t12.*t6159.*(t2425-t2468).*(-8.07151e-1);
t8247 = (t3752.*t6969)./4.0;
t8258 = t12.*t6155.*(t2425-t2468).*8.07151e-1;
t8260 = t4.*t6159.*(t2425-t2468).*8.07151e-1;
t8262 = t12.*t6159.*(t2425-t2468).*8.07151e-1;
t8285 = t1226+t2546+t2591+t2996+t2999+t3115;
t8302 = (t5450.*t5759)./2.0;
t8310 = t986+t2595+t2600+t3092+t3124+t3141;
t8312 = -t8.*(t7.*(t4650+t34.*(t2425-t2468))+t47.*(t2425-t2468));
t8315 = -t16.*(t7.*(t4650+t34.*(t2425-t2468))+t47.*(t2425-t2468));
t8329 = -t9.*(t4654+t15.*(t4650+t34.*(t2425-t2468)));
t8331 = t16.*(t7.*(t4650+t34.*(t2425-t2468))+t47.*(t2425-t2468));
t8332 = -t17.*(t4654+t15.*(t4650+t34.*(t2425-t2468)));
t8337 = (t4436.*t6646)./4.0;
t8350 = t9.*(t4654+t15.*(t4650+t34.*(t2425-t2468)));
t8360 = t6646.*(t2425-t2468).*(-1.0./4.0);
t8370 = (t6646.*(t2425-t2468))./4.0;
t8435 = (t3243.*t7389)./4.0;
t8437 = t610+t834+t867+t2820+t2852+t2983+t3192;
t8438 = t612+t848+t877+t2826+t2859+t3052+t3134;
t8465 = (t3318.*t7386)./4.0;
t8466 = (t3316.*t7389)./4.0;
t8477 = t706+t710+t960+t2903+t2906+t3091+t3155;
t8479 = (t7389.*(t881-t912))./2.0;
t8480 = (t7389.*(t881-t912))./4.0;
t8486 = -t8470;
t8502 = t12.*t4959.*t6159.*1.614302;
t8522 = (t3405.*t7422)./4.0;
t8550 = t5.*t7620.*2.01382560198e-1;
t8577 = t13.*t7656.*2.01382560198e-1;
t8609 = t758+t1210+t1253+t2990+t3133+t3149+t3244;
t8620 = (t4959.*t6646)./2.0;
t8635 = t8.*(t7.*(t4650+t34.*(t2425-t2468))+t47.*(t2425-t2468)).*(-1.666555);
t8653 = t17.*(t4654+t15.*(t4650+t34.*(t2425-t2468))).*(-7.35522e-1);
t8706 = t4681.*(t5026+t5.*(t2959-t2967)).*(-1.0./4.0);
t8710 = (t4681.*(t5026+t5.*(t2959-t2967)))./4.0;
t8728 = t3113+t5436+t5484;
t8734 = t3122+t5422+t5501;
t8745 = t4843.*(t5026+t5.*(t2959-t2967)).*(-1.0./4.0);
t8754 = (t4843.*(t5026+t5.*(t2959-t2967)))./4.0;
t8768 = (t4436.*t7362)./4.0;
t8819 = (t12.*t4436.*t7386)./4.0;
t8823 = (t4.*t4436.*t7389)./4.0;
t8824 = (t12.*t4436.*t7389)./4.0;
t8855 = t12.*t7386.*(t2425-t2468).*(-1.0./4.0);
t8859 = t4.*t7389.*(t2425-t2468).*(-1.0./4.0);
t8860 = t12.*t7389.*(t2425-t2468).*(-1.0./4.0);
t8875 = (t12.*t7386.*(t2425-t2468))./4.0;
t8877 = (t4.*t7389.*(t2425-t2468))./4.0;
t8879 = (t12.*t7389.*(t2425-t2468))./4.0;
t8921 = t5.*t8156.*2.01382560198e-1;
t8934 = t12.*t13.*t8156.*2.01382560198e-1;
t8957 = t8.*(t7.*(t4650+t34.*(t2425-t2468))+t47.*(t2425-t2468)).*(-1.17633784675e-2);
t8964 = t7.*(t7.*(t4650+t34.*(t2425-t2468))+t47.*(t2425-t2468)).*(-1.059103943995e-1);
t8980 = t17.*(t4654+t15.*(t4650+t34.*(t2425-t2468))).*(-1.563719772e-3);
t8986 = t15.*(t4654+t15.*(t4650+t34.*(t2425-t2468))).*(-1.059103943995e-1);
t9035 = (t12.*t4959.*t7389)./2.0;
t9116 = (t4843.*t7734)./4.0;
t9126 = (t4936.*t7620)./4.0;
t9139 = (t4916.*t7656)./4.0;
t9155 = t7.*(t7.*(t4650+t34.*(t2425-t2468)).*1.225946+t47.*(t2425-t2468).*1.225946).*(-8.639075e-2);
t9215 = t4905+t5424+t5502;
t9218 = t4916+t5436+t5484;
t9426 = (t4930.*t8156)./4.0;
t9491 = t4884.*(t4654+t15.*(t4650+t34.*(t2425-t2468))).*(-1.0./4.0);
t9495 = (t4884.*(t4654+t15.*(t4650+t34.*(t2425-t2468))))./4.0;
t9522 = t12.*t13.*t8156.*(t2425-t2468).*(-8.07151e-1);
t9528 = t12.*t13.*t8156.*(t2425-t2468).*8.07151e-1;
t9550 = -t9540;
t9638 = (t6155.*t7389)./2.0;
t9639 = (t6159.*t7386)./2.0;
t9687 = t4255.*(t7.*(t4650+t34.*(t2425-t2468)).*1.225946+t47.*(t2425-t2468).*1.225946).*(-1.0./4.0);
t9690 = (t4255.*(t7.*(t4650+t34.*(t2425-t2468)).*1.225946+t47.*(t2425-t2468).*1.225946))./4.0;
t9763 = t5443.*(t4654+t15.*(t4650+t34.*(t2425-t2468))).*(-1.0./4.0);
t10271 = -t9.*(t16.*(t30.*(t2425-t2468)+t68.*(t2425-t2468))+t8.*(t7.*(t4650+t34.*(t2425-t2468))+t47.*(t2425-t2468)));
t10272 = -t17.*(t16.*(t30.*(t2425-t2468)+t68.*(t2425-t2468))+t8.*(t7.*(t4650+t34.*(t2425-t2468))+t47.*(t2425-t2468)));
t10488 = t9.*(t16.*(t30.*(t2425-t2468)+t68.*(t2425-t2468))+t8.*(t7.*(t4650+t34.*(t2425-t2468))+t47.*(t2425-t2468))).*(-7.35522e-1);
t10489 = t17.*(t16.*(t30.*(t2425-t2468)+t68.*(t2425-t2468))+t8.*(t7.*(t4650+t34.*(t2425-t2468))+t47.*(t2425-t2468))).*(-7.35522e-1);
t10692 = t8156.*(-t2715+t3105+t5080.*3.228604).*(-1.0./2.0);
t10710 = t7422.*(-t3405+t4994+t5076).*(-1.0./2.0);
t10735 = t17.*(t16.*(t30.*(t2425-t2468)+t68.*(t2425-t2468))+t8.*(t7.*(t4650+t34.*(t2425-t2468))+t47.*(t2425-t2468))).*(-3.867742437e-3);
t10741 = t8.*(t16.*(t30.*(t2425-t2468)+t68.*(t2425-t2468))+t8.*(t7.*(t4650+t34.*(t2425-t2468))+t47.*(t2425-t2468))).*(-4.38178973375e-3);
t10742 = t9.*(t16.*(t30.*(t2425-t2468)+t68.*(t2425-t2468))+t8.*(t7.*(t4650+t34.*(t2425-t2468))+t47.*(t2425-t2468))).*(-1.563719772e-3);
t10743 = t17.*(t16.*(t30.*(t2425-t2468)+t68.*(t2425-t2468))+t8.*(t7.*(t4650+t34.*(t2425-t2468))+t47.*(t2425-t2468))).*3.867742437e-3;
t10746 = t8.*(t16.*(t30.*(t2425-t2468)+t68.*(t2425-t2468))+t8.*(t7.*(t4650+t34.*(t2425-t2468))+t47.*(t2425-t2468))).*4.38178973375e-3;
t10866 = t8.*(t16.*(t30.*(t2425-t2468)+t68.*(t2425-t2468)).*1.666555+t8.*(t7.*(t4650+t34.*(t2425-t2468))+t47.*(t2425-t2468)).*1.666555).*(-2.62925e-3);
t10869 = t8.*(t16.*(t30.*(t2425-t2468)+t68.*(t2425-t2468)).*1.666555+t8.*(t7.*(t4650+t34.*(t2425-t2468))+t47.*(t2425-t2468)).*1.666555).*2.62925e-3;
t11312 = -q6d.*(t3355-t3398-t3536+t6133+t6524+(t17.*(t689-t740))./2.0);
t11602 = t6046.*(t16.*(t30.*(t2425-t2468)+t68.*(t2425-t2468))+t8.*(t7.*(t4650+t34.*(t2425-t2468))+t47.*(t2425-t2468))).*(-1.0./4.0);
t12567 = t9.*(t9.*(t16.*(t30.*(t2425-t2468)+t68.*(t2425-t2468))+t8.*(t7.*(t4650+t34.*(t2425-t2468))+t47.*(t2425-t2468)))+t17.*(t4654+t15.*(t4650+t34.*(t2425-t2468)))).*(-1.13264871585e-2);
t12682 = t9.*(t9.*(t16.*(t30.*(t2425-t2468)+t68.*(t2425-t2468))+t8.*(t7.*(t4650+t34.*(t2425-t2468))+t47.*(t2425-t2468))).*7.35522e-1+t17.*(t4654+t15.*(t4650+t34.*(t2425-t2468))).*7.35522e-1).*(-1.539925e-2);
t12906 = t3738.*(t9.*(t16.*(t30.*(t2425-t2468)+t68.*(t2425-t2468))+t8.*(t7.*(t4650+t34.*(t2425-t2468))+t47.*(t2425-t2468))).*7.35522e-1+t17.*(t4654+t15.*(t4650+t34.*(t2425-t2468))).*7.35522e-1).*(-1.0./4.0);
t12910 = (t3738.*(t9.*(t16.*(t30.*(t2425-t2468)+t68.*(t2425-t2468))+t8.*(t7.*(t4650+t34.*(t2425-t2468))+t47.*(t2425-t2468))).*7.35522e-1+t17.*(t4654+t15.*(t4650+t34.*(t2425-t2468))).*7.35522e-1))./4.0;
t13015 = t5434.*(t9.*(t16.*(t30.*(t2425-t2468)+t68.*(t2425-t2468))+t8.*(t7.*(t4650+t34.*(t2425-t2468))+t47.*(t2425-t2468)))+t17.*(t4654+t15.*(t4650+t34.*(t2425-t2468)))).*(-1.0./4.0);
t13017 = (t5434.*(t9.*(t16.*(t30.*(t2425-t2468)+t68.*(t2425-t2468))+t8.*(t7.*(t4650+t34.*(t2425-t2468))+t47.*(t2425-t2468)))+t17.*(t4654+t15.*(t4650+t34.*(t2425-t2468)))))./4.0;
t411 = -t380;
t412 = t8.*t389;
t415 = t8.*t395;
t417 = -t386;
t418 = -t395;
t436 = -t426;
t447 = t385.*(1.1e+1./1.25e+2);
t448 = t386.*(1.1e+1./1.25e+2);
t451 = t394.*(1.1e+1./1.25e+2);
t470 = t47+t384;
t483 = t73+t388;
t484 = t64+t397;
t485 = t9.*t454;
t486 = t17.*t454;
t497 = t8.*t456;
t500 = t116+t391;
t516 = t110+t394;
t517 = t119+t390;
t531 = t9.*t473;
t532 = t17.*t473;
t542 = -t9.*(t71-t391);
t543 = -t17.*(t71-t391);
t562 = t9.*t538;
t563 = t17.*t538;
t578 = t8.*t9.*(t71-t391);
t586 = t251+t431;
t598 = t16.*t574;
t599 = t17.*t574;
t600 = t265+t427;
t604 = t381+t385;
t614 = t8.*t571;
t615 = t9.*t571;
t616 = t16.*t571;
t617 = t17.*t571;
t622 = t8.*t574;
t623 = t9.*t574;
t702 = t9.*t16.*(t71-t391).*(-1.1e+1./1.25e+2);
t713 = t16.*t17.*(t71-t391).*(-1.1e+1./1.25e+2);
t800 = -t624;
t824 = t163.*(t71-t391);
t831 = -t9.*(t208-t427);
t845 = -t17.*(t208-t427);
t1302 = -t9.*(t380-t392);
t1309 = t328+t474;
t1316 = -t17.*(t380-t392);
t1778 = -t1475;
t1804 = -t1510;
t1904 = t393+t518;
t1907 = t389+t527;
t1914 = t384.*2.9474e-2;
t1919 = t391.*2.9474e-2;
t1938 = -t1916;
t1939 = -t1917;
t1951 = -t1932;
t1962 = t389.*1.2516e-2;
t1964 = t390.*1.2516e-2;
t1966 = t395.*1.2516e-2;
t1981 = t384.*3.8437e-2;
t1984 = t391.*3.8437e-2;
t2003 = -t1959;
t2007 = -t1960;
t2053 = t381.*4.815e-3;
t2056 = -t1976;
t2058 = -t1980;
t2059 = t385.*4.815e-3;
t2060 = t386.*4.815e-3;
t2061 = t384.*3.5549e-2;
t2063 = t394.*4.815e-3;
t2064 = t391.*3.5549e-2;
t2065 = t381.*6.0149e-2;
t2070 = -t1982;
t2071 = -t1983;
t2073 = t384.*6.0149e-2;
t2074 = t385.*6.0149e-2;
t2075 = t386.*6.0149e-2;
t2076 = -t1987;
t2078 = t391.*6.0149e-2;
t2080 = t394.*6.0149e-2;
t2083 = -t1997;
t2084 = -t1998;
t2085 = t384.*4.1065e-2;
t2086 = -t2004;
t2088 = t391.*4.1065e-2;
t2089 = -t2014;
t2090 = -t2015;
t2091 = -t2017;
t2092 = -t2018;
t2097 = -t2026;
t2098 = t381.*4.354e-3;
t2099 = -t2033;
t2104 = t385.*4.354e-3;
t2105 = t386.*4.354e-3;
t2107 = t7.*t1936;
t2108 = t7.*t1937;
t2110 = t394.*4.354e-3;
t2114 = t15.*t1936;
t2115 = t15.*t1937;
t2118 = -t2046;
t2120 = -t2050;
t2121 = t389.*6.1597e-2;
t2123 = t390.*6.1597e-2;
t2124 = t384.*5.433e-3;
t2125 = t395.*6.1597e-2;
t2127 = t397.*6.1597e-2;
t2128 = t391.*5.433e-3;
t2137 = -t2068;
t2138 = t381.*4.252e-3;
t2140 = t388.*1.964e-3;
t2141 = t380.*1.4117e-2;
t2142 = t384.*1.1953e-2;
t2145 = t392.*1.964e-3;
t2146 = t393.*1.964e-3;
t2147 = t385.*4.252e-3;
t2148 = t386.*4.252e-3;
t2149 = t389.*4.252e-3;
t2151 = t390.*4.252e-3;
t2152 = t391.*1.1953e-2;
t2155 = t394.*4.252e-3;
t2156 = t395.*4.252e-3;
t2158 = t384.*1.4117e-2;
t2160 = t388.*1.4117e-2;
t2161 = t380.*1.0517e-2;
t2163 = t381.*1.196e-3;
t2165 = t391.*1.4117e-2;
t2166 = t392.*1.4117e-2;
t2167 = t393.*1.4117e-2;
t2168 = t381.*1.0517e-2;
t2172 = t389.*4.28e-4;
t2174 = t390.*4.28e-4;
t2180 = t385.*1.196e-3;
t2181 = t386.*1.196e-3;
t2182 = t389.*1.196e-3;
t2184 = t390.*1.196e-3;
t2185 = t395.*4.28e-4;
t2187 = t397.*4.28e-4;
t2188 = t385.*1.0517e-2;
t2189 = t386.*1.0517e-2;
t2191 = t388.*1.0517e-2;
t2192 = t389.*1.0517e-2;
t2194 = -t2094;
t2195 = -t2095;
t2196 = t384.*2.117e-3;
t2197 = t380.*1.158e-3;
t2199 = t394.*1.196e-3;
t2200 = t395.*1.196e-3;
t2201 = t392.*1.0517e-2;
t2202 = t393.*1.0517e-2;
t2204 = t394.*1.0517e-2;
t2205 = t395.*1.0517e-2;
t2207 = t397.*1.0517e-2;
t2209 = t391.*2.117e-3;
t2210 = t384.*4.037e-3;
t2211 = t384.*6.4725936e-2;
t2212 = t391.*4.037e-3;
t2213 = t391.*6.4725936e-2;
t2214 = t384.*1.158e-3;
t2216 = t388.*1.158e-3;
t2220 = t391.*1.158e-3;
t2221 = t392.*1.158e-3;
t2222 = t393.*1.158e-3;
t2223 = -t2119;
t2225 = t389.*1.0027e-2;
t2227 = -t2122;
t2230 = t395.*1.0027e-2;
t2232 = t397.*1.0027e-2;
t2233 = -t2126;
t2235 = t380.*1.964e-3;
t2237 = -t2132;
t2238 = -t2133;
t2240 = t394.*7.41e-4;
t2241 = t395.*7.41e-4;
t2243 = t397.*7.41e-4;
t2251 = t424.*1.2516e-2;
t2257 = t381.*3.41e-4;
t2258 = -t2170;
t2259 = -t2171;
t2263 = -t2177;
t2270 = t384.*3.41e-4;
t2271 = t385.*3.41e-4;
t2272 = t386.*3.41e-4;
t2279 = t391.*3.41e-4;
t2281 = t394.*3.41e-4;
t2287 = -t2106;
t2291 = t384.*2.29e-4;
t2294 = -t2217;
t2300 = t391.*2.29e-4;
t2308 = t381.*7.41e-4;
t2313 = t385.*7.41e-4;
t2314 = t386.*7.41e-4;
t2315 = t389.*7.41e-4;
t2323 = t380.*1.09e-4;
t2328 = t381.*1.09e-4;
t2338 = t385.*1.09e-4;
t2339 = t386.*1.09e-4;
t2341 = t388.*1.09e-4;
t2342 = t392.*1.09e-4;
t2343 = t393.*1.09e-4;
t2345 = t394.*1.09e-4;
t2347 = t16.*t389.*6.4725936e-2;
t2349 = t16.*t395.*6.4725936e-2;
t2353 = -t2290;
t2363 = -t2309;
t2367 = t488+t513;
t2370 = -t2319;
t2372 = t9.*t2236;
t2373 = -t2327;
t2374 = t17.*t2236;
t2376 = -t2331;
t2377 = -t2336;
t2386 = t423.*6.1597e-2;
t2387 = t424.*6.1597e-2;
t2388 = -t2360;
t2391 = -t2362;
t2394 = -t2364;
t2395 = t424.*4.252e-3;
t2398 = t423.*4.28e-4;
t2400 = t424.*4.28e-4;
t2401 = t423.*1.0517e-2;
t2404 = t424.*1.196e-3;
t2408 = -t2379;
t2409 = t469.*7.35522e-1;
t2412 = t465.*1.666555;
t2414 = t423.*1.0027e-2;
t2416 = t469.*1.666555;
t2418 = t423+t585;
t2421 = -t2390;
t2426 = -t2397;
t2427 = -t8.*(t479+t534);
t2430 = -t16.*(t479+t534);
t2437 = -t2417;
t2440 = -t2419;
t2442 = t423.*7.41e-4;
t2445 = t439.*t587;
t2458 = t424+t618;
t2462 = t505.*7.35522e-1;
t2463 = t506.*7.35522e-1;
t2465 = -t2446;
t2467 = t16.*(t479+t534);
t2479 = -t2453;
t2488 = t503.*7.35522e-1;
t2489 = t504.*7.35522e-1;
t2496 = t9.*t439.*6.1597e-2;
t2498 = t17.*t439.*6.1597e-2;
t2499 = -t2476;
t2508 = t439.*t687;
t2509 = t439.*t689;
t2511 = t439.*t701;
t2515 = t439.*t751;
t2525 = t439.*t775;
t2529 = t439.*t798;
t2530 = t9.*(t71-t391).*(-1.2516e-2);
t2531 = t17.*(t71-t391).*(-1.2516e-2);
t2532 = t17.*t439.*(-1.0517e-2);
t2556 = t439.*t906;
t2586 = -t2536;
t2607 = t16.*(t71-t391).*(-4.815e-3);
t2610 = t17.*t439.*(-7.41e-4);
t2642 = t16.*(t71-t391).*(-4.354e-3);
t2647 = t9.*(t71-t391).*(-6.1597e-2);
t2650 = t17.*(t71-t391).*(-6.1597e-2);
t2664 = t16.*(t71-t391).*(-6.0149e-2);
t2669 = t9.*(t71-t391).*(-1.196e-3);
t2670 = t17.*(t71-t391).*(-4.28e-4);
t2671 = t8.*(t71-t391).*(-1.0517e-2);
t2672 = t9.*(t71-t391).*(-1.0517e-2);
t2673 = t16.*(t71-t391).*(-1.196e-3);
t2674 = t17.*(t71-t391).*(-1.196e-3);
t2675 = t16.*(t71-t391).*(-1.0517e-2);
t2676 = t17.*(t71-t391).*(-1.0517e-2);
t2677 = t8.*(t71-t391).*(-1.158e-3);
t2678 = t9.*(t71-t391).*(-1.0027e-2);
t2679 = t17.*(t71-t391).*(-1.0027e-2);
t2680 = t17.*(t71-t391).*6.1597e-2;
t2681 = t8.*(t71-t391).*(-1.964e-3);
t2682 = t9.*(t71-t391).*(-4.252e-3);
t2684 = t660.*(t71-t391);
t2685 = t16.*(t71-t391).*(-4.252e-3);
t2686 = t17.*(t71-t391).*(-4.252e-3);
t2687 = t8.*(t71-t391).*(-1.4117e-2);
t2691 = t9.*(t71-t391).*(-4.28e-4);
t2693 = t687.*(t71-t391);
t2694 = t692.*(t71-t391);
t2695 = t695.*(t71-t391);
t2696 = t700.*(t71-t391);
t2697 = t16.*(t71-t391).*(-3.41e-4);
t2700 = t740.*(t71-t391);
t2702 = t9.*(t71-t391).*(-7.41e-4);
t2703 = t16.*(t71-t391).*(-7.41e-4);
t2704 = t17.*(t71-t391).*(-7.41e-4);
t2705 = t618.*(-1.2516e-2);
t2706 = t775.*(t71-t391);
t2707 = t783.*(t71-t391);
t2709 = t798.*(t71-t391);
t2710 = t16.*(t71-t391).*(-1.09e-4);
t2711 = t9.*t16.*(t71-t391).*(-6.4725936e-2);
t2714 = t16.*t17.*(t71-t391).*(-6.4725936e-2);
t2719 = t843.*(t71-t391);
t2736 = t1347.*(t71-t391);
t2737 = t8.*(t71-t391).*(-1.09e-4);
t2738 = t957.*(t71-t391);
t2739 = t618.*(-6.1597e-2);
t2740 = t982.*(t71-t391);
t2749 = t620.*7.35522e-1;
t2752 = t624.*7.35522e-1;
t2759 = t620.*1.666555;
t2764 = t624.*1.666555;
t2786 = t1161.*(t71-t391);
t2789 = t618.*6.1597e-2;
t2809 = t618.*(-4.252e-3);
t2830 = t618.*(-4.28e-4);
t2831 = t618.*(-1.196e-3);
t2894 = t618.*4.252e-3;
t2932 = t618.*1.196e-3;
t2966 = t571+t765;
t2980 = t574+t766;
t2986 = -t2885;
t2987 = -t2886;
t3002 = t9.*(t208-t427).*(-7.35522e-1);
t3005 = t17.*(t208-t427).*(-7.35522e-1);
t3166 = t9.*(t380-t392).*(-1.2516e-2);
t3195 = t1510.*7.35522e-1;
t3199 = t1462.*1.666555;
t3201 = t1540.*7.35522e-1;
t3205 = t1475.*1.666555;
t3213 = t1510.*1.666555;
t3218 = t1540.*1.666555;
t3228 = t1462.*7.35522e-1;
t3242 = t9.*(t380-t392).*(-6.1597e-2);
t3245 = t17.*(t380-t392).*(-6.1597e-2);
t3250 = t9.*(t380-t392).*(-4.252e-3);
t3255 = t9.*(t380-t392).*(-4.28e-4);
t3257 = t9.*(t380-t392).*(-1.196e-3);
t3258 = t17.*(t380-t392).*(-4.28e-4);
t3259 = t17.*(t380-t392).*(-1.0517e-2);
t3262 = t17.*(t380-t392).*(-1.0027e-2);
t3267 = t17.*(t380-t392).*(-7.41e-4);
t3274 = t775.*(t380-t392);
t3278 = t798.*(t380-t392);
t3282 = t751.*(t380-t392);
t3287 = t906.*(t380-t392);
t3313 = -t3294;
t3331 = t178+t193+t487+t541;
t3333 = t384.*4.7121686402e-2;
t3336 = t391.*4.7121686402e-2;
t3341 = t8.*t3268;
t3342 = t8.*t3269;
t3343 = t9.*t3268;
t3347 = t16.*t3268;
t3348 = t16.*t3269;
t3349 = t17.*t3268;
t3366 = -t3328;
t3394 = -t3344;
t3422 = t384.*5.034347249e-2;
t3423 = -t3372;
t3425 = t391.*5.034347249e-2;
t3426 = -t3380;
t3436 = t389.*4.5305948634e-2;
t3438 = t390.*4.5305948634e-2;
t3443 = t395.*4.5305948634e-2;
t3445 = t397.*4.5305948634e-2;
t3456 = -t3410;
t3457 = -t3411;
t3458 = -t3412;
t3459 = -t3413;
t3460 = -t3418;
t3461 = t392.*1.7527158935e-2;
t3462 = t393.*1.7527158935e-2;
t3464 = t394.*1.7527158935e-2;
t3468 = t394.*3.127439544e-3;
t3469 = t395.*3.127439544e-3;
t3470 = t385.*7.735484874e-3;
t3471 = t386.*7.735484874e-3;
t3472 = t389.*7.735484874e-3;
t3476 = t381.*1.00241616695e-1;
t3478 = t394.*7.735484874e-3;
t3479 = t395.*7.735484874e-3;
t3481 = t397.*7.735484874e-3;
t3486 = t384.*1.00241616695e-1;
t3487 = t385.*1.00241616695e-1;
t3488 = t386.*1.00241616695e-1;
t3494 = t391.*1.00241616695e-1;
t3496 = t394.*1.00241616695e-1;
t3498 = -t3435;
t3501 = -t3437;
t3502 = t8.*t3330;
t3503 = t9.*t3330;
t3506 = -t3444;
t3507 = t16.*t3330;
t3508 = t17.*t3330;
t3513 = t384.*1.4653732538e-2;
t3517 = t391.*1.4653732538e-2;
t3519 = t545+t2113;
t3522 = t380.*2.3526756935e-2;
t3523 = t380.*1.7527158935e-2;
t3525 = t381.*1.7527158935e-2;
t3527 = t381.*3.127439544e-3;
t3528 = t384.*2.3526756935e-2;
t3530 = t388.*2.3526756935e-2;
t3532 = t385.*1.7527158935e-2;
t3533 = t386.*1.7527158935e-2;
t3535 = t388.*1.7527158935e-2;
t3537 = t381.*7.735484874e-3;
t3539 = t391.*2.3526756935e-2;
t3540 = t392.*2.3526756935e-2;
t3541 = t393.*2.3526756935e-2;
t3542 = t385.*3.127439544e-3;
t3543 = t386.*3.127439544e-3;
t3544 = t389.*3.127439544e-3;
t3546 = t390.*3.127439544e-3;
t3561 = t2106.*1.666555;
t3573 = t2106.*1.225946;
t3576 = t2113.*1.225946;
t3614 = -t3564;
t3637 = t565+t2106;
t3648 = t310+t529+t1415;
t3666 = t423.*4.5305948634e-2;
t3667 = t424.*4.5305948634e-2;
t3674 = t16.*t389.*3.40361334456e-4;
t3677 = -t3639;
t3678 = -t3640;
t3685 = -t3655;
t3700 = t424.*3.127439544e-3;
t3703 = t423.*7.735484874e-3;
t3725 = t16.*t395.*1.37607339936e-4;
t3729 = -t3710;
t3737 = -t3716;
t3764 = t469.*5.01208083475e-2;
t3766 = t8.*(t479+t534).*(-1.666555);
t3773 = t17.*t439.*4.5305948634e-2;
t3775 = t465.*1.17633784675e-2;
t3797 = t9.*t439.*4.5305948634e-2;
t3805 = -t3779;
t3808 = t439.*t2769;
t3814 = t439.*t2778;
t3825 = t503.*3.867742437e-3;
t3826 = t504.*3.867742437e-3;
t3827 = -t3798;
t3840 = t17.*t439.*(-7.735484874e-3);
t3853 = t505.*1.563719772e-3;
t3854 = t506.*1.563719772e-3;
t3858 = -t3828;
t3859 = -t3831;
t3862 = -t3834;
t3863 = -t3835;
t3887 = t9.*t3784;
t3890 = t17.*t3784;
t3896 = -t3847;
t3901 = t17.*(t71-t391).*(-4.5305948634e-2);
t3903 = -t3856;
t3924 = t9.*(t71-t391).*(-4.5305948634e-2);
t3925 = t17.*(t71-t391).*4.5305948634e-2;
t3932 = t8.*(t71-t391).*(-2.3526756935e-2);
t3934 = t8.*(t71-t391).*(-1.7527158935e-2);
t3936 = t9.*(t71-t391).*(-3.127439544e-3);
t3937 = t16.*(t71-t391).*(-1.7527158935e-2);
t3939 = t16.*(t71-t391).*(-3.127439544e-3);
t3940 = t17.*(t71-t391).*(-3.127439544e-3);
t3941 = t9.*(t71-t391).*(-7.735484874e-3);
t3943 = t16.*(t71-t391).*(-7.735484874e-3);
t3944 = t17.*(t71-t391).*(-7.735484874e-3);
t3945 = -t3918;
t3946 = -t3919;
t3950 = t16.*(t71-t391).*(-1.00241616695e-1);
t3951 = -t3926;
t3952 = -t3928;
t3963 = t8.*(t71-t391).*1.7527158935e-2;
t3965 = t2769.*(t71-t391);
t3966 = t16.*(t71-t391).*1.7527158935e-2;
t3967 = -t3938;
t3968 = t2771.*(t71-t391);
t3969 = -t3947;
t3973 = t2785.*(t71-t391);
t3979 = -t3955;
t3983 = -t3959;
t3988 = t3001.*(t71-t391);
t3996 = t2840.*(t71-t391);
t3997 = -t3974;
t4001 = t9.*t16.*(t71-t391).*(-3.40361334456e-4);
t4004 = -t3976;
t4007 = -t3986;
t4009 = t618.*(-4.5305948634e-2);
t4012 = -t3993;
t4015 = -t3998;
t4018 = t618.*(-3.127439544e-3);
t4025 = -t4008;
t4030 = t618.*4.5305948634e-2;
t4031 = -t4010;
t4035 = t456+t625+t764;
t4038 = t618.*3.127439544e-3;
t4040 = t16.*t17.*(t71-t391).*(-1.37607339936e-4);
t4048 = (t454.*t3173)./4.0;
t4050 = -t4037;
t4060 = -t4042;
t4061 = -t4043;
t4064 = t455+t762+t776;
t4067 = (t440.*t3219)./4.0;
t4113 = t3106.*(t71-t391).*(-1.0./4.0);
t4142 = t9.*(t208-t427).*(-3.867742437e-3);
t4146 = (t3106.*(t71-t391))./4.0;
t4153 = t440.*(t689-t740).*(-1.0./4.0);
t4168 = t9.*(t380-t392).*(-4.5305948634e-2);
t4169 = t17.*(t380-t392).*(-4.5305948634e-2);
t4173 = t17.*(t208-t427).*(-1.563719772e-3);
t4184 = t454.*(t733-t806).*(-1.0./4.0);
t4185 = t9.*(t380-t392).*(-3.127439544e-3);
t4191 = (t440.*(t689-t740))./4.0;
t4196 = t17.*(t380-t392).*(-7.735484874e-3);
t4201 = (t439.*t3304)./4.0;
t4202 = (t439.*t3307)./4.0;
t4204 = (t440.*(t1130-t16.*t17.*1.2516e-2))./4.0;
t4208 = t3239.*(t77-t390).*(-1.0./4.0);
t4213 = (t439.*t3317)./4.0;
t4217 = (t454.*(t733-t806))./4.0;
t4218 = t2769.*(t380-t392);
t4226 = t1462.*5.01208083475e-2;
t4229 = t3247.*(t71-t391).*(-1.0./4.0);
t4240 = (t3239.*(t77-t390))./4.0;
t4253 = -t4225;
t4257 = (t3247.*(t71-t391))./4.0;
t4258 = (t540.*t3239)./4.0;
t4263 = t3277.*(t71-t391).*(-1.0./4.0);
t4269 = t1475.*1.17633784675e-2;
t4275 = t3299.*(t71-t391).*(-1.0./4.0);
t4277 = (t439.*t3453)./4.0;
t4278 = t3286.*(t60-t394).*(-1.0./4.0);
t4284 = (t3277.*(t71-t391))./4.0;
t4285 = (t439.*t3441)./4.0;
t4287 = t3296.*(t60-t394).*(-1.0./4.0);
t4288 = -t4268;
t4295 = (t3299.*(t71-t391))./4.0;
t4304 = (t3296.*(t60-t394))./4.0;
t4309 = (t539.*t3286)./4.0;
t4310 = t16.*t3286.*(t71-t391).*(-1.0./4.0);
t4311 = (t539.*t3296)./4.0;
t4312 = t16.*t3296.*(t71-t391).*(-1.0./2.0);
t4316 = -t4308;
t4323 = t8.*t3307.*(t71-t391).*(-1.0./2.0);
t4336 = t384.*2.16405205209813e-3;
t4338 = -t4320;
t4343 = -t4326;
t4366 = t391.*4.600245517563106e-3;
t4367 = -t4345;
t4368 = -t4347;
t4369 = (t1355-t15.*t16.*1.158e-3).*(t71-t391).*(-1.0./4.0);
t4370 = -t4353;
t4373 = t397.*2.74179553204116e-4;
t4376 = t388.*5.187945860934245e-5;
t4379 = t392.*5.187945860934245e-5;
t4380 = t393.*5.187945860934245e-5;
t4387 = t3624.*(-7.35522e-1);
t4394 = t390.*8.36241330891889e-4;
t4397 = ((t1355-t15.*t16.*1.158e-3).*(t71-t391))./4.0;
t4399 = t380.*5.187945860934245e-5;
t4403 = -t4372;
t4406 = -t4375;
t4414 = t381.*4.67845486573025e-5;
t4416 = t385.*4.67845486573025e-5;
t4417 = t386.*4.67845486573025e-5;
t4419 = t394.*4.67845486573025e-5;
t4420 = t3624.*7.35522e-1;
t4421 = -t4388;
t4423 = -t4393;
t4425 = -t4396;
t4430 = t2113.*2.5171736245e-2;
t4434 = -t4413;
t4438 = t2106.*7.326866269e-3;
t4445 = -t4418;
t4453 = t574+t1459+t1482;
t4456 = t384.*5.897280115119475e-3;
t4462 = -t4437;
t4467 = -t4448;
t4469 = -t4452;
t4480 = -t4460;
t4481 = t381.*2.454825983680473e-3;
t4483 = t385.*2.454825983680473e-3;
t4484 = t386.*2.454825983680473e-3;
t4485 = t424.*8.36241330891889e-4;
t4488 = t394.*2.454825983680473e-3;
t4490 = t423.*2.74179553204116e-4;
t4523 = t3307.*(t380-t392).*(-1.0./4.0);
t4530 = -t4516;
t4536 = t4.*t4506;
t4540 = t4.*t4507;
t4552 = (t3307.*(t380-t392))./4.0;
t4571 = -t4556;
t4577 = t9.*t439.*8.36241330891889e-4;
t4579 = t8.*(t479+t534).*(-1.17633784675e-2);
t4592 = -t4542;
t4593 = t17.*t439.*2.74179553204116e-4;
t4611 = t367+t4252;
t4615 = t8.*(t479+t534).*1.17633784675e-2;
t4676 = t3219.*(t395+t9.*(t48-t349)).*(-1.0./4.0);
t4706 = (t3219.*(t395+t9.*(t48-t349)))./4.0;
t4719 = t9.*(t71-t391).*(-1.672482661783778e-3);
t4722 = t17.*(t71-t391).*(-5.48359106408232e-4);
